simulink model "untitled"  (R2019a)
settings: Solver=VariableStepAuto  StartTime=0.0  StopTime=30.0  RelTol=1e-3
undefined symbols (not defined in the file or in its folder): qJoints_init, robot, sigbuilder_block
libraries: SPART_Lib x2, dspinverses x2, robotmaniplib x1
settings Model: Creator=tori  LastModifiedBy=tori
settings DataIOCC: ReturnWorkspaceOutputs=off
settings DebuggingCC: ArithmeticOperatorsInVariantConditions=warning
settings SFSimCC: SimUseLocalCustomCode=off
settings RTWCC: RTWUseLocalCustomCode=off

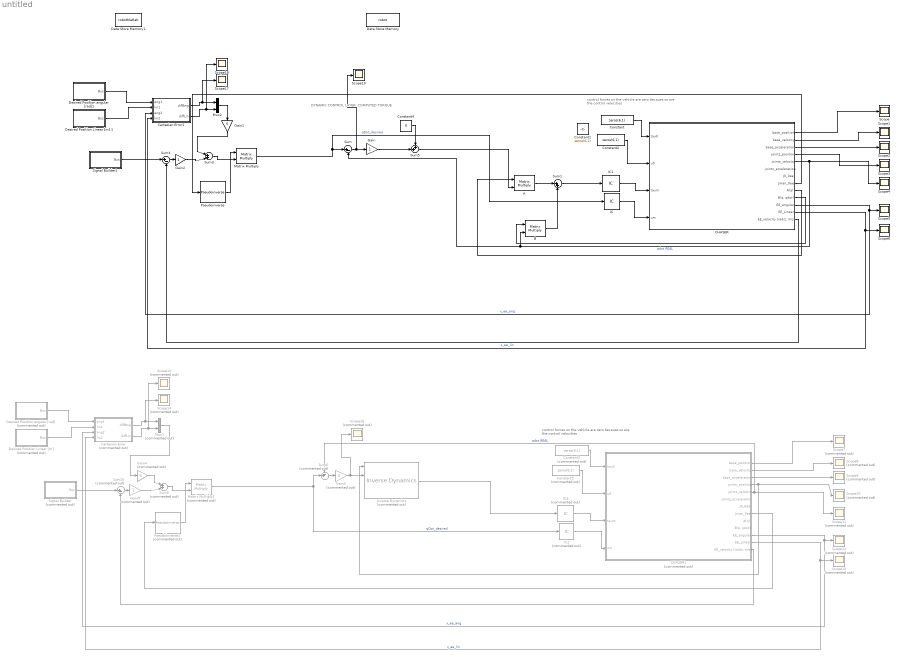
== system untitled ==
  note: DYNAMIC CONTROL LAYER: COMPUTED TORQUE
  note: control forces on the vehicle are zero
      | because so are the control velocities
  note: control forces on the vehicle are zero
      | because so are the control velocities
  A : Product  Multiplication=Matrix(*)
  B : Product  Multiplication=Matrix(*)
  CHASER : Subsystem
  CHASER1 : Subsystem  Commented=on
  Cartesian Error : MATLAB Function  Commented=on  TreatAsAtomicUnit=on
  Cartesian Error1 : MATLAB Function  TreatAsAtomicUnit=on
  Constant : Constant  Value=zeros(6,1)
  Constant1 : Constant  Value=zeros(6,1)
  Constant2 : Constant  Value=zeros(6,1)
  Constant3 : Constant  Commented=on  Value=zeros(6,1)
  Constant4 : Constant  Value=0
  Constant5 : Constant  Commented=on  Value=zeros(6,1)
  Data Store Memory : DataStoreMemory  DataStoreName=robot  ReadBeforeWriteMsg=warning  WriteAfterWriteMsg=warning  WriteAfterReadMsg=warning  ShowAdditionalParam=off
  Data Store Memory1 : DataStoreMemory  DataStoreName=robotMatlab  ReadBeforeWriteMsg=warning  WriteAfterWriteMsg=warning  WriteAfterReadMsg=warning  ShowAdditionalParam=off
  "Desired Position Linear [m] " : Subsystem  Tag=STV Subsys  Commented=on  LoadFcn=sigbuilder_block('load');  StartFcn=sigbuilder_block('start');  StopFcn=sigbuilder_block('stop');  ClipboardFcn=sigbuilder_block('clipboard');  mask(Sigbuilder block){tuvar=[0:10]}
      mask help: Simulink:masks:SigbuilderBlock_MD
      mask init:
      | if ~strcmp(get_param(bdroot(gcbh),'SimulationStatus'),'stopped') tuvar = sigbuilder_block('maskInit'); end
      settings: CopyFcn=sigbuilder_block('copy');  DeleteFcn=sigbuilder_block('delete');  ModelCloseFcn=sigbuilder_block('modelClose');  PreSaveFcn=sigbuilder_block('preSave');  PauseFcn=sigbuilder_block('pause');  ContinueFcn=sigbuilder_block('continue');  NameChangeFcn=sigbuilder_block('namechange');  OpenFcn=sigbuilder_block('open',[4.5 0 1432.5 645.75 ]);  CloseFcn=sigbuilder_block('close');
      mask Display: plot(0, 0, 100, 100,[2, 2, 32, 32, 2], [68, 8, 8, 68, 68],[32, 2], [38, 38], [32, 19, 2],[53, 60, 44], [32, 17, 17, 2],[16, 16, 31, 31]);txt = getActiveGroup(gcbh);text(2, 100, txt,'verticalAlignment', 'top');
  Desired Position Linear [m] 1 : Subsystem  Tag=STV Subsys  LoadFcn=sigbuilder_block('load');  StartFcn=sigbuilder_block('start');  StopFcn=sigbuilder_block('stop');  ClipboardFcn=sigbuilder_block('clipboard');  mask(Sigbuilder block){tuvar=[0:10]}
      mask help: Simulink:masks:SigbuilderBlock_MD
      mask init:
      | if ~strcmp(get_param(bdroot(gcbh),'SimulationStatus'),'stopped') tuvar = sigbuilder_block('maskInit'); end
      settings: CopyFcn=sigbuilder_block('copy');  DeleteFcn=sigbuilder_block('delete');  ModelCloseFcn=sigbuilder_block('modelClose');  PreSaveFcn=sigbuilder_block('preSave');  PauseFcn=sigbuilder_block('pause');  ContinueFcn=sigbuilder_block('continue');  NameChangeFcn=sigbuilder_block('namechange');  OpenFcn=sigbuilder_block('open',[4.5 0 1432.5 645.75 ]);  CloseFcn=sigbuilder_block('close');
      mask Display: plot(0, 0, 100, 100,[2, 2, 32, 32, 2], [68, 8, 8, 68, 68],[32, 2], [38, 38], [32, 19, 2],[53, 60, 44], [32, 17, 17, 2],[16, 16, 31, 31]);txt = getActiveGroup(gcbh);text(2, 100, txt,'verticalAlignment', 'top');
  Desired Position angular [rad] : Subsystem  Tag=STV Subsys  Commented=on  LoadFcn=sigbuilder_block('load');  StartFcn=sigbuilder_block('start');  StopFcn=sigbuilder_block('stop');  ClipboardFcn=sigbuilder_block('clipboard');  mask(Sigbuilder block){tuvar=[0:10]}
      mask help: Simulink:masks:SigbuilderBlock_MD
      mask init:
      | if ~strcmp(get_param(bdroot(gcbh),'SimulationStatus'),'stopped') tuvar = sigbuilder_block('maskInit'); end
      settings: CopyFcn=sigbuilder_block('copy');  DeleteFcn=sigbuilder_block('delete');  ModelCloseFcn=sigbuilder_block('modelClose');  PreSaveFcn=sigbuilder_block('preSave');  PauseFcn=sigbuilder_block('pause');  ContinueFcn=sigbuilder_block('continue');  NameChangeFcn=sigbuilder_block('namechange');  OpenFcn=sigbuilder_block('open',[0 0 1440 627 ]);  CloseFcn=sigbuilder_block('close');
      mask Display: plot(0, 0, 100, 100,[2, 2, 32, 32, 2], [68, 8, 8, 68, 68],[32, 2], [38, 38], [32, 19, 2],[53, 60, 44], [32, 17, 17, 2],[16, 16, 31, 31]);txt = getActiveGroup(gcbh);text(2, 100, txt,'verticalAlignment', 'top');
  Desired Position angular [rad]1 : Subsystem  Tag=STV Subsys  LoadFcn=sigbuilder_block('load');  StartFcn=sigbuilder_block('start');  StopFcn=sigbuilder_block('stop');  ClipboardFcn=sigbuilder_block('clipboard');  mask(Sigbuilder block){tuvar=[0:10]}
      mask help: Simulink:masks:SigbuilderBlock_MD
      mask init:
      | if ~strcmp(get_param(bdroot(gcbh),'SimulationStatus'),'stopped') tuvar = sigbuilder_block('maskInit'); end
      settings: CopyFcn=sigbuilder_block('copy');  DeleteFcn=sigbuilder_block('delete');  ModelCloseFcn=sigbuilder_block('modelClose');  PreSaveFcn=sigbuilder_block('preSave');  PauseFcn=sigbuilder_block('pause');  ContinueFcn=sigbuilder_block('continue');  NameChangeFcn=sigbuilder_block('namechange');  OpenFcn=sigbuilder_block('open',[0 0 1440 608.25 ]);  CloseFcn=sigbuilder_block('close');
      mask Display: plot(0, 0, 100, 100,[2, 2, 32, 32, 2], [68, 8, 8, 68, 68],[32, 2], [38, 38], [32, 19, 2],[53, 60, 44], [32, 17, 17, 2],[16, 16, 31, 31]);txt = getActiveGroup(gcbh);text(2, 100, txt,'verticalAlignment', 'top');
  Gain : Gain
  Gain1 : Gain  Gain=5
  Gain2 : Gain
  Gain3 : Gain  Commented=on  Gain=5
  Gain4 : Gain  Commented=on  Gain=3
  Gain5 : Gain  Commented=on
  IC : InitialCondition  Value=zeros(7,1)
  IC1 : InitialCondition  Value=zeros(7,1)
  IC2 : InitialCondition  Commented=on  Value=zeros(7,1)
  IC3 : InitialCondition  Commented=on  Value=zeros(7,1)
  Inverse Dynamics : robotmaniplib/Inverse Dynamics  Commented=on  RigidBodyTree=robotMatlab  SimulateUsing=Interpreted execution
      settings: SourceProductName=Robotics System Toolbox  SourceProductBaseCode=RO
  Matrix Multiply : Product  Multiplication=Matrix(*)
  Matrix Multiply1 : Product  Commented=on  Multiplication=Matrix(*)
  Mux1 : Mux  Commented=on  Inputs=2
  Mux2 : Mux  Inputs=2
  Pseudoinverse : dspinverses/Pseudoinverse  wanterr=off  SimulateUsing=Interpreted execution
      settings: SourceProductName=DSP System Toolbox  SourceProductBaseCode=DS
  Pseudoinverse1 : dspinverses/Pseudoinverse  Commented=on  wanterr=off  SimulateUsing=Interpreted execution
      settings: SourceProductName=DSP System Toolbox  SourceProductBaseCode=DS
  Scope{,1..6,17..19} (10 alike) : Scope
  Scope{7..16} (10 alike) : Scope  Commented=on
  Signal Builder : Subsystem  Tag=STV Subsys  Commented=on  LoadFcn=sigbuilder_block('load');  StartFcn=sigbuilder_block('start');  StopFcn=sigbuilder_block('stop');  ClipboardFcn=sigbuilder_block('clipboard');  mask(Sigbuilder block){tuvar=[0:10]}
      mask help: Simulink:masks:SigbuilderBlock_MD
      mask init:
      | if ~strcmp(get_param(bdroot(gcbh),'SimulationStatus'),'stopped') tuvar = sigbuilder_block('maskInit'); end
      settings: CopyFcn=sigbuilder_block('copy');  DeleteFcn=sigbuilder_block('delete');  ModelCloseFcn=sigbuilder_block('modelClose');  PreSaveFcn=sigbuilder_block('preSave');  PauseFcn=sigbuilder_block('pause');  ContinueFcn=sigbuilder_block('continue');  NameChangeFcn=sigbuilder_block('namechange');  OpenFcn=sigbuilder_block('open',[0.75 -1.5 735 724.5 ]);  CloseFcn=sigbuilder_block('close');
      mask Display: plot(0, 0, 100, 100,[2, 2, 32, 32, 2], [68, 8, 8, 68, 68],[32, 2], [38, 38], [32, 19, 2],[53, 60, 44], [32, 17, 17, 2],[16, 16, 31, 31]);txt = getActiveGroup(gcbh);text(2, 100, txt,'verticalAlignment', 'top');
  Signal Builder1 : Subsystem  Tag=STV Subsys  LoadFcn=sigbuilder_block('load');  StartFcn=sigbuilder_block('start');  StopFcn=sigbuilder_block('stop');  ClipboardFcn=sigbuilder_block('clipboard');  mask(Sigbuilder block){tuvar=[0:10]}
      mask help: Simulink:masks:SigbuilderBlock_MD
      mask init:
      | if ~strcmp(get_param(bdroot(gcbh),'SimulationStatus'),'stopped') tuvar = sigbuilder_block('maskInit'); end
      settings: CopyFcn=sigbuilder_block('copy');  DeleteFcn=sigbuilder_block('delete');  ModelCloseFcn=sigbuilder_block('modelClose');  PreSaveFcn=sigbuilder_block('preSave');  PauseFcn=sigbuilder_block('pause');  ContinueFcn=sigbuilder_block('continue');  NameChangeFcn=sigbuilder_block('namechange');  OpenFcn=sigbuilder_block('open',[8.25 0 720 724.5 ]);  CloseFcn=sigbuilder_block('close');
      mask Display: plot(0, 0, 100, 100,[2, 2, 32, 32, 2], [68, 8, 8, 68, 68],[32, 2], [38, 38], [32, 19, 2],[53, 60, 44], [32, 17, 17, 2],[16, 16, 31, 31]);txt = getActiveGroup(gcbh);text(2, 100, txt,'verticalAlignment', 'top');
  Sum : Sum  Inputs=|+-
  Sum1 : Sum  Inputs=|++
  Sum10 : Sum  Commented=on  Inputs=|+-
  Sum3 : Sum  Inputs=|++|
  Sum4 : Sum  Inputs=|+-
  Sum5 : Sum  Inputs=++|
  Sum6 : Sum  Commented=on  Inputs=-+|
  Sum9 : Sum  Commented=on  Inputs=|++|
  wires:
  Pseudoinverse/1 -> Matrix Multiply/1
  Gain/1 -> Sum5/2
  Matrix Multiply/1 -> IC/1, Sum/1  "qDot_desired"
  Sum/1 -> Scope19/1, Gain/1
  A/1 -> Sum1/1
  B/1 -> Sum1/2
  CHASER/5(joints_velocity) -> Scope4/1, Sum/2, B/2  "qdot REAL"
  CHASER/8(Jman_0ee) -> Pseudoinverse/1
  Sum1/1 -> IC1/1
  Constant/1 -> CHASER/1(tau0)
  Constant2/1 -> CHASER/2(u0)
  IC/1 -> CHASER/4(um)
  IC1/1 -> CHASER/3(taum)
  CHASER/10("B(q, qdot)") -> B/1
  CHASER/9(A(q)) -> A/1
  CHASER/1("base_position ") -> Scope/1
  CHASER/2("base_velocity ") -> Scope1/1
  CHASER/3(base_acceleration) -> Scope2/1
  CHASER/4(joints_position) -> Scope3/1
  CHASER/11("EE_angular ") -> Cartesian Error1/3(ang2), Scope5/1  "x_ee_ang"
  CHASER/12("EE_Linear ") -> Cartesian Error1/4(lin2), Scope6/1  "x_ee_lin"
  Sum3/1 -> Matrix Multiply/2
  Sum4/1 -> Gain2/1
  Gain2/1 -> Sum3/2
  Signal Builder1/1(Bus) -> Sum4/1
  CHASER/13(EE_velocity [rad/s; m/s]) -> Sum4/2
  Sum5/1 -> A/2
  Signal Builder/1(Bus) -> Sum10/1
  CHASER1/13(EE_velocity [rad/s; m/s]) -> Sum10/2
  CHASER1/12("EE_Linear ") -> Cartesian Error/4(lin2), Scope13/1  "x_ee_lin"
  Gain5/1 -> Sum9/2
  Matrix Multiply1/1 -> Sum6/2, IC2/1  "qDot_desired"
  CHASER1/3(base_acceleration) -> Scope9/1
  Gain4/1 -> Sum9/1
  CHASER1/4(joints_position) -> Inverse Dynamics/1, Scope10/1
  CHASER1/11("EE_angular ") -> Cartesian Error/3(ang2), Scope12/1  "x_ee_ang"
  Pseudoinverse1/1 -> Matrix Multiply1/1
  CHASER1/1("base_position ") -> Scope7/1
  Sum10/1 -> Gain5/1
  Sum9/1 -> Matrix Multiply1/2
  CHASER1/2("base_velocity ") -> Scope8/1
  Constant3/1 -> CHASER1/1(tau0)
  Constant5/1 -> CHASER1/2(u0)
  CHASER1/5(joints_velocity) -> Scope11/1, Sum6/1  "qdot REAL"
  CHASER1/8(Jman_0ee) -> Pseudoinverse1/1
  IC2/1 -> CHASER1/4(um)
  IC3/1 -> CHASER1/3(taum)
  Inverse Dynamics/1 -> IC3/1
  Desired Position angular [rad]/1(Bus) -> Cartesian Error/1(ang1)
  "Desired Position Linear [m] "/1(Bus) -> Cartesian Error/2(lin1)
  Cartesian Error/1(diffAng) -> Scope14/1, Mux1/1
  Cartesian Error/2(diffLin) -> Scope15/1, Mux1/2
  Mux1/1 -> Gain4/1
  Sum6/1 -> Gain3/1
  Gain3/1 -> Scope16/1, Inverse Dynamics/2
  Mux2/1 -> Gain1/1
  Cartesian Error1/2(diffLin) -> Scope18/1, Mux2/2
  Desired Position Linear [m] 1/1(Bus) -> Cartesian Error1/2(lin1)
  Cartesian Error1/1(diffAng) -> Scope17/1, Mux2/1
  Desired Position angular [rad]1/1(Bus) -> Cartesian Error1/1(ang1)
  Gain1/1 -> Sum3/1
  Constant4/1 -> Sum5/1

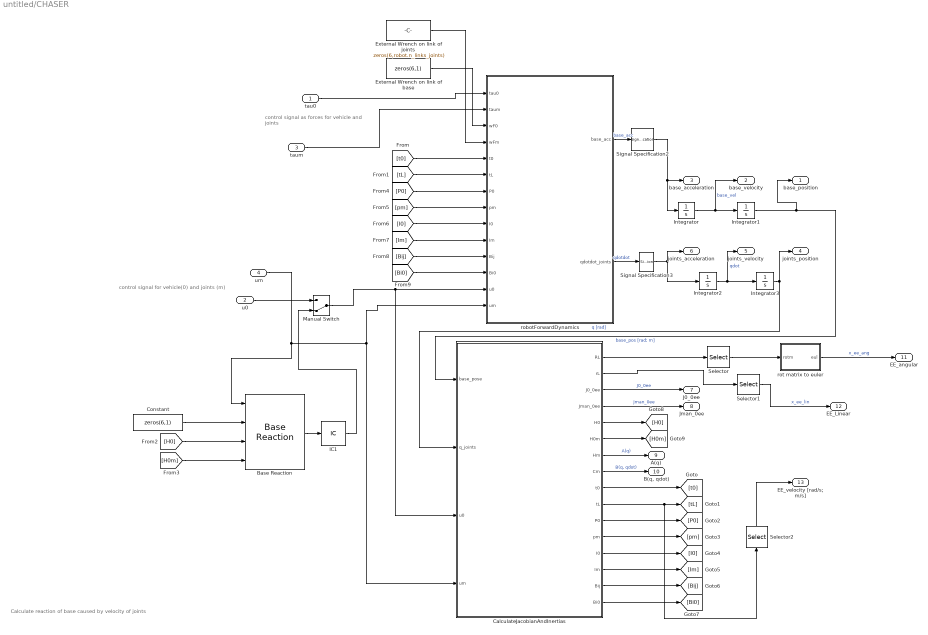
== system untitled/CHASER ==
  note: Calculate reaction of base caused by velocity of joints
  note: control signal as forces
      | for vehicle and joints
  note: control signal for vehicle(0)
      | and joints (m)
  tau0 : Inport
  u0 : Inport  Port=2
  taum : Inport  Port=3
  um : Inport  Port=4
  Base Reaction : SPART_Lib/Components/Base Reaction  SystemSampleTime=-1
  CalculateJacobianAndInertias : MATLAB Function  TreatAsAtomicUnit=on
  Constant : Constant  Value=zeros(6,1)
  "External Wrench on link of base " : Constant  Value=zeros(6,1)
  External Wrench on link of joints : Constant  Value=zeros(6,robot.n_links_joints)
  IC1 : InitialCondition  Value=zeros(6,1)
  Integrator : Integrator
  Integrator1 : Integrator
  Integrator2 : Integrator  InitialCondition=zeros(7,1)
  Integrator3 : Integrator  InitialCondition=qJoints_init  ContinuousStateAttributes='position'
  Manual Switch : ManualSwitch  CurrentSetting=0
  Selector : Selector  NumberOfDimensions=3  InputPortWidth=3  IndexOptions=Select all,Select all,Starting index (dialog)  Indices=[1 3],1,8  OutputSizes=1,1,1
  Selector1 : Selector  NumberOfDimensions=2  InputPortWidth=3  IndexOptions=Select all,Starting index (dialog)  Indices=[1 3],8  OutputSizes=1,1
  Selector2 : Selector  NumberOfDimensions=2  InputPortWidth=3  IndexOptions=Select all,Starting index (dialog)  Indices=[1 3],8  OutputSizes=1,1
  Signal Specification2 : SignalSpecification  Dimensions=[6 1]
  Signal Specification3 : SignalSpecification  Unit=rad  Dimensions=[7 1]
  "robotForwardDynamics " : MATLAB Function  TreatAsAtomicUnit=on
  "rot matrix to euler " : MATLAB Function  TreatAsAtomicUnit=on
  "base_position " : Outport
  "base_velocity " : Outport  Port=2
  base_acceleration : Outport  Port=3
  joints_position : Outport  Port=4
  joints_velocity : Outport  Port=5
  joints_acceleration : Outport  Port=6
  J0_0ee : Outport  Port=7
  Jman_0ee : Outport  Port=8
  A(q) : Outport  Port=9
  "B(q, qdot)" : Outport  Port=10
  "EE_angular " : Outport  Port=11
  "EE_Linear " : Outport  Port=12
  EE_velocity [rad/s; m/s] : Outport  Port=13
  wires:
  CalculateJacobianAndInertias/4(Jman_0ee) -> Jman_0ee/1  "Jman_0ee"
  CalculateJacobianAndInertias/7(Hm) -> A(q)/1  "A(q)"
  CalculateJacobianAndInertias/8(Cm) -> "B(q, qdot)"/1  "B(q, qdot)"
  "robotForwardDynamics "/1(base_acc) -> Signal Specification2/1  "base_acc"
  taum/1 -> "robotForwardDynamics "/2(taum)
  um/1 -> Base Reaction/1, "robotForwardDynamics "/14(um), CalculateJacobianAndInertias/4(um)
  tau0/1 -> "robotForwardDynamics "/1(tau0)
  CalculateJacobianAndInertias/3(J0_0ee) -> J0_0ee/1  "J0_0ee"
  Integrator/1 -> Integrator1/1, "base_velocity "/1  "base_vel"
  Integrator1/1 -> CalculateJacobianAndInertias/1(base_pose), "base_position "/1  "base_pos [rad; m]"
  Integrator2/1 -> joints_velocity/1, Integrator3/1  "qdot"
  Integrator3/1 -> CalculateJacobianAndInertias/2(q_joints), joints_position/1  "q [rad]"
  "robotForwardDynamics "/2(qdotdot_joints) -> Signal Specification3/1  "qdotdot"
  "External Wrench on link of base "/1 -> "robotForwardDynamics "/3(wF0)
  External Wrench on link of joints/1 -> "robotForwardDynamics "/4(wFm)
  [t0] -> "robotForwardDynamics "/5(t0)
  [tL] -> "robotForwardDynamics "/6(tL)
  [P0] -> "robotForwardDynamics "/7(P0)
  [pm] -> "robotForwardDynamics "/8(pm)
  [I0] -> "robotForwardDynamics "/9(I0)
  [Im] -> "robotForwardDynamics "/10(Im)
  [Bij] -> "robotForwardDynamics "/11(Bij)
  [Bi0] -> "robotForwardDynamics "/12(Bi0)
  CalculateJacobianAndInertias/9(t0) -> [t0]
  CalculateJacobianAndInertias/10(tL) -> Selector2/1, [tL]
  CalculateJacobianAndInertias/11(P0) -> [P0]
  CalculateJacobianAndInertias/12(pm) -> [pm]
  CalculateJacobianAndInertias/13(I0) -> [I0]
  CalculateJacobianAndInertias/14(Im) -> [Im]
  CalculateJacobianAndInertias/15(Bij) -> [Bij]
  CalculateJacobianAndInertias/16(Bi0) -> [Bi0]
  CalculateJacobianAndInertias/5(H0) -> [H0]
  CalculateJacobianAndInertias/6(H0m) -> [H0m]
  [H0] -> Base Reaction/3
  [H0m] -> Base Reaction/4
  CalculateJacobianAndInertias/1(RL) -> Selector/1
  CalculateJacobianAndInertias/2(rL) -> Selector1/1
  Selector/1 -> "rot matrix to euler "/1(rotm)
  "rot matrix to euler "/1(eul) -> "EE_angular "/1  "x_ee_ang"
  Selector1/1 -> "EE_Linear "/1  "x_ee_lin"
  Signal Specification3/1 -> Integrator2/1, joints_acceleration/1
  Signal Specification2/1 -> Integrator/1, base_acceleration/1
  Selector2/1 -> EE_velocity [rad/s; m/s]/1
  Constant/1 -> Base Reaction/2
  Base Reaction/1 -> IC1/1
  u0/1 -> Manual Switch/1
  Manual Switch/1 -> CalculateJacobianAndInertias/3(u0), "robotForwardDynamics "/13(u0)
  IC1/1 -> Manual Switch/2

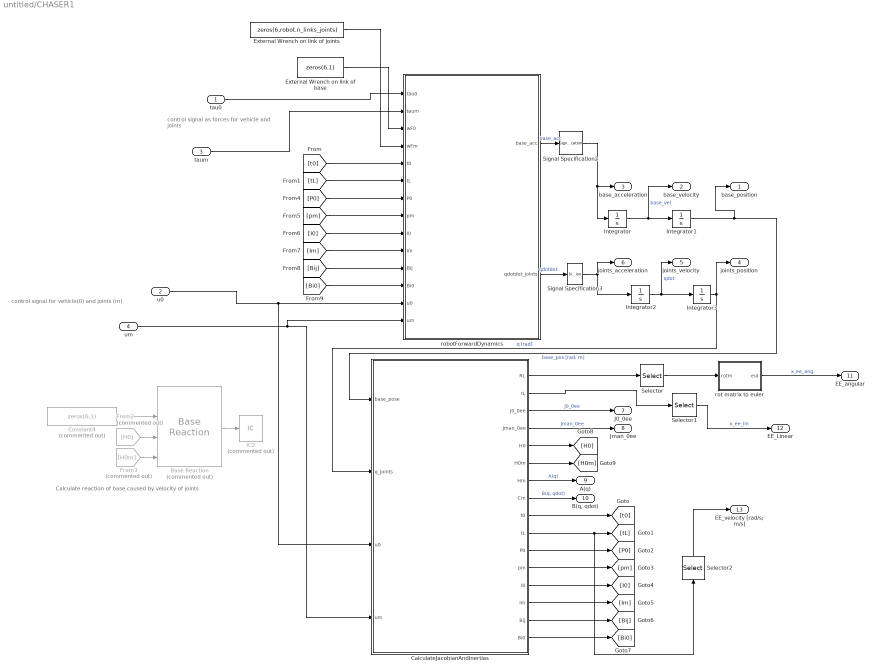
== system untitled/CHASER1 ==
  note: Calculate reaction of base caused by velocity of joints
  note: control signal as forces
      | for vehicle and joints
  note: control signal for vehicle(0)
      | and joints (m)
  tau0 : Inport
  u0 : Inport  Port=2
  taum : Inport  Port=3
  um : Inport  Port=4
  Base Reaction : SPART_Lib/Components/Base Reaction  Commented=on  SystemSampleTime=-1
  CalculateJacobianAndInertias : MATLAB Function  TreatAsAtomicUnit=on
  Constant4 : Constant  Commented=on  Value=zeros(6,1)
  "External Wrench on link of base " : Constant  Value=zeros(6,1)
  External Wrench on link of joints : Constant  Value=zeros(6,robot.n_links_joints)
  From2 : From  Commented=on  GotoTag=H0
  From3 : From  Commented=on  GotoTag=H0m
  IC2 : InitialCondition  Commented=on  Value=zeros(6,1)
  Integrator : Integrator
  Integrator1 : Integrator
  Integrator2 : Integrator  InitialCondition=zeros(7,1)
  Integrator3 : Integrator  InitialCondition=qJoints_init  ContinuousStateAttributes='position'
  Selector : Selector  NumberOfDimensions=3  InputPortWidth=3  IndexOptions=Select all,Select all,Starting index (dialog)  Indices=[1 3],1,8  OutputSizes=1,1,1
  Selector1 : Selector  NumberOfDimensions=2  InputPortWidth=3  IndexOptions=Select all,Starting index (dialog)  Indices=[1 3],8  OutputSizes=1,1
  Selector2 : Selector  NumberOfDimensions=2  InputPortWidth=3  IndexOptions=Select all,Starting index (dialog)  Indices=[1 3],8  OutputSizes=1,1
  Signal Specification2 : SignalSpecification  Dimensions=[6 1]
  Signal Specification3 : SignalSpecification  Unit=rad  Dimensions=[7 1]
  "robotForwardDynamics " : MATLAB Function  TreatAsAtomicUnit=on
  "rot matrix to euler " : MATLAB Function  TreatAsAtomicUnit=on
  "base_position " : Outport
  "base_velocity " : Outport  Port=2
  base_acceleration : Outport  Port=3
  joints_position : Outport  Port=4
  joints_velocity : Outport  Port=5
  joints_acceleration : Outport  Port=6
  J0_0ee : Outport  Port=7
  Jman_0ee : Outport  Port=8
  A(q) : Outport  Port=9
  "B(q, qdot)" : Outport  Port=10
  "EE_angular " : Outport  Port=11
  "EE_Linear " : Outport  Port=12
  EE_velocity [rad/s; m/s] : Outport  Port=13
  wires:
  CalculateJacobianAndInertias/4(Jman_0ee) -> Jman_0ee/1  "Jman_0ee"
  CalculateJacobianAndInertias/7(Hm) -> A(q)/1  "A(q)"
  CalculateJacobianAndInertias/8(Cm) -> "B(q, qdot)"/1  "B(q, qdot)"
  "robotForwardDynamics "/1(base_acc) -> Signal Specification2/1  "base_acc"
  taum/1 -> "robotForwardDynamics "/2(taum)
  um/1 -> CalculateJacobianAndInertias/4(um), "robotForwardDynamics "/14(um)
  tau0/1 -> "robotForwardDynamics "/1(tau0)
  CalculateJacobianAndInertias/3(J0_0ee) -> J0_0ee/1  "J0_0ee"
  Integrator/1 -> Integrator1/1, "base_velocity "/1  "base_vel"
  Integrator1/1 -> CalculateJacobianAndInertias/1(base_pose), "base_position "/1  "base_pos [rad; m]"
  Integrator2/1 -> joints_velocity/1, Integrator3/1  "qdot"
  Integrator3/1 -> CalculateJacobianAndInertias/2(q_joints), joints_position/1  "q [rad]"
  "robotForwardDynamics "/2(qdotdot_joints) -> Signal Specification3/1  "qdotdot"
  "External Wrench on link of base "/1 -> "robotForwardDynamics "/3(wF0)
  External Wrench on link of joints/1 -> "robotForwardDynamics "/4(wFm)
  [t0] -> "robotForwardDynamics "/5(t0)
  [tL] -> "robotForwardDynamics "/6(tL)
  [P0] -> "robotForwardDynamics "/7(P0)
  [pm] -> "robotForwardDynamics "/8(pm)
  [I0] -> "robotForwardDynamics "/9(I0)
  [Im] -> "robotForwardDynamics "/10(Im)
  [Bij] -> "robotForwardDynamics "/11(Bij)
  [Bi0] -> "robotForwardDynamics "/12(Bi0)
  CalculateJacobianAndInertias/9(t0) -> [t0]
  CalculateJacobianAndInertias/10(tL) -> Selector2/1, [tL]
  CalculateJacobianAndInertias/11(P0) -> [P0]
  CalculateJacobianAndInertias/12(pm) -> [pm]
  CalculateJacobianAndInertias/13(I0) -> [I0]
  CalculateJacobianAndInertias/14(Im) -> [Im]
  CalculateJacobianAndInertias/15(Bij) -> [Bij]
  CalculateJacobianAndInertias/16(Bi0) -> [Bi0]
  CalculateJacobianAndInertias/5(H0) -> [H0]
  CalculateJacobianAndInertias/6(H0m) -> [H0m]
  From2/1 -> Base Reaction/3
  From3/1 -> Base Reaction/4
  CalculateJacobianAndInertias/1(RL) -> Selector/1
  CalculateJacobianAndInertias/2(rL) -> Selector1/1
  Selector/1 -> "rot matrix to euler "/1(rotm)
  "rot matrix to euler "/1(eul) -> "EE_angular "/1  "x_ee_ang"
  Selector1/1 -> "EE_Linear "/1  "x_ee_lin"
  Signal Specification3/1 -> Integrator2/1, joints_acceleration/1
  Signal Specification2/1 -> Integrator/1, base_acceleration/1
  Selector2/1 -> EE_velocity [rad/s; m/s]/1
  Base Reaction/1 -> IC2/1
  Constant4/1 -> Base Reaction/2
  u0/1 -> CalculateJacobianAndInertias/3(u0), "robotForwardDynamics "/13(u0)

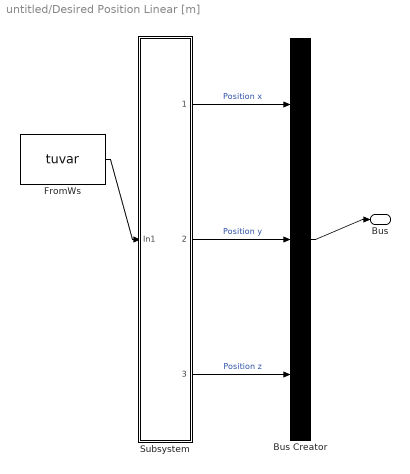
== system untitled/Desired Position Linear [m]  ==
  Bus Creator : BusCreator  Tag=Bus Creator  Inputs=3
  FromWs : FromWorkspace  Tag=STV FromWs  VariableName=tuvar  SampleTime=0
      SigBuilderData=|
      | common.afterFinalStr = 'Extrapolate'
      | common.sampleTime = 0
      | dataSet(1).timeRange = [0 30]
      | dataSet(1).name = 'Position'
      | dataSet(2).timeRange = [0 30]
      | dataSet(2).name = 'Position1'
      | sbobj.Groups(1).Name = 'Position'
      | sbobj.Groups(1).Signals(1).Name = 'Position x'
      | sbobj.Groups(1).Signals(1).XData = [0 0.15075 0.3015 0.45226 0.60301 0.75376 0.90451 1.0553 1.206 1.3568 1.5075 1.6583 1.809 1.9598 2.1105 2.2613 2.412 2.5628 2.7135 2.8643 3.015 3.1658 3.3165 3.4673 3.618 3.7688 3.9196 4.0703 4.2211 4.3718 4.5226 4.6733 4.8241 4.9748 5.1256 5.2763 5.4271 5.5778 5.7286 5.8793 6.0301 6.1808 6.3316 6.4823 6.6331 6.7838 6.9346 7.0853 7.2361 7.3869 7.5376 7.6884 7.8391 7.9899 8.1406 8.2914 8.4421 8.5929 8.7436 8.8944 9.0451 9.1959 9.3466 9.4974 9.6481 9.7989 9.9496 10.1 10.251 10.402 10.553 10.703 10.854 11.005 11.156 11.306 11.457 11.608 11.759 11.909 12.06 12.211 12.362 12.512 12.663 12.814 12.965 13.115 13.266 13.417 13.568 13.718 13.869 14.02 14.171 14.321 14.472 14.623 14.774 14.924 15.075 15.226 15.377 15.527 15.678 15.829 15.98 16.13 16.281 16.432 16.583 16.733 16.884 17.035 17.186 17.336 17.487 17.638 17.789 17.939 18.09 18.241 18.392 18.543 18.693 18.844 18.995 19.146 19.296 19.447 19.598 19.749 19.899 20.05 20.201 20.352 20.502 20.653 20.804 20.955 21.105 21.256 21.407 21.558 21.708 21.859 22.01 22.161 22.311 22.462 22.613 22.764 22.914 23.065 23.216 23.367 23.517 23.668 23.819 23.97 24.12 24.271 24.422 24.573 24.723 24.874 25.025 25.176 25.326 25.477 25.628 25.779 25.929 26.08 26.231 26.382 26.532 26.683 26.834 26.985 27.135 27.286 27.437 27.588 27.738 27.889 28.04 28.191 28.341 28.492 28.643 28.794 28.944 29.095 29.246 29.397 29.547 29.698 29.849 30]
      | sbobj.Groups(1).Signals(1).YData = [4.1497 4.1496 4.1494 4.149 4.1484 4.1474 4.1461 4.1445 4.1427 4.1405 4.1382 4.1356 4.1328 4.1298 4.1268 4.1236 4.1203 4.117 4.1136 4.1102 4.1067 4.1033 4.0999 4.0964 4.093 4.0896 4.0862 4.0828 4.0794 4.076 4.0726 4.0692 4.0657 4.0622 4.0586 4.055 4.0513 4.0476 4.0438 4.0399 4.0359 4.0318 4.0277 4.0235 4.0192 4.0148 4.0104 4.0058 4.0012 3.9966 3.9918 3.987 3.9822 3.9773 3.9723 3.9674 3.9623 3.9573 3.9522 3.9471 3.9419 3.9368 3.9316 3.9265 3.9213 3.9161 3.9109 3.9056 3.9004 3.8951 3.8899 3.8846 3.8793 3.8739 3.8686 3.8632 3.8578 3.8523 3.8468 3.8413 3.8357 3.83 3.8243 3.8186 3.8128 3.8069 3.801 3.795 3.7889 3.7828 3.7766 3.7704 3.7641 3.7578 3.7513 3.7449 3.7384 3.7318 3.7252 3.7186 3.7119 3.7052 3.6984 3.6917 3.6849 3.678 3.6712 3.6644 3.6575 3.6506 3.6438 3.6369 3.63 3.6231 3.6163 3.6094 3.6025 3.5956 3.5887 3.5818 3.5749 3.5679 3.561 3.554 3.547 3.54 3.533 3.5259 3.5188 3.5116 3.5044 3.4972 3.4899 3.4825 3.4751 3.4676 3.4601 3.4525 3.4449 3.4371 3.4294 3.4216 3.4137 3.4058 3.3978 3.3898 3.3818 3.3737 3.3656 3.3575 3.3494 3.3412 3.3331 3.325 3.3169 3.3088 3.3007 3.2927 3.2847 3.2767 3.2687 3.2608 3.253 3.2451 3.2373 3.2295 3.2217 3.2139 3.2061 3.1983 3.1905 3.1826 3.1747 3.1668 3.1587 3.1506 3.1424 3.1341 3.1258 3.1173 3.1087 3.1 3.0912 3.0824 3.0736 3.0647 3.0559 3.0471 3.0385 3.0301 3.022 3.0143 3.0071 3.0004 2.9944 2.9892 2.9849 2.9817 2.9797 2.979]
      | sbobj.Groups(1).Signals(2).Name = 'Position y'
      | sbobj.Groups(1).Signals(2).XData = [0 0.15075 0.3015 0.45226 0.60301 0.75376 0.90451 1.0553 1.206 1.3568 1.5075 1.6583 1.809 1.9598 2.1105 2.2613 2.412 2.5628 2.7135 2.8643 3.015 3.1658 3.3165 3.4673 3.618 3.7688 3.9196 4.0703 4.2211 4.3718 4.5226 4.6733 4.8241 4.9748 5.1256 5.2763 5.4271 5.5778 5.7286 5.8793 6.0301 6.1808 6.3316 6.4823 6.6331 6.7838 6.9346 7.0853 7.2361 7.3869 7.5376 7.6884 7.8391 7.9899 8.1406 8.2914 8.4421 8.5929 8.7436 8.8944 9.0451 9.1959 9.3466 9.4974 9.6481 9.7989 9.9496 10.1 10.251 10.402 10.553 10.703 10.854 11.005 11.156 11.306 11.457 11.608 11.759 11.909 12.06 12.211 12.362 12.512 12.663 12.814 12.965 13.115 13.266 13.417 13.568 13.718 13.869 14.02 14.171 14.321 14.472 14.623 14.774 14.924 15.075 15.226 15.377 15.527 15.678 15.829 15.98 16.13 16.281 16.432 16.583 16.733 16.884 17.035 17.186 17.336 17.487 17.638 17.789 17.939 18.09 18.241 18.392 18.543 18.693 18.844 18.995 19.146 19.296 19.447 19.598 19.749 19.899 20.05 20.201 20.352 20.502 20.653 20.804 20.955 21.105 21.256 21.407 21.558 21.708 21.859 22.01 22.161 22.311 22.462 22.613 22.764 22.914 23.065 23.216 23.367 23.517 23.668 23.819 23.97 24.12 24.271 24.422 24.573 24.723 24.874 25.025 25.176 25.326 25.477 25.628 25.779 25.929 26.08 26.231 26.382 26.532 26.683 26.834 26.985 27.135 27.286 27.437 27.588 27.738 27.889 28.04 28.191 28.341 28.492 28.643 28.794 28.944 29.095 29.246 29.397 29.547 29.698 29.849 30]
      | sbobj.Groups(1).Signals(2).YData = [0.16804 0.16819 0.16861 0.16923 0.17001 0.17093 0.17195 0.17305 0.1742 0.17541 0.17666 0.17793 0.17923 0.18054 0.18188 0.18322 0.18458 0.18595 0.18732 0.1887 0.19008 0.19147 0.19286 0.19425 0.19564 0.19703 0.19842 0.19981 0.2012 0.20259 0.20397 0.20535 0.20673 0.2081 0.20948 0.21085 0.21222 0.21359 0.21496 0.21632 0.21769 0.21906 0.22044 0.22181 0.22319 0.22458 0.22597 0.22738 0.22879 0.23021 0.23164 0.23309 0.23455 0.23602 0.23751 0.23902 0.24054 0.24207 0.24363 0.2452 0.24679 0.24839 0.25002 0.25166 0.25331 0.25498 0.25667 0.25837 0.26008 0.2618 0.26354 0.26528 0.26703 0.26879 0.27056 0.27233 0.27411 0.27589 0.27767 0.27945 0.28123 0.283 0.28478 0.28655 0.28832 0.29008 0.29184 0.2936 0.29535 0.2971 0.29884 0.30058 0.30231 0.30404 0.30577 0.30749 0.30922 0.31095 0.31268 0.31441 0.31614 0.31789 0.31963 0.32139 0.32316 0.32494 0.32673 0.32854 0.33036 0.3322 0.33405 0.33592 0.33782 0.33973 0.34166 0.34361 0.34558 0.34758 0.34959 0.35162 0.35367 0.35574 0.35782 0.35992 0.36204 0.36416 0.3663 0.36845 0.3706 0.37276 0.37493 0.37709 0.37926 0.38142 0.38358 0.38573 0.38788 0.39002 0.39214 0.39426 0.39636 0.39845 0.40052 0.40259 0.40464 0.40667 0.4087 0.41071 0.41272 0.41471 0.41671 0.4187 0.42069 0.42268 0.42468 0.42668 0.4287 0.43074 0.43279 0.43487 0.43697 0.43911 0.44128 0.44348 0.44572 0.44801 0.45033 0.4527 0.45511 0.45757 0.46008 0.46262 0.46521 0.46784 0.47051 0.47321 0.47593 0.47868 0.48145 0.48422 0.48701 0.48978 0.49255 0.49529 0.49801 0.50068 0.5033 0.50586 0.50835 0.51074 0.51304 0.51521 0.51725 0.51912 0.52082 0.5223 0.52353 0.52447 0.52508 0.52529]
      | sbobj.Groups(1).Signals(3).Name = 'Position z'
      | sbobj.Groups(1).Signals(3).XData = [0 0.15075 0.3015 0.45226 0.60301 0.75376 0.90451 1.0553 1.206 1.3568 1.5075 1.6583 1.809 1.9598 2.1105 2.2613 2.412 2.5628 2.7135 2.8643 3.015 3.1658 3.3165 3.4673 3.618 3.7688 3.9196 4.0703 4.2211 4.3718 4.5226 4.6733 4.8241 4.9748 5.1256 5.2763 5.4271 5.5778 5.7286 5.8793 6.0301 6.1808 6.3316 6.4823 6.6331 6.7838 6.9346 7.0853 7.2361 7.3869 7.5376 7.6884 7.8391 7.9899 8.1406 8.2914 8.4421 8.5929 8.7436 8.8944 9.0451 9.1959 9.3466 9.4974 9.6481 9.7989 9.9496 10.1 10.251 10.402 10.553 10.703 10.854 11.005 11.156 11.306 11.457 11.608 11.759 11.909 12.06 12.211 12.362 12.512 12.663 12.814 12.965 13.115 13.266 13.417 13.568 13.718 13.869 14.02 14.171 14.321 14.472 14.623 14.774 14.924 15.075 15.226 15.377 15.527 15.678 15.829 15.98 16.13 16.281 16.432 16.583 16.733 16.884 17.035 17.186 17.336 17.487 17.638 17.789 17.939 18.09 18.241 18.392 18.543 18.693 18.844 18.995 19.146 19.296 19.447 19.598 19.749 19.899 20.05 20.201 20.352 20.502 20.653 20.804 20.955 21.105 21.256 21.407 21.558 21.708 21.859 22.01 22.161 22.311 22.462 22.613 22.764 22.914 23.065 23.216 23.367 23.517 23.668 23.819 23.97 24.12 24.271 24.422 24.573 24.723 24.874 25.025 25.176 25.326 25.477 25.628 25.779 25.929 26.08 26.231 26.382 26.532 26.683 26.834 26.985 27.135 27.286 27.437 27.588 27.738 27.889 28.04 28.191 28.341 28.492 28.643 28.794 28.944 29.095 29.246 29.397 29.547 29.698 29.849 30]
      | sbobj.Groups(1).Signals(3).YData = [1.735 1.7355 1.737 1.7396 1.7435 1.7485 1.7547 1.7619 1.7701 1.7791 1.7889 1.7992 1.81 1.8211 1.8325 1.844 1.8557 1.8673 1.8789 1.8904 1.9017 1.9129 1.924 1.9348 1.9455 1.9559 1.9662 1.9764 1.9863 1.9962 2.0059 2.0155 2.0251 2.0346 2.044 2.0535 2.0629 2.0723 2.0817 2.0912 2.1007 2.1102 2.1198 2.1294 2.1391 2.1488 2.1585 2.1682 2.178 2.1878 2.1976 2.2074 2.2171 2.2269 2.2366 2.2463 2.2559 2.2655 2.275 2.2845 2.2939 2.3032 2.3124 2.3215 2.3306 2.3395 2.3484 2.3572 2.3659 2.3746 2.3831 2.3916 2.4 2.4083 2.4166 2.4248 2.4329 2.441 2.4491 2.4571 2.4651 2.4731 2.481 2.4889 2.4968 2.5047 2.5126 2.5204 2.5283 2.5361 2.5439 2.5518 2.5596 2.5674 2.5751 2.5829 2.5906 2.5983 2.606 2.6137 2.6213 2.6289 2.6364 2.6439 2.6513 2.6587 2.666 2.6733 2.6804 2.6876 2.6946 2.7016 2.7085 2.7153 2.722 2.7287 2.7353 2.7418 2.7483 2.7546 2.7609 2.7672 2.7733 2.7794 2.7855 2.7915 2.7974 2.8033 2.8091 2.815 2.8207 2.8265 2.8322 2.8379 2.8435 2.8492 2.8548 2.8604 2.866 2.8715 2.8771 2.8826 2.8881 2.8936 2.899 2.9045 2.9099 2.9152 2.9206 2.9258 2.9311 2.9362 2.9414 2.9464 2.9514 2.9563 2.9611 2.9659 2.9705 2.9751 2.9796 2.984 2.9883 2.9925 2.9966 3.0006 3.0045 3.0084 3.0122 3.0159 3.0195 3.0231 3.0266 3.0301 3.0336 3.037 3.0404 3.0438 3.0472 3.0506 3.054 3.0573 3.0607 3.0641 3.0674 3.0707 3.0739 3.0771 3.0802 3.0832 3.086 3.0887 3.0911 3.0934 3.0953 3.097 3.0983 3.0992 3.0998 3.1]
      | sbobj.Groups(1).TimeRange = [0 30]
      | sbobj.Groups(2).Name = 'Position1'
      | sbobj.Groups(2).Signals(1).Name = 'Position x'
      | sbobj.Groups(2).Signals(1).XData = [0 0.15075 0.3015 0.45226 0.60301 0.75376 0.90451 1.0553 1.206 1.3568 1.5075 1.6583 1.809 1.9598 2.1105 2.2613 2.412 2.5628 2.7135 2.8643 3.015 3.1658 3.3165 3.4673 3.618 3.7688 3.9196 4.0703 4.2211 4.3718 4.5226 4.6733 4.8241 4.9748 5.1256 5.2763 5.4271 5.5778 5.7286 5.8793 6.0301 6.1808 6.3316 6.4823 6.6331 6.7838 6.9346 7.0853 7.2361 7.3869 7.5376 7.6884 7.8391 7.9899 8.1406 8.2914 8.4421 8.5929 8.7436 8.8944 9.0451 9.1959 9.3466 9.4974 9.6481 9.7989 9.9496 10.1 10.251 10.402 10.553 10.703 10.854 11.005 11.156 11.306 11.457 11.608 11.759 11.909 12.06 12.211 12.362 12.512 12.663 12.814 12.965 13.115 13.266 13.417 13.568 13.718 13.869 14.02 14.171 14.321 14.472 14.623 14.774 14.924 15.075 15.226 15.377 15.527 15.678 15.829 15.98 16.13 16.281 16.432 16.583 16.733 16.884 17.035 17.186 17.336 17.487 17.638 17.789 17.939 18.09 18.241 18.392 18.543 18.693 18.844 18.995 19.146 19.296 19.447 19.598 19.749 19.899 20.05 20.201 20.352 20.502 20.653 20.804 20.955 21.105 21.256 21.407 21.558 21.708 21.859 22.01 22.161 22.311 22.462 22.613 22.764 22.914 23.065 23.216 23.367 23.517 23.668 23.819 23.97 24.12 24.271 24.422 24.573 24.723 24.874 25.025 25.176 25.326 25.477 25.628 25.779 25.929 26.08 26.231 26.382 26.532 26.683 26.834 26.985 27.135 27.286 27.437 27.588 27.738 27.889 28.04 28.191 28.341 28.492 28.643 28.794 28.944 29.095 29.246 29.397 29.547 29.698 29.849 30]
      | sbobj.Groups(2).Signals(1).YData = [4.1497 4.1496 4.1494 4.149 4.1484 4.1474 4.1461 4.1445 4.1427 4.1405 4.1382 4.1356 4.1328 4.1298 4.1268 4.1236 4.1203 4.117 4.1136 4.1102 4.1067 4.1033 4.0999 4.0964 4.093 4.0896 4.0862 4.0828 4.0794 4.076 4.0726 4.0692 4.0657 4.0622 4.0586 4.055 4.0513 4.0476 4.0438 4.0399 4.0359 4.0318 4.0277 4.0235 4.0192 4.0148 4.0104 4.0058 4.0012 3.9966 3.9918 3.987 3.9822 3.9773 3.9723 3.9674 3.9623 3.9573 3.9522 3.9471 3.9419 3.9368 3.9316 3.9265 3.9213 3.9161 3.9109 3.9056 3.9004 3.8951 3.8899 3.8846 3.8793 3.8739 3.8686 3.8632 3.8578 3.8523 3.8468 3.8413 3.8357 3.83 3.8243 3.8186 3.8128 3.8069 3.801 3.795 3.7889 3.7828 3.7766 3.7704 3.7641 3.7578 3.7513 3.7449 3.7384 3.7318 3.7252 3.7186 3.7119 3.7052 3.6984 3.6917 3.6849 3.678 3.6712 3.6644 3.6575 3.6506 3.6438 3.6369 3.63 3.6231 3.6163 3.6094 3.6025 3.5956 3.5887 3.5818 3.5749 3.5679 3.561 3.554 3.547 3.54 3.533 3.5259 3.5188 3.5116 3.5044 3.4972 3.4899 3.4825 3.4751 3.4676 3.4601 3.4525 3.4449 3.4371 3.4294 3.4216 3.4137 3.4058 3.3978 3.3898 3.3818 3.3737 3.3656 3.3575 3.3494 3.3412 3.3331 3.325 3.3169 3.3088 3.3007 3.2927 3.2847 3.2767 3.2687 3.2608 3.253 3.2451 3.2373 3.2295 3.2217 3.2139 3.2061 3.1983 3.1905 3.1826 3.1747 3.1668 3.1587 3.1506 3.1424 3.1341 3.1258 3.1173 3.1087 3.1 3.0912 3.0824 3.0736 3.0647 3.0559 3.0471 3.0385 3.0301 3.022 3.0143 3.0071 3.0004 2.9944 2.9892 2.9849 2.9817 2.9797 2.979]
      | sbobj.Groups(2).Signals(2).Name = 'Position y'
      | sbobj.Groups(2).Signals(2).XData = [0 0.15075 0.3015 0.45226 0.60301 0.75376 0.90451 1.0553 1.206 1.3568 1.5075 1.6583 1.809 1.9598 2.1105 2.2613 2.412 2.5628 2.7135 2.8643 3.015 3.1658 3.3165 3.4673 3.618 3.7688 3.9196 4.0703 4.2211 4.3718 4.5226 4.6733 4.8241 4.9748 5.1256 5.2763 5.4271 5.5778 5.7286 5.8793 6.0301 6.1808 6.3316 6.4823 6.6331 6.7838 6.9346 7.0853 7.2361 7.3869 7.5376 7.6884 7.8391 7.9899 8.1406 8.2914 8.4421 8.5929 8.7436 8.8944 9.0451 9.1959 9.3466 9.4974 9.6481 9.7989 9.9496 10.1 10.251 10.402 10.553 10.703 10.854 11.005 11.156 11.306 11.457 11.608 11.759 11.909 12.06 12.211 12.362 12.512 12.663 12.814 12.965 13.115 13.266 13.417 13.568 13.718 13.869 14.02 14.171 14.321 14.472 14.623 14.774 14.924 15.075 15.226 15.377 15.527 15.678 15.829 15.98 16.13 16.281 16.432 16.583 16.733 16.884 17.035 17.186 17.336 17.487 17.638 17.789 17.939 18.09 18.241 18.392 18.543 18.693 18.844 18.995 19.146 19.296 19.447 19.598 19.749 19.899 20.05 20.201 20.352 20.502 20.653 20.804 20.955 21.105 21.256 21.407 21.558 21.708 21.859 22.01 22.161 22.311 22.462 22.613 22.764 22.914 23.065 23.216 23.367 23.517 23.668 23.819 23.97 24.12 24.271 24.422 24.573 24.723 24.874 25.025 25.176 25.326 25.477 25.628 25.779 25.929 26.08 26.231 26.382 26.532 26.683 26.834 26.985 27.135 27.286 27.437 27.588 27.738 27.889 28.04 28.191 28.341 28.492 28.643 28.794 28.944 29.095 29.246 29.397 29.547 29.698 29.849 30]
      | sbobj.Groups(2).Signals(2).YData = [0.16804 0.16819 0.16861 0.16923 0.17001 0.17093 0.17195 0.17305 0.1742 0.17541 0.17666 0.17793 0.17923 0.18054 0.18188 0.18322 0.18458 0.18595 0.18732 0.1887 0.19008 0.19147 0.19286 0.19425 0.19564 0.19703 0.19842 0.19981 0.2012 0.20259 0.20397 0.20535 0.20673 0.2081 0.20948 0.21085 0.21222 0.21359 0.21496 0.21632 0.21769 0.21906 0.22044 0.22181 0.22319 0.22458 0.22597 0.22738 0.22879 0.23021 0.23164 0.23309 0.23455 0.23602 0.23751 0.23902 0.24054 0.24207 0.24363 0.2452 0.24679 0.24839 0.25002 0.25166 0.25331 0.25498 0.25667 0.25837 0.26008 0.2618 0.26354 0.26528 0.26703 0.26879 0.27056 0.27233 0.27411 0.27589 0.27767 0.27945 0.28123 0.283 0.28478 0.28655 0.28832 0.29008 0.29184 0.2936 0.29535 0.2971 0.29884 0.30058 0.30231 0.30404 0.30577 0.30749 0.30922 0.31095 0.31268 0.31441 0.31614 0.31789 0.31963 0.32139 0.32316 0.32494 0.32673 0.32854 0.33036 0.3322 0.33405 0.33592 0.33782 0.33973 0.34166 0.34361 0.34558 0.34758 0.34959 0.35162 0.35367 0.35574 0.35782 0.35992 0.36204 0.36416 0.3663 0.36845 0.3706 0.37276 0.37493 0.37709 0.37926 0.38142 0.38358 0.38573 0.38788 0.39002 0.39214 0.39426 0.39636 0.39845 0.40052 0.40259 0.40464 0.40667 0.4087 0.41071 0.41272 0.41471 0.41671 0.4187 0.42069 0.42268 0.42468 0.42668 0.4287 0.43074 0.43279 0.43487 0.43697 0.43911 0.44128 0.44348 0.44572 0.44801 0.45033 0.4527 0.45511 0.45757 0.46008 0.46262 0.46521 0.46784 0.47051 0.47321 0.47593 0.47868 0.48145 0.48422 0.48701 0.48978 0.49255 0.49529 0.49801 0.50068 0.5033 0.50586 0.50835 0.51074 0.51304 0.51521 0.51725 0.51912 0.52082 0.5223 0.52353 0.52447 0.52508 0.52529]
      | sbobj.Groups(2).Signals(3).Name = 'Position z'
      | sbobj.Groups(2).Signals(3).XData = [0 0.15075 0.3015 0.45226 0.60301 0.75376 0.90451 1.0553 1.206 1.3568 1.5075 1.6583 1.809 1.9598 2.1105 2.2613 2.412 2.5628 2.7135 2.8643 3.015 3.1658 3.3165 3.4673 3.618 3.7688 3.9196 4.0703 4.2211 4.3718 4.5226 4.6733 4.8241 4.9748 5.1256 5.2763 5.4271 5.5778 5.7286 5.8793 6.0301 6.1808 6.3316 6.4823 6.6331 6.7838 6.9346 7.0853 7.2361 7.3869 7.5376 7.6884 7.8391 7.9899 8.1406 8.2914 8.4421 8.5929 8.7436 8.8944 9.0451 9.1959 9.3466 9.4974 9.6481 9.7989 9.9496 10.1 10.251 10.402 10.553 10.703 10.854 11.005 11.156 11.306 11.457 11.608 11.759 11.909 12.06 12.211 12.362 12.512 12.663 12.814 12.965 13.115 13.266 13.417 13.568 13.718 13.869 14.02 14.171 14.321 14.472 14.623 14.774 14.924 15.075 15.226 15.377 15.527 15.678 15.829 15.98 16.13 16.281 16.432 16.583 16.733 16.884 17.035 17.186 17.336 17.487 17.638 17.789 17.939 18.09 18.241 18.392 18.543 18.693 18.844 18.995 19.146 19.296 19.447 19.598 19.749 19.899 20.05 20.201 20.352 20.502 20.653 20.804 20.955 21.105 21.256 21.407 21.558 21.708 21.859 22.01 22.161 22.311 22.462 22.613 22.764 22.914 23.065 23.216 23.367 23.517 23.668 23.819 23.97 24.12 24.271 24.422 24.573 24.723 24.874 25.025 25.176 25.326 25.477 25.628 25.779 25.929 26.08 26.231 26.382 26.532 26.683 26.834 26.985 27.135 27.286 27.437 27.588 27.738 27.889 28.04 28.191 28.341 28.492 28.643 28.794 28.944 29.095 29.246 29.397 29.547 29.698 29.849 30]
      | sbobj.Groups(2).Signals(3).YData = [1.735 1.7355 1.737 1.7396 1.7435 1.7485 1.7547 1.7619 1.7701 1.7791 1.7889 1.7992 1.81 1.8211 1.8325 1.844 1.8557 1.8673 1.8789 1.8904 1.9017 1.9129 1.924 1.9348 1.9455 1.9559 1.9662 1.9764 1.9863 1.9962 2.0059 2.0155 2.0251 2.0346 2.044 2.0535 2.0629 2.0723 2.0817 2.0912 2.1007 2.1102 2.1198 2.1294 2.1391 2.1488 2.1585 2.1682 2.178 2.1878 2.1976 2.2074 2.2171 2.2269 2.2366 2.2463 2.2559 2.2655 2.275 2.2845 2.2939 2.3032 2.3124 2.3215 2.3306 2.3395 2.3484 2.3572 2.3659 2.3746 2.3831 2.3916 2.4 2.4083 2.4166 2.4248 2.4329 2.441 2.4491 2.4571 2.4651 2.4731 2.481 2.4889 2.4968 2.5047 2.5126 2.5204 2.5283 2.5361 2.5439 2.5518 2.5596 2.5674 2.5751 2.5829 2.5906 2.5983 2.606 2.6137 2.6213 2.6289 2.6364 2.6439 2.6513 2.6587 2.666 2.6733 2.6804 2.6876 2.6946 2.7016 2.7085 2.7153 2.722 2.7287 2.7353 2.7418 2.7483 2.7546 2.7609 2.7672 2.7733 2.7794 2.7855 2.7915 2.7974 2.8033 2.8091 2.815 2.8207 2.8265 2.8322 2.8379 2.8435 2.8492 2.8548 2.8604 2.866 2.8715 2.8771 2.8826 2.8881 2.8936 2.899 2.9045 2.9099 2.9152 2.9206 2.9258 2.9311 2.9362 2.9414 2.9464 2.9514 2.9563 2.9611 2.9659 2.9705 2.9751 2.9796 2.984 2.9883 2.9925 2.9966 3.0006 3.0045 3.0084 3.0122 3.0159 3.0195 3.0231 3.0266 3.0301 3.0336 3.037 3.0404 3.0438 3.0472 3.0506 3.054 3.0573 3.0607 3.0641 3.0674 3.0707 3.0739 3.0771 3.0802 3.0832 3.086 3.0887 3.0911 3.0934 3.0953 3.097 3.0983 3.0992 3.0998 3.1]
      | sbobj.Groups(2).TimeRange = [0 30]
  Subsystem : Subsystem
  Bus : Outport
  wires:
  FromWs/1 -> Subsystem/1(In1)
  Bus Creator/1 -> Bus/1
  Subsystem/1(Position x) -> Bus Creator/1  "Position x"
  Subsystem/2(Position y) -> Bus Creator/2  "Position y"
  Subsystem/3(Position z) -> Bus Creator/3  "Position z"

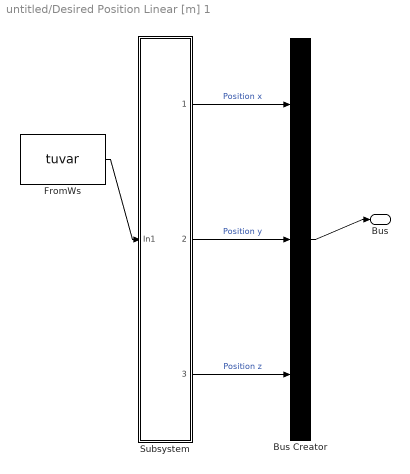
== system untitled/Desired Position Linear [m] 1 ==
  Bus Creator : BusCreator  Tag=Bus Creator  Inputs=3
  FromWs : FromWorkspace  Tag=STV FromWs  VariableName=tuvar  SampleTime=0
      SigBuilderData=|
      | common.afterFinalStr = 'Extrapolate'
      | common.sampleTime = 0
      | dataSet(1).timeRange = [0 30]
      | dataSet(1).name = 'Position'
      | dataSet(2).timeRange = [0 30]
      | dataSet(2).name = 'Position1'
      | sbobj.Groups(1).Name = 'Position'
      | sbobj.Groups(1).Signals(1).Name = 'Position x'
      | sbobj.Groups(1).Signals(1).XData = [0 0.15075 0.3015 0.45226 0.60301 0.75376 0.90451 1.0553 1.206 1.3568 1.5075 1.6583 1.809 1.9598 2.1105 2.2613 2.412 2.5628 2.7135 2.8643 3.015 3.1658 3.3165 3.4673 3.618 3.7688 3.9196 4.0703 4.2211 4.3718 4.5226 4.6733 4.8241 4.9748 5.1256 5.2763 5.4271 5.5778 5.7286 5.8793 6.0301 6.1808 6.3316 6.4823 6.6331 6.7838 6.9346 7.0853 7.2361 7.3869 7.5376 7.6884 7.8391 7.9899 8.1406 8.2914 8.4421 8.5929 8.7436 8.8944 9.0451 9.1959 9.3466 9.4974 9.6481 9.7989 9.9496 10.1 10.251 10.402 10.553 10.703 10.854 11.005 11.156 11.306 11.457 11.608 11.759 11.909 12.06 12.211 12.362 12.512 12.663 12.814 12.965 13.115 13.266 13.417 13.568 13.718 13.869 14.02 14.171 14.321 14.472 14.623 14.774 14.924 15.075 15.226 15.377 15.527 15.678 15.829 15.98 16.13 16.281 16.432 16.583 16.733 16.884 17.035 17.186 17.336 17.487 17.638 17.789 17.939 18.09 18.241 18.392 18.543 18.693 18.844 18.995 19.146 19.296 19.447 19.598 19.749 19.899 20.05 20.201 20.352 20.502 20.653 20.804 20.955 21.105 21.256 21.407 21.558 21.708 21.859 22.01 22.161 22.311 22.462 22.613 22.764 22.914 23.065 23.216 23.367 23.517 23.668 23.819 23.97 24.12 24.271 24.422 24.573 24.723 24.874 25.025 25.176 25.326 25.477 25.628 25.779 25.929 26.08 26.231 26.382 26.532 26.683 26.834 26.985 27.135 27.286 27.437 27.588 27.738 27.889 28.04 28.191 28.341 28.492 28.643 28.794 28.944 29.095 29.246 29.397 29.547 29.698 29.849 30]
      | sbobj.Groups(1).Signals(1).YData = [4.1497 4.1496 4.1494 4.149 4.1484 4.1474 4.1461 4.1445 4.1427 4.1405 4.1382 4.1356 4.1328 4.1298 4.1268 4.1236 4.1203 4.117 4.1136 4.1102 4.1067 4.1033 4.0999 4.0964 4.093 4.0896 4.0862 4.0828 4.0794 4.076 4.0726 4.0692 4.0657 4.0622 4.0586 4.055 4.0513 4.0476 4.0438 4.0399 4.0359 4.0318 4.0277 4.0235 4.0192 4.0148 4.0104 4.0058 4.0012 3.9966 3.9918 3.987 3.9822 3.9773 3.9723 3.9674 3.9623 3.9573 3.9522 3.9471 3.9419 3.9368 3.9316 3.9265 3.9213 3.9161 3.9109 3.9056 3.9004 3.8951 3.8899 3.8846 3.8793 3.8739 3.8686 3.8632 3.8578 3.8523 3.8468 3.8413 3.8357 3.83 3.8243 3.8186 3.8128 3.8069 3.801 3.795 3.7889 3.7828 3.7766 3.7704 3.7641 3.7578 3.7513 3.7449 3.7384 3.7318 3.7252 3.7186 3.7119 3.7052 3.6984 3.6917 3.6849 3.678 3.6712 3.6644 3.6575 3.6506 3.6438 3.6369 3.63 3.6231 3.6163 3.6094 3.6025 3.5956 3.5887 3.5818 3.5749 3.5679 3.561 3.554 3.547 3.54 3.533 3.5259 3.5188 3.5116 3.5044 3.4972 3.4899 3.4825 3.4751 3.4676 3.4601 3.4525 3.4449 3.4371 3.4294 3.4216 3.4137 3.4058 3.3978 3.3898 3.3818 3.3737 3.3656 3.3575 3.3494 3.3412 3.3331 3.325 3.3169 3.3088 3.3007 3.2927 3.2847 3.2767 3.2687 3.2608 3.253 3.2451 3.2373 3.2295 3.2217 3.2139 3.2061 3.1983 3.1905 3.1826 3.1747 3.1668 3.1587 3.1506 3.1424 3.1341 3.1258 3.1173 3.1087 3.1 3.0912 3.0824 3.0736 3.0647 3.0559 3.0471 3.0385 3.0301 3.022 3.0143 3.0071 3.0004 2.9944 2.9892 2.9849 2.9817 2.9797 2.979]
      | sbobj.Groups(1).Signals(2).Name = 'Position y'
      | sbobj.Groups(1).Signals(2).XData = [0 0.15075 0.3015 0.45226 0.60301 0.75376 0.90451 1.0553 1.206 1.3568 1.5075 1.6583 1.809 1.9598 2.1105 2.2613 2.412 2.5628 2.7135 2.8643 3.015 3.1658 3.3165 3.4673 3.618 3.7688 3.9196 4.0703 4.2211 4.3718 4.5226 4.6733 4.8241 4.9748 5.1256 5.2763 5.4271 5.5778 5.7286 5.8793 6.0301 6.1808 6.3316 6.4823 6.6331 6.7838 6.9346 7.0853 7.2361 7.3869 7.5376 7.6884 7.8391 7.9899 8.1406 8.2914 8.4421 8.5929 8.7436 8.8944 9.0451 9.1959 9.3466 9.4974 9.6481 9.7989 9.9496 10.1 10.251 10.402 10.553 10.703 10.854 11.005 11.156 11.306 11.457 11.608 11.759 11.909 12.06 12.211 12.362 12.512 12.663 12.814 12.965 13.115 13.266 13.417 13.568 13.718 13.869 14.02 14.171 14.321 14.472 14.623 14.774 14.924 15.075 15.226 15.377 15.527 15.678 15.829 15.98 16.13 16.281 16.432 16.583 16.733 16.884 17.035 17.186 17.336 17.487 17.638 17.789 17.939 18.09 18.241 18.392 18.543 18.693 18.844 18.995 19.146 19.296 19.447 19.598 19.749 19.899 20.05 20.201 20.352 20.502 20.653 20.804 20.955 21.105 21.256 21.407 21.558 21.708 21.859 22.01 22.161 22.311 22.462 22.613 22.764 22.914 23.065 23.216 23.367 23.517 23.668 23.819 23.97 24.12 24.271 24.422 24.573 24.723 24.874 25.025 25.176 25.326 25.477 25.628 25.779 25.929 26.08 26.231 26.382 26.532 26.683 26.834 26.985 27.135 27.286 27.437 27.588 27.738 27.889 28.04 28.191 28.341 28.492 28.643 28.794 28.944 29.095 29.246 29.397 29.547 29.698 29.849 30]
      | sbobj.Groups(1).Signals(2).YData = [0.16804 0.16819 0.16861 0.16923 0.17001 0.17093 0.17195 0.17305 0.1742 0.17541 0.17666 0.17793 0.17923 0.18054 0.18188 0.18322 0.18458 0.18595 0.18732 0.1887 0.19008 0.19147 0.19286 0.19425 0.19564 0.19703 0.19842 0.19981 0.2012 0.20259 0.20397 0.20535 0.20673 0.2081 0.20948 0.21085 0.21222 0.21359 0.21496 0.21632 0.21769 0.21906 0.22044 0.22181 0.22319 0.22458 0.22597 0.22738 0.22879 0.23021 0.23164 0.23309 0.23455 0.23602 0.23751 0.23902 0.24054 0.24207 0.24363 0.2452 0.24679 0.24839 0.25002 0.25166 0.25331 0.25498 0.25667 0.25837 0.26008 0.2618 0.26354 0.26528 0.26703 0.26879 0.27056 0.27233 0.27411 0.27589 0.27767 0.27945 0.28123 0.283 0.28478 0.28655 0.28832 0.29008 0.29184 0.2936 0.29535 0.2971 0.29884 0.30058 0.30231 0.30404 0.30577 0.30749 0.30922 0.31095 0.31268 0.31441 0.31614 0.31789 0.31963 0.32139 0.32316 0.32494 0.32673 0.32854 0.33036 0.3322 0.33405 0.33592 0.33782 0.33973 0.34166 0.34361 0.34558 0.34758 0.34959 0.35162 0.35367 0.35574 0.35782 0.35992 0.36204 0.36416 0.3663 0.36845 0.3706 0.37276 0.37493 0.37709 0.37926 0.38142 0.38358 0.38573 0.38788 0.39002 0.39214 0.39426 0.39636 0.39845 0.40052 0.40259 0.40464 0.40667 0.4087 0.41071 0.41272 0.41471 0.41671 0.4187 0.42069 0.42268 0.42468 0.42668 0.4287 0.43074 0.43279 0.43487 0.43697 0.43911 0.44128 0.44348 0.44572 0.44801 0.45033 0.4527 0.45511 0.45757 0.46008 0.46262 0.46521 0.46784 0.47051 0.47321 0.47593 0.47868 0.48145 0.48422 0.48701 0.48978 0.49255 0.49529 0.49801 0.50068 0.5033 0.50586 0.50835 0.51074 0.51304 0.51521 0.51725 0.51912 0.52082 0.5223 0.52353 0.52447 0.52508 0.52529]
      | sbobj.Groups(1).Signals(3).Name = 'Position z'
      | sbobj.Groups(1).Signals(3).XData = [0 0.15075 0.3015 0.45226 0.60301 0.75376 0.90451 1.0553 1.206 1.3568 1.5075 1.6583 1.809 1.9598 2.1105 2.2613 2.412 2.5628 2.7135 2.8643 3.015 3.1658 3.3165 3.4673 3.618 3.7688 3.9196 4.0703 4.2211 4.3718 4.5226 4.6733 4.8241 4.9748 5.1256 5.2763 5.4271 5.5778 5.7286 5.8793 6.0301 6.1808 6.3316 6.4823 6.6331 6.7838 6.9346 7.0853 7.2361 7.3869 7.5376 7.6884 7.8391 7.9899 8.1406 8.2914 8.4421 8.5929 8.7436 8.8944 9.0451 9.1959 9.3466 9.4974 9.6481 9.7989 9.9496 10.1 10.251 10.402 10.553 10.703 10.854 11.005 11.156 11.306 11.457 11.608 11.759 11.909 12.06 12.211 12.362 12.512 12.663 12.814 12.965 13.115 13.266 13.417 13.568 13.718 13.869 14.02 14.171 14.321 14.472 14.623 14.774 14.924 15.075 15.226 15.377 15.527 15.678 15.829 15.98 16.13 16.281 16.432 16.583 16.733 16.884 17.035 17.186 17.336 17.487 17.638 17.789 17.939 18.09 18.241 18.392 18.543 18.693 18.844 18.995 19.146 19.296 19.447 19.598 19.749 19.899 20.05 20.201 20.352 20.502 20.653 20.804 20.955 21.105 21.256 21.407 21.558 21.708 21.859 22.01 22.161 22.311 22.462 22.613 22.764 22.914 23.065 23.216 23.367 23.517 23.668 23.819 23.97 24.12 24.271 24.422 24.573 24.723 24.874 25.025 25.176 25.326 25.477 25.628 25.779 25.929 26.08 26.231 26.382 26.532 26.683 26.834 26.985 27.135 27.286 27.437 27.588 27.738 27.889 28.04 28.191 28.341 28.492 28.643 28.794 28.944 29.095 29.246 29.397 29.547 29.698 29.849 30]
      | sbobj.Groups(1).Signals(3).YData = [1.735 1.7355 1.737 1.7396 1.7435 1.7485 1.7547 1.7619 1.7701 1.7791 1.7889 1.7992 1.81 1.8211 1.8325 1.844 1.8557 1.8673 1.8789 1.8904 1.9017 1.9129 1.924 1.9348 1.9455 1.9559 1.9662 1.9764 1.9863 1.9962 2.0059 2.0155 2.0251 2.0346 2.044 2.0535 2.0629 2.0723 2.0817 2.0912 2.1007 2.1102 2.1198 2.1294 2.1391 2.1488 2.1585 2.1682 2.178 2.1878 2.1976 2.2074 2.2171 2.2269 2.2366 2.2463 2.2559 2.2655 2.275 2.2845 2.2939 2.3032 2.3124 2.3215 2.3306 2.3395 2.3484 2.3572 2.3659 2.3746 2.3831 2.3916 2.4 2.4083 2.4166 2.4248 2.4329 2.441 2.4491 2.4571 2.4651 2.4731 2.481 2.4889 2.4968 2.5047 2.5126 2.5204 2.5283 2.5361 2.5439 2.5518 2.5596 2.5674 2.5751 2.5829 2.5906 2.5983 2.606 2.6137 2.6213 2.6289 2.6364 2.6439 2.6513 2.6587 2.666 2.6733 2.6804 2.6876 2.6946 2.7016 2.7085 2.7153 2.722 2.7287 2.7353 2.7418 2.7483 2.7546 2.7609 2.7672 2.7733 2.7794 2.7855 2.7915 2.7974 2.8033 2.8091 2.815 2.8207 2.8265 2.8322 2.8379 2.8435 2.8492 2.8548 2.8604 2.866 2.8715 2.8771 2.8826 2.8881 2.8936 2.899 2.9045 2.9099 2.9152 2.9206 2.9258 2.9311 2.9362 2.9414 2.9464 2.9514 2.9563 2.9611 2.9659 2.9705 2.9751 2.9796 2.984 2.9883 2.9925 2.9966 3.0006 3.0045 3.0084 3.0122 3.0159 3.0195 3.0231 3.0266 3.0301 3.0336 3.037 3.0404 3.0438 3.0472 3.0506 3.054 3.0573 3.0607 3.0641 3.0674 3.0707 3.0739 3.0771 3.0802 3.0832 3.086 3.0887 3.0911 3.0934 3.0953 3.097 3.0983 3.0992 3.0998 3.1]
      | sbobj.Groups(1).TimeRange = [0 30]
      | sbobj.Groups(2).Name = 'Position1'
      | sbobj.Groups(2).Signals(1).Name = 'Position x'
      | sbobj.Groups(2).Signals(1).XData = [0 0.15075 0.3015 0.45226 0.60301 0.75376 0.90451 1.0553 1.206 1.3568 1.5075 1.6583 1.809 1.9598 2.1105 2.2613 2.412 2.5628 2.7135 2.8643 3.015 3.1658 3.3165 3.4673 3.618 3.7688 3.9196 4.0703 4.2211 4.3718 4.5226 4.6733 4.8241 4.9748 5.1256 5.2763 5.4271 5.5778 5.7286 5.8793 6.0301 6.1808 6.3316 6.4823 6.6331 6.7838 6.9346 7.0853 7.2361 7.3869 7.5376 7.6884 7.8391 7.9899 8.1406 8.2914 8.4421 8.5929 8.7436 8.8944 9.0451 9.1959 9.3466 9.4974 9.6481 9.7989 9.9496 10.1 10.251 10.402 10.553 10.703 10.854 11.005 11.156 11.306 11.457 11.608 11.759 11.909 12.06 12.211 12.362 12.512 12.663 12.814 12.965 13.115 13.266 13.417 13.568 13.718 13.869 14.02 14.171 14.321 14.472 14.623 14.774 14.924 15.075 15.226 15.377 15.527 15.678 15.829 15.98 16.13 16.281 16.432 16.583 16.733 16.884 17.035 17.186 17.336 17.487 17.638 17.789 17.939 18.09 18.241 18.392 18.543 18.693 18.844 18.995 19.146 19.296 19.447 19.598 19.749 19.899 20.05 20.201 20.352 20.502 20.653 20.804 20.955 21.105 21.256 21.407 21.558 21.708 21.859 22.01 22.161 22.311 22.462 22.613 22.764 22.914 23.065 23.216 23.367 23.517 23.668 23.819 23.97 24.12 24.271 24.422 24.573 24.723 24.874 25.025 25.176 25.326 25.477 25.628 25.779 25.929 26.08 26.231 26.382 26.532 26.683 26.834 26.985 27.135 27.286 27.437 27.588 27.738 27.889 28.04 28.191 28.341 28.492 28.643 28.794 28.944 29.095 29.246 29.397 29.547 29.698 29.849 30]
      | sbobj.Groups(2).Signals(1).YData = [4.1497 4.1496 4.1494 4.149 4.1484 4.1474 4.1461 4.1445 4.1427 4.1405 4.1382 4.1356 4.1328 4.1298 4.1268 4.1236 4.1203 4.117 4.1136 4.1102 4.1067 4.1033 4.0999 4.0964 4.093 4.0896 4.0862 4.0828 4.0794 4.076 4.0726 4.0692 4.0657 4.0622 4.0586 4.055 4.0513 4.0476 4.0438 4.0399 4.0359 4.0318 4.0277 4.0235 4.0192 4.0148 4.0104 4.0058 4.0012 3.9966 3.9918 3.987 3.9822 3.9773 3.9723 3.9674 3.9623 3.9573 3.9522 3.9471 3.9419 3.9368 3.9316 3.9265 3.9213 3.9161 3.9109 3.9056 3.9004 3.8951 3.8899 3.8846 3.8793 3.8739 3.8686 3.8632 3.8578 3.8523 3.8468 3.8413 3.8357 3.83 3.8243 3.8186 3.8128 3.8069 3.801 3.795 3.7889 3.7828 3.7766 3.7704 3.7641 3.7578 3.7513 3.7449 3.7384 3.7318 3.7252 3.7186 3.7119 3.7052 3.6984 3.6917 3.6849 3.678 3.6712 3.6644 3.6575 3.6506 3.6438 3.6369 3.63 3.6231 3.6163 3.6094 3.6025 3.5956 3.5887 3.5818 3.5749 3.5679 3.561 3.554 3.547 3.54 3.533 3.5259 3.5188 3.5116 3.5044 3.4972 3.4899 3.4825 3.4751 3.4676 3.4601 3.4525 3.4449 3.4371 3.4294 3.4216 3.4137 3.4058 3.3978 3.3898 3.3818 3.3737 3.3656 3.3575 3.3494 3.3412 3.3331 3.325 3.3169 3.3088 3.3007 3.2927 3.2847 3.2767 3.2687 3.2608 3.253 3.2451 3.2373 3.2295 3.2217 3.2139 3.2061 3.1983 3.1905 3.1826 3.1747 3.1668 3.1587 3.1506 3.1424 3.1341 3.1258 3.1173 3.1087 3.1 3.0912 3.0824 3.0736 3.0647 3.0559 3.0471 3.0385 3.0301 3.022 3.0143 3.0071 3.0004 2.9944 2.9892 2.9849 2.9817 2.9797 2.979]
      | sbobj.Groups(2).Signals(2).Name = 'Position y'
      | sbobj.Groups(2).Signals(2).XData = [0 0.15075 0.3015 0.45226 0.60301 0.75376 0.90451 1.0553 1.206 1.3568 1.5075 1.6583 1.809 1.9598 2.1105 2.2613 2.412 2.5628 2.7135 2.8643 3.015 3.1658 3.3165 3.4673 3.618 3.7688 3.9196 4.0703 4.2211 4.3718 4.5226 4.6733 4.8241 4.9748 5.1256 5.2763 5.4271 5.5778 5.7286 5.8793 6.0301 6.1808 6.3316 6.4823 6.6331 6.7838 6.9346 7.0853 7.2361 7.3869 7.5376 7.6884 7.8391 7.9899 8.1406 8.2914 8.4421 8.5929 8.7436 8.8944 9.0451 9.1959 9.3466 9.4974 9.6481 9.7989 9.9496 10.1 10.251 10.402 10.553 10.703 10.854 11.005 11.156 11.306 11.457 11.608 11.759 11.909 12.06 12.211 12.362 12.512 12.663 12.814 12.965 13.115 13.266 13.417 13.568 13.718 13.869 14.02 14.171 14.321 14.472 14.623 14.774 14.924 15.075 15.226 15.377 15.527 15.678 15.829 15.98 16.13 16.281 16.432 16.583 16.733 16.884 17.035 17.186 17.336 17.487 17.638 17.789 17.939 18.09 18.241 18.392 18.543 18.693 18.844 18.995 19.146 19.296 19.447 19.598 19.749 19.899 20.05 20.201 20.352 20.502 20.653 20.804 20.955 21.105 21.256 21.407 21.558 21.708 21.859 22.01 22.161 22.311 22.462 22.613 22.764 22.914 23.065 23.216 23.367 23.517 23.668 23.819 23.97 24.12 24.271 24.422 24.573 24.723 24.874 25.025 25.176 25.326 25.477 25.628 25.779 25.929 26.08 26.231 26.382 26.532 26.683 26.834 26.985 27.135 27.286 27.437 27.588 27.738 27.889 28.04 28.191 28.341 28.492 28.643 28.794 28.944 29.095 29.246 29.397 29.547 29.698 29.849 30]
      | sbobj.Groups(2).Signals(2).YData = [0.16804 0.16819 0.16861 0.16923 0.17001 0.17093 0.17195 0.17305 0.1742 0.17541 0.17666 0.17793 0.17923 0.18054 0.18188 0.18322 0.18458 0.18595 0.18732 0.1887 0.19008 0.19147 0.19286 0.19425 0.19564 0.19703 0.19842 0.19981 0.2012 0.20259 0.20397 0.20535 0.20673 0.2081 0.20948 0.21085 0.21222 0.21359 0.21496 0.21632 0.21769 0.21906 0.22044 0.22181 0.22319 0.22458 0.22597 0.22738 0.22879 0.23021 0.23164 0.23309 0.23455 0.23602 0.23751 0.23902 0.24054 0.24207 0.24363 0.2452 0.24679 0.24839 0.25002 0.25166 0.25331 0.25498 0.25667 0.25837 0.26008 0.2618 0.26354 0.26528 0.26703 0.26879 0.27056 0.27233 0.27411 0.27589 0.27767 0.27945 0.28123 0.283 0.28478 0.28655 0.28832 0.29008 0.29184 0.2936 0.29535 0.2971 0.29884 0.30058 0.30231 0.30404 0.30577 0.30749 0.30922 0.31095 0.31268 0.31441 0.31614 0.31789 0.31963 0.32139 0.32316 0.32494 0.32673 0.32854 0.33036 0.3322 0.33405 0.33592 0.33782 0.33973 0.34166 0.34361 0.34558 0.34758 0.34959 0.35162 0.35367 0.35574 0.35782 0.35992 0.36204 0.36416 0.3663 0.36845 0.3706 0.37276 0.37493 0.37709 0.37926 0.38142 0.38358 0.38573 0.38788 0.39002 0.39214 0.39426 0.39636 0.39845 0.40052 0.40259 0.40464 0.40667 0.4087 0.41071 0.41272 0.41471 0.41671 0.4187 0.42069 0.42268 0.42468 0.42668 0.4287 0.43074 0.43279 0.43487 0.43697 0.43911 0.44128 0.44348 0.44572 0.44801 0.45033 0.4527 0.45511 0.45757 0.46008 0.46262 0.46521 0.46784 0.47051 0.47321 0.47593 0.47868 0.48145 0.48422 0.48701 0.48978 0.49255 0.49529 0.49801 0.50068 0.5033 0.50586 0.50835 0.51074 0.51304 0.51521 0.51725 0.51912 0.52082 0.5223 0.52353 0.52447 0.52508 0.52529]
      | sbobj.Groups(2).Signals(3).Name = 'Position z'
      | sbobj.Groups(2).Signals(3).XData = [0 0.15075 0.3015 0.45226 0.60301 0.75376 0.90451 1.0553 1.206 1.3568 1.5075 1.6583 1.809 1.9598 2.1105 2.2613 2.412 2.5628 2.7135 2.8643 3.015 3.1658 3.3165 3.4673 3.618 3.7688 3.9196 4.0703 4.2211 4.3718 4.5226 4.6733 4.8241 4.9748 5.1256 5.2763 5.4271 5.5778 5.7286 5.8793 6.0301 6.1808 6.3316 6.4823 6.6331 6.7838 6.9346 7.0853 7.2361 7.3869 7.5376 7.6884 7.8391 7.9899 8.1406 8.2914 8.4421 8.5929 8.7436 8.8944 9.0451 9.1959 9.3466 9.4974 9.6481 9.7989 9.9496 10.1 10.251 10.402 10.553 10.703 10.854 11.005 11.156 11.306 11.457 11.608 11.759 11.909 12.06 12.211 12.362 12.512 12.663 12.814 12.965 13.115 13.266 13.417 13.568 13.718 13.869 14.02 14.171 14.321 14.472 14.623 14.774 14.924 15.075 15.226 15.377 15.527 15.678 15.829 15.98 16.13 16.281 16.432 16.583 16.733 16.884 17.035 17.186 17.336 17.487 17.638 17.789 17.939 18.09 18.241 18.392 18.543 18.693 18.844 18.995 19.146 19.296 19.447 19.598 19.749 19.899 20.05 20.201 20.352 20.502 20.653 20.804 20.955 21.105 21.256 21.407 21.558 21.708 21.859 22.01 22.161 22.311 22.462 22.613 22.764 22.914 23.065 23.216 23.367 23.517 23.668 23.819 23.97 24.12 24.271 24.422 24.573 24.723 24.874 25.025 25.176 25.326 25.477 25.628 25.779 25.929 26.08 26.231 26.382 26.532 26.683 26.834 26.985 27.135 27.286 27.437 27.588 27.738 27.889 28.04 28.191 28.341 28.492 28.643 28.794 28.944 29.095 29.246 29.397 29.547 29.698 29.849 30]
      | sbobj.Groups(2).Signals(3).YData = [1.735 1.7355 1.737 1.7396 1.7435 1.7485 1.7547 1.7619 1.7701 1.7791 1.7889 1.7992 1.81 1.8211 1.8325 1.844 1.8557 1.8673 1.8789 1.8904 1.9017 1.9129 1.924 1.9348 1.9455 1.9559 1.9662 1.9764 1.9863 1.9962 2.0059 2.0155 2.0251 2.0346 2.044 2.0535 2.0629 2.0723 2.0817 2.0912 2.1007 2.1102 2.1198 2.1294 2.1391 2.1488 2.1585 2.1682 2.178 2.1878 2.1976 2.2074 2.2171 2.2269 2.2366 2.2463 2.2559 2.2655 2.275 2.2845 2.2939 2.3032 2.3124 2.3215 2.3306 2.3395 2.3484 2.3572 2.3659 2.3746 2.3831 2.3916 2.4 2.4083 2.4166 2.4248 2.4329 2.441 2.4491 2.4571 2.4651 2.4731 2.481 2.4889 2.4968 2.5047 2.5126 2.5204 2.5283 2.5361 2.5439 2.5518 2.5596 2.5674 2.5751 2.5829 2.5906 2.5983 2.606 2.6137 2.6213 2.6289 2.6364 2.6439 2.6513 2.6587 2.666 2.6733 2.6804 2.6876 2.6946 2.7016 2.7085 2.7153 2.722 2.7287 2.7353 2.7418 2.7483 2.7546 2.7609 2.7672 2.7733 2.7794 2.7855 2.7915 2.7974 2.8033 2.8091 2.815 2.8207 2.8265 2.8322 2.8379 2.8435 2.8492 2.8548 2.8604 2.866 2.8715 2.8771 2.8826 2.8881 2.8936 2.899 2.9045 2.9099 2.9152 2.9206 2.9258 2.9311 2.9362 2.9414 2.9464 2.9514 2.9563 2.9611 2.9659 2.9705 2.9751 2.9796 2.984 2.9883 2.9925 2.9966 3.0006 3.0045 3.0084 3.0122 3.0159 3.0195 3.0231 3.0266 3.0301 3.0336 3.037 3.0404 3.0438 3.0472 3.0506 3.054 3.0573 3.0607 3.0641 3.0674 3.0707 3.0739 3.0771 3.0802 3.0832 3.086 3.0887 3.0911 3.0934 3.0953 3.097 3.0983 3.0992 3.0998 3.1]
      | sbobj.Groups(2).TimeRange = [0 30]
  Subsystem : Subsystem
  Bus : Outport
  wires:
  FromWs/1 -> Subsystem/1(In1)
  Bus Creator/1 -> Bus/1
  Subsystem/1(Position x) -> Bus Creator/1  "Position x"
  Subsystem/2(Position y) -> Bus Creator/2  "Position y"
  Subsystem/3(Position z) -> Bus Creator/3  "Position z"

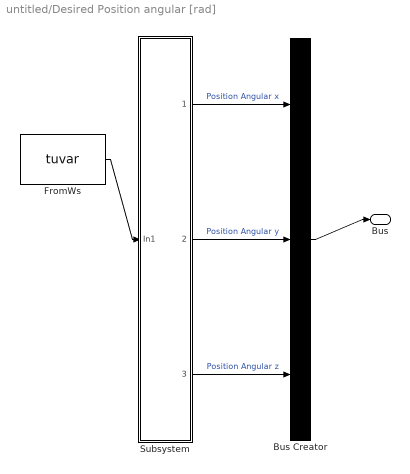
== system untitled/Desired Position angular [rad] ==
  Bus Creator : BusCreator  Tag=Bus Creator  Inputs=3
  FromWs : FromWorkspace  Tag=STV FromWs  VariableName=tuvar  SampleTime=0
      SigBuilderData=|
      | common.afterFinalStr = 'Extrapolate'
      | common.sampleTime = 0
      | dataSet(1).timeRange = [0 30]
      | dataSet(1).name = 'Position'
      | dataSet(2).timeRange = [0 30]
      | dataSet(2).name = 'Position1'
      | sbobj.Groups(1).Name = 'Position'
      | sbobj.Groups(1).Signals(1).Name = 'Position Angular x'
      | sbobj.Groups(1).Signals(1).XData = [0 0.15075 0.3015 0.45226 0.60301 0.75376 0.90451 1.0553 1.206 1.3568 1.5075 1.6583 1.809 1.9598 2.1105 2.2613 2.412 2.5628 2.7135 2.8643 3.015 3.1658 3.3165 3.4673 3.618 3.7688 3.9196 4.0703 4.2211 4.3718 4.5226 4.6733 4.8241 4.9748 5.1256 5.2763 5.4271 5.5778 5.7286 5.8793 6.0301 6.1808 6.3316 6.4823 6.6331 6.7838 6.9346 7.0853 7.2361 7.3869 7.5376 7.6884 7.8391 7.9899 8.1406 8.2914 8.4421 8.5929 8.7436 8.8944 9.0451 9.1959 9.3466 9.4974 9.6481 9.7989 9.9496 10.1 10.251 10.402 10.553 10.703 10.854 11.005 11.156 11.306 11.457 11.608 11.759 11.909 12.06 12.211 12.362 12.512 12.663 12.814 12.965 13.115 13.266 13.417 13.568 13.718 13.869 14.02 14.171 14.321 14.472 14.623 14.774 14.924 15.075 15.226 15.377 15.527 15.678 15.829 15.98 16.13 16.281 16.432 16.583 16.733 16.884 17.035 17.186 17.336 17.487 17.638 17.789 17.939 18.09 18.241 18.392 18.543 18.693 18.844 18.995 19.146 19.296 19.447 19.598 19.749 19.899 20.05 20.201 20.352 20.502 20.653 20.804 20.955 21.105 21.256 21.407 21.558 21.708 21.859 22.01 22.161 22.311 22.462 22.613 22.764 22.914 23.065 23.216 23.367 23.517 23.668 23.819 23.97 24.12 24.271 24.422 24.573 24.723 24.874 25.025 25.176 25.326 25.477 25.628 25.779 25.929 26.08 26.231 26.382 26.532 26.683 26.834 26.985 27.135 27.286 27.437 27.588 27.738 27.889 28.04 28.191 28.341 28.492 28.643 28.794 28.944 29.095 29.246 29.397 29.547 29.698 29.849 30]
      | sbobj.Groups(1).Signals(1).YData = [-1.2662 -2.371 -2.4879 -2.5537 -2.6023 -2.6406 -2.6717 -2.6974 -2.7189 -2.7372 -2.7527 -2.7661 -2.7777 -2.7877 -2.7963 -2.8039 -2.8104 -2.8161 -2.821 -2.8252 -2.8289 -2.832 -2.8346 -2.8369 -2.8388 -2.8404 -2.8417 -2.8429 -2.8438 -2.8446 -2.8453 -2.8459 -2.8464 -2.8469 -2.8474 -2.8479 -2.8484 -2.8489 -2.8495 -2.85 -2.8507 -2.8513 -2.852 -2.8528 -2.8536 -2.8544 -2.8552 -2.856 -2.8569 -2.8577 -2.8586 -2.8594 -2.8602 -2.861 -2.8617 -2.8624 -2.863 -2.8636 -2.8641 -2.8646 -2.865 -2.8654 -2.8656 -2.8659 -2.866 -2.8662 -2.8662 -2.8662 -2.8662 -2.8661 -2.866 -2.8659 -2.8657 -2.8655 -2.8653 -2.8651 -2.8649 -2.8647 -2.8645 -2.8643 -2.8641 -2.8639 -2.8638 -2.8637 -2.8636 -2.8635 -2.8635 -2.8635 -2.8635 -2.8636 -2.8637 -2.8638 -2.864 -2.8641 -2.8643 -2.8646 -2.8648 -2.865 -2.8653 -2.8655 -2.8658 -2.866 -2.8662 -2.8664 -2.8666 -2.8668 -2.8669 -2.867 -2.8671 -2.8672 -2.8672 -2.8672 -2.8671 -2.867 -2.8668 -2.8666 -2.8664 -2.8662 -2.8659 -2.8655 -2.8652 -2.8648 -2.8644 -2.864 -2.8635 -2.863 -2.8626 -2.8621 -2.8616 -2.8612 -2.8607 -2.8602 -2.8598 -2.8594 -2.859 -2.8586 -2.8582 -2.8579 -2.8576 -2.8573 -2.8571 -2.8568 -2.8566 -2.8565 -2.8563 -2.8562 -2.8561 -2.856 -2.8559 -2.8558 -2.8557 -2.8556 -2.8555 -2.8554 -2.8553 -2.8551 -2.8549 -2.8547 -2.8544 -2.8541 -2.8538 -2.8534 -2.853 -2.8525 -2.852 -2.8514 -2.8508 -2.8502 -2.8495 -2.8487 -2.8479 -2.8471 -2.8463 -2.8454 -2.8445 -2.8436 -2.8428 -2.8419 -2.841 -2.8401 -2.8393 -2.8384 -2.8376 -2.8368 -2.8361 -2.8354 -2.8347 -2.834 -2.8334 -2.8328 -2.8322 -2.8317 -2.8312 -2.8307 -2.8303 -2.8299 -2.8295 -2.8292 -2.8291 -2.8291]
      | sbobj.Groups(1).Signals(2).Name = 'Position Angular y'
      | sbobj.Groups(1).Signals(2).XData = [0 0.15075 0.3015 0.45226 0.60301 0.75376 0.90451 1.0553 1.206 1.3568 1.5075 1.6583 1.809 1.9598 2.1105 2.2613 2.412 2.5628 2.7135 2.8643 3.015 3.1658 3.3165 3.4673 3.618 3.7688 3.9196 4.0703 4.2211 4.3718 4.5226 4.6733 4.8241 4.9748 5.1256 5.2763 5.4271 5.5778 5.7286 5.8793 6.0301 6.1808 6.3316 6.4823 6.6331 6.7838 6.9346 7.0853 7.2361 7.3869 7.5376 7.6884 7.8391 7.9899 8.1406 8.2914 8.4421 8.5929 8.7436 8.8944 9.0451 9.1959 9.3466 9.4974 9.6481 9.7989 9.9496 10.1 10.251 10.402 10.553 10.703 10.854 11.005 11.156 11.306 11.457 11.608 11.759 11.909 12.06 12.211 12.362 12.512 12.663 12.814 12.965 13.115 13.266 13.417 13.568 13.718 13.869 14.02 14.171 14.321 14.472 14.623 14.774 14.924 15.075 15.226 15.377 15.527 15.678 15.829 15.98 16.13 16.281 16.432 16.583 16.733 16.884 17.035 17.186 17.336 17.487 17.638 17.789 17.939 18.09 18.241 18.392 18.543 18.693 18.844 18.995 19.146 19.296 19.447 19.598 19.749 19.899 20.05 20.201 20.352 20.502 20.653 20.804 20.955 21.105 21.256 21.407 21.558 21.708 21.859 22.01 22.161 22.311 22.462 22.613 22.764 22.914 23.065 23.216 23.367 23.517 23.668 23.819 23.97 24.12 24.271 24.422 24.573 24.723 24.874 25.025 25.176 25.326 25.477 25.628 25.779 25.929 26.08 26.231 26.382 26.532 26.683 26.834 26.985 27.135 27.286 27.437 27.588 27.738 27.889 28.04 28.191 28.341 28.492 28.643 28.794 28.944 29.095 29.246 29.397 29.547 29.698 29.849 30]
      | sbobj.Groups(1).Signals(2).YData = [-1.5708 -1.5706 -1.5699 -1.5687 -1.5669 -1.5646 -1.5618 -1.5584 -1.5546 -1.5504 -1.5458 -1.5409 -1.5358 -1.5305 -1.525 -1.5195 -1.5138 -1.5082 -1.5025 -1.4969 -1.4914 -1.4859 -1.4804 -1.4751 -1.4698 -1.4647 -1.4596 -1.4546 -1.4496 -1.4447 -1.4399 -1.4351 -1.4303 -1.4255 -1.4208 -1.416 -1.4113 -1.4065 -1.4017 -1.3969 -1.392 -1.3871 -1.3822 -1.3772 -1.3722 -1.3672 -1.3621 -1.3569 -1.3518 -1.3466 -1.3414 -1.3361 -1.3309 -1.3256 -1.3204 -1.3151 -1.3098 -1.3046 -1.2993 -1.2941 -1.2889 -1.2837 -1.2785 -1.2734 -1.2683 -1.2632 -1.2582 -1.2532 -1.2482 -1.2432 -1.2383 -1.2334 -1.2285 -1.2236 -1.2187 -1.2139 -1.2091 -1.2042 -1.1994 -1.1946 -1.1898 -1.185 -1.1801 -1.1753 -1.1704 -1.1655 -1.1606 -1.1557 -1.1508 -1.1459 -1.1409 -1.1359 -1.1309 -1.1259 -1.1209 -1.1158 -1.1108 -1.1057 -1.1006 -1.0955 -1.0904 -1.0853 -1.0802 -1.0751 -1.07 -1.065 -1.0599 -1.0549 -1.0498 -1.0448 -1.0398 -1.0348 -1.0299 -1.0249 -1.02 -1.0151 -1.0103 -1.0054 -1.0006 -0.9958 -0.99101 -0.98623 -0.98146 -0.97671 -0.97195 -0.96721 -0.96246 -0.95771 -0.95296 -0.9482 -0.94342 -0.93864 -0.93384 -0.92902 -0.92418 -0.91932 -0.91444 -0.90954 -0.90462 -0.89967 -0.8947 -0.88972 -0.88471 -0.87969 -0.87466 -0.86962 -0.86457 -0.85952 -0.85448 -0.84944 -0.8444 -0.83939 -0.83439 -0.82941 -0.82446 -0.81954 -0.81465 -0.8098 -0.80498 -0.8002 -0.79546 -0.79075 -0.78608 -0.78143 -0.77682 -0.77223 -0.76765 -0.76309 -0.75853 -0.75396 -0.74939 -0.74479 -0.74016 -0.7355 -0.73079 -0.72604 -0.72122 -0.71635 -0.71142 -0.70643 -0.70139 -0.6963 -0.69118 -0.68603 -0.68089 -0.67576 -0.6707 -0.66571 -0.66086 -0.65617 -0.65169 -0.64747 -0.64355 -0.64 -0.63685 -0.63414 -0.63191 -0.63017 -0.62894 -0.62818]
      | sbobj.Groups(1).Signals(3).Name = 'Position Angular z'
      | sbobj.Groups(1).Signals(3).XData = [0 0.15075 0.3015 0.45226 0.60301 0.75376 0.90451 1.0553 1.206 1.3568 1.5075 1.6583 1.809 1.9598 2.1105 2.2613 2.412 2.5628 2.7135 2.8643 3.015 3.1658 3.3165 3.4673 3.618 3.7688 3.9196 4.0703 4.2211 4.3718 4.5226 4.6733 4.8241 4.9748 5.1256 5.2763 5.4271 5.5778 5.7286 5.8793 6.0301 6.1808 6.3316 6.4823 6.6331 6.7838 6.9346 7.0853 7.2361 7.3869 7.5376 7.6884 7.8391 7.9899 8.1406 8.2914 8.4421 8.5929 8.7436 8.8944 9.0451 9.1959 9.3466 9.4974 9.6481 9.7989 9.9496 10.1 10.251 10.402 10.553 10.703 10.854 11.005 11.156 11.306 11.457 11.608 11.759 11.909 12.06 12.211 12.362 12.512 12.663 12.814 12.965 13.115 13.266 13.417 13.568 13.718 13.869 14.02 14.171 14.321 14.472 14.623 14.774 14.924 15.075 15.226 15.377 15.527 15.678 15.829 15.98 16.13 16.281 16.432 16.583 16.733 16.884 17.035 17.186 17.336 17.487 17.638 17.789 17.939 18.09 18.241 18.392 18.543 18.693 18.844 18.995 19.146 19.296 19.447 19.598 19.749 19.899 20.05 20.201 20.352 20.502 20.653 20.804 20.955 21.105 21.256 21.407 21.558 21.708 21.859 22.01 22.161 22.311 22.462 22.613 22.764 22.914 23.065 23.216 23.367 23.517 23.668 23.819 23.97 24.12 24.271 24.422 24.573 24.723 24.874 25.025 25.176 25.326 25.477 25.628 25.779 25.929 26.08 26.231 26.382 26.532 26.683 26.834 26.985 27.135 27.286 27.437 27.588 27.738 27.889 28.04 28.191 28.341 28.492 28.643 28.794 28.944 29.095 29.246 29.397 29.547 29.698 29.849 30]
      | sbobj.Groups(1).Signals(3).YData = [1.2662 2.3711 2.4881 2.554 2.6028 2.6413 2.6726 2.6985 2.7203 2.7387 2.7545 2.7681 2.7799 2.7901 2.799 2.8067 2.8135 2.8194 2.8246 2.8291 2.833 2.8364 2.8393 2.8419 2.8441 2.846 2.8476 2.849 2.8502 2.8513 2.8523 2.8532 2.854 2.8547 2.8554 2.8562 2.8569 2.8577 2.8584 2.8593 2.8601 2.861 2.8619 2.8629 2.8639 2.8649 2.866 2.8671 2.8681 2.8692 2.8703 2.8714 2.8725 2.8735 2.8745 2.8755 2.8764 2.8773 2.8781 2.8789 2.8796 2.8803 2.8809 2.8815 2.882 2.8825 2.8829 2.8832 2.8835 2.8838 2.8841 2.8843 2.8844 2.8846 2.8847 2.8849 2.885 2.8851 2.8852 2.8854 2.8855 2.8857 2.8859 2.8861 2.8863 2.8866 2.8869 2.8872 2.8876 2.888 2.8884 2.8889 2.8894 2.8899 2.8905 2.891 2.8916 2.8922 2.8928 2.8934 2.8941 2.8947 2.8953 2.8959 2.8965 2.8971 2.8977 2.8982 2.8987 2.8992 2.8997 2.9001 2.9005 2.9008 2.9011 2.9014 2.9016 2.9018 2.902 2.9021 2.9022 2.9023 2.9024 2.9024 2.9024 2.9024 2.9024 2.9024 2.9024 2.9024 2.9024 2.9024 2.9025 2.9025 2.9026 2.9027 2.9029 2.903 2.9032 2.9035 2.9038 2.9041 2.9044 2.9048 2.9052 2.9056 2.906 2.9065 2.907 2.9075 2.908 2.9085 2.9089 2.9094 2.9099 2.9103 2.9107 2.9111 2.9114 2.9117 2.912 2.9122 2.9123 2.9125 2.9125 2.9126 2.9125 2.9125 2.9124 2.9123 2.9121 2.912 2.9118 2.9117 2.9115 2.9114 2.9112 2.9111 2.9111 2.9111 2.9111 2.9112 2.9113 2.9114 2.9116 2.9118 2.912 2.9122 2.9124 2.9126 2.9128 2.9128 2.9129 2.9128 2.9128 2.9127 2.9126 2.9125 2.9127 2.9131]
      | sbobj.Groups(1).TimeRange = [0 30]
      | sbobj.Groups(2).Name = 'Position1'
      | sbobj.Groups(2).Signals(1).Name = 'Position Angular x'
      | sbobj.Groups(2).Signals(1).XData = [0 0.15075 0.3015 0.45226 0.60301 0.75376 0.90451 1.0553 1.206 1.3568 1.5075 1.6583 1.809 1.9598 2.1105 2.2613 2.412 2.5628 2.7135 2.8643 3.015 3.1658 3.3165 3.4673 3.618 3.7688 3.9196 4.0703 4.2211 4.3718 4.5226 4.6733 4.8241 4.9748 5.1256 5.2763 5.4271 5.5778 5.7286 5.8793 6.0301 6.1808 6.3316 6.4823 6.6331 6.7838 6.9346 7.0853 7.2361 7.3869 7.5376 7.6884 7.8391 7.9899 8.1406 8.2914 8.4421 8.5929 8.7436 8.8944 9.0451 9.1959 9.3466 9.4974 9.6481 9.7989 9.9496 10.1 10.251 10.402 10.553 10.703 10.854 11.005 11.156 11.306 11.457 11.608 11.759 11.909 12.06 12.211 12.362 12.512 12.663 12.814 12.965 13.115 13.266 13.417 13.568 13.718 13.869 14.02 14.171 14.321 14.472 14.623 14.774 14.924 15.075 15.226 15.377 15.527 15.678 15.829 15.98 16.13 16.281 16.432 16.583 16.733 16.884 17.035 17.186 17.336 17.487 17.638 17.789 17.939 18.09 18.241 18.392 18.543 18.693 18.844 18.995 19.146 19.296 19.447 19.598 19.749 19.899 20.05 20.201 20.352 20.502 20.653 20.804 20.955 21.105 21.256 21.407 21.558 21.708 21.859 22.01 22.161 22.311 22.462 22.613 22.764 22.914 23.065 23.216 23.367 23.517 23.668 23.819 23.97 24.12 24.271 24.422 24.573 24.723 24.874 25.025 25.176 25.326 25.477 25.628 25.779 25.929 26.08 26.231 26.382 26.532 26.683 26.834 26.985 27.135 27.286 27.437 27.588 27.738 27.889 28.04 28.191 28.341 28.492 28.643 28.794 28.944 29.095 29.246 29.397 29.547 29.698 29.849 30]
      | sbobj.Groups(2).Signals(1).YData = [-1.2662 -2.371 -2.4879 -2.5537 -2.6023 -2.6406 -2.6717 -2.6974 -2.7189 -2.7372 -2.7527 -2.7661 -2.7777 -2.7877 -2.7963 -2.8039 -2.8104 -2.8161 -2.821 -2.8252 -2.8289 -2.832 -2.8346 -2.8369 -2.8388 -2.8404 -2.8417 -2.8429 -2.8438 -2.8446 -2.8453 -2.8459 -2.8464 -2.8469 -2.8474 -2.8479 -2.8484 -2.8489 -2.8495 -2.85 -2.8507 -2.8513 -2.852 -2.8528 -2.8536 -2.8544 -2.8552 -2.856 -2.8569 -2.8577 -2.8586 -2.8594 -2.8602 -2.861 -2.8617 -2.8624 -2.863 -2.8636 -2.8641 -2.8646 -2.865 -2.8654 -2.8656 -2.8659 -2.866 -2.8662 -2.8662 -2.8662 -2.8662 -2.8661 -2.866 -2.8659 -2.8657 -2.8655 -2.8653 -2.8651 -2.8649 -2.8647 -2.8645 -2.8643 -2.8641 -2.8639 -2.8638 -2.8637 -2.8636 -2.8635 -2.8635 -2.8635 -2.8635 -2.8636 -2.8637 -2.8638 -2.864 -2.8641 -2.8643 -2.8646 -2.8648 -2.865 -2.8653 -2.8655 -2.8658 -2.866 -2.8662 -2.8664 -2.8666 -2.8668 -2.8669 -2.867 -2.8671 -2.8672 -2.8672 -2.8672 -2.8671 -2.867 -2.8668 -2.8666 -2.8664 -2.8662 -2.8659 -2.8655 -2.8652 -2.8648 -2.8644 -2.864 -2.8635 -2.863 -2.8626 -2.8621 -2.8616 -2.8612 -2.8607 -2.8602 -2.8598 -2.8594 -2.859 -2.8586 -2.8582 -2.8579 -2.8576 -2.8573 -2.8571 -2.8568 -2.8566 -2.8565 -2.8563 -2.8562 -2.8561 -2.856 -2.8559 -2.8558 -2.8557 -2.8556 -2.8555 -2.8554 -2.8553 -2.8551 -2.8549 -2.8547 -2.8544 -2.8541 -2.8538 -2.8534 -2.853 -2.8525 -2.852 -2.8514 -2.8508 -2.8502 -2.8495 -2.8487 -2.8479 -2.8471 -2.8463 -2.8454 -2.8445 -2.8436 -2.8428 -2.8419 -2.841 -2.8401 -2.8393 -2.8384 -2.8376 -2.8368 -2.8361 -2.8354 -2.8347 -2.834 -2.8334 -2.8328 -2.8322 -2.8317 -2.8312 -2.8307 -2.8303 -2.8299 -2.8295 -2.8292 -2.8291 -2.8291]
      | sbobj.Groups(2).Signals(2).Name = 'Position Angular y'
      | sbobj.Groups(2).Signals(2).XData = [0 0.15075 0.3015 0.45226 0.60301 0.75376 0.90451 1.0553 1.206 1.3568 1.5075 1.6583 1.809 1.9598 2.1105 2.2613 2.412 2.5628 2.7135 2.8643 3.015 3.1658 3.3165 3.4673 3.618 3.7688 3.9196 4.0703 4.2211 4.3718 4.5226 4.6733 4.8241 4.9748 5.1256 5.2763 5.4271 5.5778 5.7286 5.8793 6.0301 6.1808 6.3316 6.4823 6.6331 6.7838 6.9346 7.0853 7.2361 7.3869 7.5376 7.6884 7.8391 7.9899 8.1406 8.2914 8.4421 8.5929 8.7436 8.8944 9.0451 9.1959 9.3466 9.4974 9.6481 9.7989 9.9496 10.1 10.251 10.402 10.553 10.703 10.854 11.005 11.156 11.306 11.457 11.608 11.759 11.909 12.06 12.211 12.362 12.512 12.663 12.814 12.965 13.115 13.266 13.417 13.568 13.718 13.869 14.02 14.171 14.321 14.472 14.623 14.774 14.924 15.075 15.226 15.377 15.527 15.678 15.829 15.98 16.13 16.281 16.432 16.583 16.733 16.884 17.035 17.186 17.336 17.487 17.638 17.789 17.939 18.09 18.241 18.392 18.543 18.693 18.844 18.995 19.146 19.296 19.447 19.598 19.749 19.899 20.05 20.201 20.352 20.502 20.653 20.804 20.955 21.105 21.256 21.407 21.558 21.708 21.859 22.01 22.161 22.311 22.462 22.613 22.764 22.914 23.065 23.216 23.367 23.517 23.668 23.819 23.97 24.12 24.271 24.422 24.573 24.723 24.874 25.025 25.176 25.326 25.477 25.628 25.779 25.929 26.08 26.231 26.382 26.532 26.683 26.834 26.985 27.135 27.286 27.437 27.588 27.738 27.889 28.04 28.191 28.341 28.492 28.643 28.794 28.944 29.095 29.246 29.397 29.547 29.698 29.849 30]
      | sbobj.Groups(2).Signals(2).YData = [-1.5708 -1.5706 -1.5699 -1.5687 -1.5669 -1.5646 -1.5618 -1.5584 -1.5546 -1.5504 -1.5458 -1.5409 -1.5358 -1.5305 -1.525 -1.5195 -1.5138 -1.5082 -1.5025 -1.4969 -1.4914 -1.4859 -1.4804 -1.4751 -1.4698 -1.4647 -1.4596 -1.4546 -1.4496 -1.4447 -1.4399 -1.4351 -1.4303 -1.4255 -1.4208 -1.416 -1.4113 -1.4065 -1.4017 -1.3969 -1.392 -1.3871 -1.3822 -1.3772 -1.3722 -1.3672 -1.3621 -1.3569 -1.3518 -1.3466 -1.3414 -1.3361 -1.3309 -1.3256 -1.3204 -1.3151 -1.3098 -1.3046 -1.2993 -1.2941 -1.2889 -1.2837 -1.2785 -1.2734 -1.2683 -1.2632 -1.2582 -1.2532 -1.2482 -1.2432 -1.2383 -1.2334 -1.2285 -1.2236 -1.2187 -1.2139 -1.2091 -1.2042 -1.1994 -1.1946 -1.1898 -1.185 -1.1801 -1.1753 -1.1704 -1.1655 -1.1606 -1.1557 -1.1508 -1.1459 -1.1409 -1.1359 -1.1309 -1.1259 -1.1209 -1.1158 -1.1108 -1.1057 -1.1006 -1.0955 -1.0904 -1.0853 -1.0802 -1.0751 -1.07 -1.065 -1.0599 -1.0549 -1.0498 -1.0448 -1.0398 -1.0348 -1.0299 -1.0249 -1.02 -1.0151 -1.0103 -1.0054 -1.0006 -0.9958 -0.99101 -0.98623 -0.98146 -0.97671 -0.97195 -0.96721 -0.96246 -0.95771 -0.95296 -0.9482 -0.94342 -0.93864 -0.93384 -0.92902 -0.92418 -0.91932 -0.91444 -0.90954 -0.90462 -0.89967 -0.8947 -0.88972 -0.88471 -0.87969 -0.87466 -0.86962 -0.86457 -0.85952 -0.85448 -0.84944 -0.8444 -0.83939 -0.83439 -0.82941 -0.82446 -0.81954 -0.81465 -0.8098 -0.80498 -0.8002 -0.79546 -0.79075 -0.78608 -0.78143 -0.77682 -0.77223 -0.76765 -0.76309 -0.75853 -0.75396 -0.74939 -0.74479 -0.74016 -0.7355 -0.73079 -0.72604 -0.72122 -0.71635 -0.71142 -0.70643 -0.70139 -0.6963 -0.69118 -0.68603 -0.68089 -0.67576 -0.6707 -0.66571 -0.66086 -0.65617 -0.65169 -0.64747 -0.64355 -0.64 -0.63685 -0.63414 -0.63191 -0.63017 -0.62894 -0.62818]
      | sbobj.Groups(2).Signals(3).Name = 'Position Angular z'
      | sbobj.Groups(2).Signals(3).XData = [0 0.15075 0.3015 0.45226 0.60301 0.75376 0.90451 1.0553 1.206 1.3568 1.5075 1.6583 1.809 1.9598 2.1105 2.2613 2.412 2.5628 2.7135 2.8643 3.015 3.1658 3.3165 3.4673 3.618 3.7688 3.9196 4.0703 4.2211 4.3718 4.5226 4.6733 4.8241 4.9748 5.1256 5.2763 5.4271 5.5778 5.7286 5.8793 6.0301 6.1808 6.3316 6.4823 6.6331 6.7838 6.9346 7.0853 7.2361 7.3869 7.5376 7.6884 7.8391 7.9899 8.1406 8.2914 8.4421 8.5929 8.7436 8.8944 9.0451 9.1959 9.3466 9.4974 9.6481 9.7989 9.9496 10.1 10.251 10.402 10.553 10.703 10.854 11.005 11.156 11.306 11.457 11.608 11.759 11.909 12.06 12.211 12.362 12.512 12.663 12.814 12.965 13.115 13.266 13.417 13.568 13.718 13.869 14.02 14.171 14.321 14.472 14.623 14.774 14.924 15.075 15.226 15.377 15.527 15.678 15.829 15.98 16.13 16.281 16.432 16.583 16.733 16.884 17.035 17.186 17.336 17.487 17.638 17.789 17.939 18.09 18.241 18.392 18.543 18.693 18.844 18.995 19.146 19.296 19.447 19.598 19.749 19.899 20.05 20.201 20.352 20.502 20.653 20.804 20.955 21.105 21.256 21.407 21.558 21.708 21.859 22.01 22.161 22.311 22.462 22.613 22.764 22.914 23.065 23.216 23.367 23.517 23.668 23.819 23.97 24.12 24.271 24.422 24.573 24.723 24.874 25.025 25.176 25.326 25.477 25.628 25.779 25.929 26.08 26.231 26.382 26.532 26.683 26.834 26.985 27.135 27.286 27.437 27.588 27.738 27.889 28.04 28.191 28.341 28.492 28.643 28.794 28.944 29.095 29.246 29.397 29.547 29.698 29.849 30]
      | sbobj.Groups(2).Signals(3).YData = [1.2662 2.3711 2.4881 2.554 2.6028 2.6413 2.6726 2.6985 2.7203 2.7387 2.7545 2.7681 2.7799 2.7901 2.799 2.8067 2.8135 2.8194 2.8246 2.8291 2.833 2.8364 2.8393 2.8419 2.8441 2.846 2.8476 2.849 2.8502 2.8513 2.8523 2.8532 2.854 2.8547 2.8554 2.8562 2.8569 2.8577 2.8584 2.8593 2.8601 2.861 2.8619 2.8629 2.8639 2.8649 2.866 2.8671 2.8681 2.8692 2.8703 2.8714 2.8725 2.8735 2.8745 2.8755 2.8764 2.8773 2.8781 2.8789 2.8796 2.8803 2.8809 2.8815 2.882 2.8825 2.8829 2.8832 2.8835 2.8838 2.8841 2.8843 2.8844 2.8846 2.8847 2.8849 2.885 2.8851 2.8852 2.8854 2.8855 2.8857 2.8859 2.8861 2.8863 2.8866 2.8869 2.8872 2.8876 2.888 2.8884 2.8889 2.8894 2.8899 2.8905 2.891 2.8916 2.8922 2.8928 2.8934 2.8941 2.8947 2.8953 2.8959 2.8965 2.8971 2.8977 2.8982 2.8987 2.8992 2.8997 2.9001 2.9005 2.9008 2.9011 2.9014 2.9016 2.9018 2.902 2.9021 2.9022 2.9023 2.9024 2.9024 2.9024 2.9024 2.9024 2.9024 2.9024 2.9024 2.9024 2.9024 2.9025 2.9025 2.9026 2.9027 2.9029 2.903 2.9032 2.9035 2.9038 2.9041 2.9044 2.9048 2.9052 2.9056 2.906 2.9065 2.907 2.9075 2.908 2.9085 2.9089 2.9094 2.9099 2.9103 2.9107 2.9111 2.9114 2.9117 2.912 2.9122 2.9123 2.9125 2.9125 2.9126 2.9125 2.9125 2.9124 2.9123 2.9121 2.912 2.9118 2.9117 2.9115 2.9114 2.9112 2.9111 2.9111 2.9111 2.9111 2.9112 2.9113 2.9114 2.9116 2.9118 2.912 2.9122 2.9124 2.9126 2.9128 2.9128 2.9129 2.9128 2.9128 2.9127 2.9126 2.9125 2.9127 2.9131]
      | sbobj.Groups(2).TimeRange = [0 30]
  Subsystem : Subsystem
  Bus : Outport
  wires:
  Bus Creator/1 -> Bus/1
  Subsystem/3(Position Angular z) -> Bus Creator/3  "Position Angular z"
  Subsystem/2(Position Angular y) -> Bus Creator/2  "Position Angular y"
  Subsystem/1(Position Angular x) -> Bus Creator/1  "Position Angular x"
  FromWs/1 -> Subsystem/1(In1)

== system untitled/Desired Position angular [rad]1 ==
  Bus Creator : BusCreator  Tag=Bus Creator  Inputs=3
  FromWs : FromWorkspace  Tag=STV FromWs  VariableName=tuvar  SampleTime=0
      SigBuilderData=|
      | common.afterFinalStr = 'Extrapolate'
      | common.sampleTime = 0
      | dataSet(1).timeRange = [0 30]
      | dataSet(1).name = 'Position'
      | dataSet(2).timeRange = [0 30]
      | dataSet(2).name = 'Position1'
      | sbobj.Groups(1).Name = 'Position'
      | sbobj.Groups(1).Signals(1).Name = 'Position Angular x'
      | sbobj.Groups(1).Signals(1).XData = [0 0.15075 0.3015 0.45226 0.60301 0.75376 0.90451 1.0553 1.206 1.3568 1.5075 1.6583 1.809 1.9598 2.1105 2.2613 2.412 2.5628 2.7135 2.8643 3.015 3.1658 3.3165 3.4673 3.618 3.7688 3.9196 4.0703 4.2211 4.3718 4.5226 4.6733 4.8241 4.9748 5.1256 5.2763 5.4271 5.5778 5.7286 5.8793 6.0301 6.1808 6.3316 6.4823 6.6331 6.7838 6.9346 7.0853 7.2361 7.3869 7.5376 7.6884 7.8391 7.9899 8.1406 8.2914 8.4421 8.5929 8.7436 8.8944 9.0451 9.1959 9.3466 9.4974 9.6481 9.7989 9.9496 10.1 10.251 10.402 10.553 10.703 10.854 11.005 11.156 11.306 11.457 11.608 11.759 11.909 12.06 12.211 12.362 12.512 12.663 12.814 12.965 13.115 13.266 13.417 13.568 13.718 13.869 14.02 14.171 14.321 14.472 14.623 14.774 14.924 15.075 15.226 15.377 15.527 15.678 15.829 15.98 16.13 16.281 16.432 16.583 16.733 16.884 17.035 17.186 17.336 17.487 17.638 17.789 17.939 18.09 18.241 18.392 18.543 18.693 18.844 18.995 19.146 19.296 19.447 19.598 19.749 19.899 20.05 20.201 20.352 20.502 20.653 20.804 20.955 21.105 21.256 21.407 21.558 21.708 21.859 22.01 22.161 22.311 22.462 22.613 22.764 22.914 23.065 23.216 23.367 23.517 23.668 23.819 23.97 24.12 24.271 24.422 24.573 24.723 24.874 25.025 25.176 25.326 25.477 25.628 25.779 25.929 26.08 26.231 26.382 26.532 26.683 26.834 26.985 27.135 27.286 27.437 27.588 27.738 27.889 28.04 28.191 28.341 28.492 28.643 28.794 28.944 29.095 29.246 29.397 29.547 29.698 29.849 30]
      | sbobj.Groups(1).Signals(1).YData = [-1.2662 -2.371 -2.4879 -2.5537 -2.6023 -2.6406 -2.6717 -2.6974 -2.7189 -2.7372 -2.7527 -2.7661 -2.7777 -2.7877 -2.7963 -2.8039 -2.8104 -2.8161 -2.821 -2.8252 -2.8289 -2.832 -2.8346 -2.8369 -2.8388 -2.8404 -2.8417 -2.8429 -2.8438 -2.8446 -2.8453 -2.8459 -2.8464 -2.8469 -2.8474 -2.8479 -2.8484 -2.8489 -2.8495 -2.85 -2.8507 -2.8513 -2.852 -2.8528 -2.8536 -2.8544 -2.8552 -2.856 -2.8569 -2.8577 -2.8586 -2.8594 -2.8602 -2.861 -2.8617 -2.8624 -2.863 -2.8636 -2.8641 -2.8646 -2.865 -2.8654 -2.8656 -2.8659 -2.866 -2.8662 -2.8662 -2.8662 -2.8662 -2.8661 -2.866 -2.8659 -2.8657 -2.8655 -2.8653 -2.8651 -2.8649 -2.8647 -2.8645 -2.8643 -2.8641 -2.8639 -2.8638 -2.8637 -2.8636 -2.8635 -2.8635 -2.8635 -2.8635 -2.8636 -2.8637 -2.8638 -2.864 -2.8641 -2.8643 -2.8646 -2.8648 -2.865 -2.8653 -2.8655 -2.8658 -2.866 -2.8662 -2.8664 -2.8666 -2.8668 -2.8669 -2.867 -2.8671 -2.8672 -2.8672 -2.8672 -2.8671 -2.867 -2.8668 -2.8666 -2.8664 -2.8662 -2.8659 -2.8655 -2.8652 -2.8648 -2.8644 -2.864 -2.8635 -2.863 -2.8626 -2.8621 -2.8616 -2.8612 -2.8607 -2.8602 -2.8598 -2.8594 -2.859 -2.8586 -2.8582 -2.8579 -2.8576 -2.8573 -2.8571 -2.8568 -2.8566 -2.8565 -2.8563 -2.8562 -2.8561 -2.856 -2.8559 -2.8558 -2.8557 -2.8556 -2.8555 -2.8554 -2.8553 -2.8551 -2.8549 -2.8547 -2.8544 -2.8541 -2.8538 -2.8534 -2.853 -2.8525 -2.852 -2.8514 -2.8508 -2.8502 -2.8495 -2.8487 -2.8479 -2.8471 -2.8463 -2.8454 -2.8445 -2.8436 -2.8428 -2.8419 -2.841 -2.8401 -2.8393 -2.8384 -2.8376 -2.8368 -2.8361 -2.8354 -2.8347 -2.834 -2.8334 -2.8328 -2.8322 -2.8317 -2.8312 -2.8307 -2.8303 -2.8299 -2.8295 -2.8292 -2.8291 -2.8291]
      | sbobj.Groups(1).Signals(2).Name = 'Position Angular y'
      | sbobj.Groups(1).Signals(2).XData = [0 0.15075 0.3015 0.45226 0.60301 0.75376 0.90451 1.0553 1.206 1.3568 1.5075 1.6583 1.809 1.9598 2.1105 2.2613 2.412 2.5628 2.7135 2.8643 3.015 3.1658 3.3165 3.4673 3.618 3.7688 3.9196 4.0703 4.2211 4.3718 4.5226 4.6733 4.8241 4.9748 5.1256 5.2763 5.4271 5.5778 5.7286 5.8793 6.0301 6.1808 6.3316 6.4823 6.6331 6.7838 6.9346 7.0853 7.2361 7.3869 7.5376 7.6884 7.8391 7.9899 8.1406 8.2914 8.4421 8.5929 8.7436 8.8944 9.0451 9.1959 9.3466 9.4974 9.6481 9.7989 9.9496 10.1 10.251 10.402 10.553 10.703 10.854 11.005 11.156 11.306 11.457 11.608 11.759 11.909 12.06 12.211 12.362 12.512 12.663 12.814 12.965 13.115 13.266 13.417 13.568 13.718 13.869 14.02 14.171 14.321 14.472 14.623 14.774 14.924 15.075 15.226 15.377 15.527 15.678 15.829 15.98 16.13 16.281 16.432 16.583 16.733 16.884 17.035 17.186 17.336 17.487 17.638 17.789 17.939 18.09 18.241 18.392 18.543 18.693 18.844 18.995 19.146 19.296 19.447 19.598 19.749 19.899 20.05 20.201 20.352 20.502 20.653 20.804 20.955 21.105 21.256 21.407 21.558 21.708 21.859 22.01 22.161 22.311 22.462 22.613 22.764 22.914 23.065 23.216 23.367 23.517 23.668 23.819 23.97 24.12 24.271 24.422 24.573 24.723 24.874 25.025 25.176 25.326 25.477 25.628 25.779 25.929 26.08 26.231 26.382 26.532 26.683 26.834 26.985 27.135 27.286 27.437 27.588 27.738 27.889 28.04 28.191 28.341 28.492 28.643 28.794 28.944 29.095 29.246 29.397 29.547 29.698 29.849 30]
      | sbobj.Groups(1).Signals(2).YData = [-1.5708 -1.5706 -1.5699 -1.5687 -1.5669 -1.5646 -1.5618 -1.5584 -1.5546 -1.5504 -1.5458 -1.5409 -1.5358 -1.5305 -1.525 -1.5195 -1.5138 -1.5082 -1.5025 -1.4969 -1.4914 -1.4859 -1.4804 -1.4751 -1.4698 -1.4647 -1.4596 -1.4546 -1.4496 -1.4447 -1.4399 -1.4351 -1.4303 -1.4255 -1.4208 -1.416 -1.4113 -1.4065 -1.4017 -1.3969 -1.392 -1.3871 -1.3822 -1.3772 -1.3722 -1.3672 -1.3621 -1.3569 -1.3518 -1.3466 -1.3414 -1.3361 -1.3309 -1.3256 -1.3204 -1.3151 -1.3098 -1.3046 -1.2993 -1.2941 -1.2889 -1.2837 -1.2785 -1.2734 -1.2683 -1.2632 -1.2582 -1.2532 -1.2482 -1.2432 -1.2383 -1.2334 -1.2285 -1.2236 -1.2187 -1.2139 -1.2091 -1.2042 -1.1994 -1.1946 -1.1898 -1.185 -1.1801 -1.1753 -1.1704 -1.1655 -1.1606 -1.1557 -1.1508 -1.1459 -1.1409 -1.1359 -1.1309 -1.1259 -1.1209 -1.1158 -1.1108 -1.1057 -1.1006 -1.0955 -1.0904 -1.0853 -1.0802 -1.0751 -1.07 -1.065 -1.0599 -1.0549 -1.0498 -1.0448 -1.0398 -1.0348 -1.0299 -1.0249 -1.02 -1.0151 -1.0103 -1.0054 -1.0006 -0.9958 -0.99101 -0.98623 -0.98146 -0.97671 -0.97195 -0.96721 -0.96246 -0.95771 -0.95296 -0.9482 -0.94342 -0.93864 -0.93384 -0.92902 -0.92418 -0.91932 -0.91444 -0.90954 -0.90462 -0.89967 -0.8947 -0.88972 -0.88471 -0.87969 -0.87466 -0.86962 -0.86457 -0.85952 -0.85448 -0.84944 -0.8444 -0.83939 -0.83439 -0.82941 -0.82446 -0.81954 -0.81465 -0.8098 -0.80498 -0.8002 -0.79546 -0.79075 -0.78608 -0.78143 -0.77682 -0.77223 -0.76765 -0.76309 -0.75853 -0.75396 -0.74939 -0.74479 -0.74016 -0.7355 -0.73079 -0.72604 -0.72122 -0.71635 -0.71142 -0.70643 -0.70139 -0.6963 -0.69118 -0.68603 -0.68089 -0.67576 -0.6707 -0.66571 -0.66086 -0.65617 -0.65169 -0.64747 -0.64355 -0.64 -0.63685 -0.63414 -0.63191 -0.63017 -0.62894 -0.62818]
      | sbobj.Groups(1).Signals(3).Name = 'Position Angular z'
      | sbobj.Groups(1).Signals(3).XData = [0 0.15075 0.3015 0.45226 0.60301 0.75376 0.90451 1.0553 1.206 1.3568 1.5075 1.6583 1.809 1.9598 2.1105 2.2613 2.412 2.5628 2.7135 2.8643 3.015 3.1658 3.3165 3.4673 3.618 3.7688 3.9196 4.0703 4.2211 4.3718 4.5226 4.6733 4.8241 4.9748 5.1256 5.2763 5.4271 5.5778 5.7286 5.8793 6.0301 6.1808 6.3316 6.4823 6.6331 6.7838 6.9346 7.0853 7.2361 7.3869 7.5376 7.6884 7.8391 7.9899 8.1406 8.2914 8.4421 8.5929 8.7436 8.8944 9.0451 9.1959 9.3466 9.4974 9.6481 9.7989 9.9496 10.1 10.251 10.402 10.553 10.703 10.854 11.005 11.156 11.306 11.457 11.608 11.759 11.909 12.06 12.211 12.362 12.512 12.663 12.814 12.965 13.115 13.266 13.417 13.568 13.718 13.869 14.02 14.171 14.321 14.472 14.623 14.774 14.924 15.075 15.226 15.377 15.527 15.678 15.829 15.98 16.13 16.281 16.432 16.583 16.733 16.884 17.035 17.186 17.336 17.487 17.638 17.789 17.939 18.09 18.241 18.392 18.543 18.693 18.844 18.995 19.146 19.296 19.447 19.598 19.749 19.899 20.05 20.201 20.352 20.502 20.653 20.804 20.955 21.105 21.256 21.407 21.558 21.708 21.859 22.01 22.161 22.311 22.462 22.613 22.764 22.914 23.065 23.216 23.367 23.517 23.668 23.819 23.97 24.12 24.271 24.422 24.573 24.723 24.874 25.025 25.176 25.326 25.477 25.628 25.779 25.929 26.08 26.231 26.382 26.532 26.683 26.834 26.985 27.135 27.286 27.437 27.588 27.738 27.889 28.04 28.191 28.341 28.492 28.643 28.794 28.944 29.095 29.246 29.397 29.547 29.698 29.849 30]
      | sbobj.Groups(1).Signals(3).YData = [1.2662 2.3711 2.4881 2.554 2.6028 2.6413 2.6726 2.6985 2.7203 2.7387 2.7545 2.7681 2.7799 2.7901 2.799 2.8067 2.8135 2.8194 2.8246 2.8291 2.833 2.8364 2.8393 2.8419 2.8441 2.846 2.8476 2.849 2.8502 2.8513 2.8523 2.8532 2.854 2.8547 2.8554 2.8562 2.8569 2.8577 2.8584 2.8593 2.8601 2.861 2.8619 2.8629 2.8639 2.8649 2.866 2.8671 2.8681 2.8692 2.8703 2.8714 2.8725 2.8735 2.8745 2.8755 2.8764 2.8773 2.8781 2.8789 2.8796 2.8803 2.8809 2.8815 2.882 2.8825 2.8829 2.8832 2.8835 2.8838 2.8841 2.8843 2.8844 2.8846 2.8847 2.8849 2.885 2.8851 2.8852 2.8854 2.8855 2.8857 2.8859 2.8861 2.8863 2.8866 2.8869 2.8872 2.8876 2.888 2.8884 2.8889 2.8894 2.8899 2.8905 2.891 2.8916 2.8922 2.8928 2.8934 2.8941 2.8947 2.8953 2.8959 2.8965 2.8971 2.8977 2.8982 2.8987 2.8992 2.8997 2.9001 2.9005 2.9008 2.9011 2.9014 2.9016 2.9018 2.902 2.9021 2.9022 2.9023 2.9024 2.9024 2.9024 2.9024 2.9024 2.9024 2.9024 2.9024 2.9024 2.9024 2.9025 2.9025 2.9026 2.9027 2.9029 2.903 2.9032 2.9035 2.9038 2.9041 2.9044 2.9048 2.9052 2.9056 2.906 2.9065 2.907 2.9075 2.908 2.9085 2.9089 2.9094 2.9099 2.9103 2.9107 2.9111 2.9114 2.9117 2.912 2.9122 2.9123 2.9125 2.9125 2.9126 2.9125 2.9125 2.9124 2.9123 2.9121 2.912 2.9118 2.9117 2.9115 2.9114 2.9112 2.9111 2.9111 2.9111 2.9111 2.9112 2.9113 2.9114 2.9116 2.9118 2.912 2.9122 2.9124 2.9126 2.9128 2.9128 2.9129 2.9128 2.9128 2.9127 2.9126 2.9125 2.9127 2.9131]
      | sbobj.Groups(1).TimeRange = [0 30]
      | sbobj.Groups(2).Name = 'Position1'
      | sbobj.Groups(2).Signals(1).Name = 'Position Angular x'
      | sbobj.Groups(2).Signals(1).XData = [0 0.15075 0.3015 0.45226 0.60301 0.75376 0.90451 1.0553 1.206 1.3568 1.5075 1.6583 1.809 1.9598 2.1105 2.2613 2.412 2.5628 2.7135 2.8643 3.015 3.1658 3.3165 3.4673 3.618 3.7688 3.9196 4.0703 4.2211 4.3718 4.5226 4.6733 4.8241 4.9748 5.1256 5.2763 5.4271 5.5778 5.7286 5.8793 6.0301 6.1808 6.3316 6.4823 6.6331 6.7838 6.9346 7.0853 7.2361 7.3869 7.5376 7.6884 7.8391 7.9899 8.1406 8.2914 8.4421 8.5929 8.7436 8.8944 9.0451 9.1959 9.3466 9.4974 9.6481 9.7989 9.9496 10.1 10.251 10.402 10.553 10.703 10.854 11.005 11.156 11.306 11.457 11.608 11.759 11.909 12.06 12.211 12.362 12.512 12.663 12.814 12.965 13.115 13.266 13.417 13.568 13.718 13.869 14.02 14.171 14.321 14.472 14.623 14.774 14.924 15.075 15.226 15.377 15.527 15.678 15.829 15.98 16.13 16.281 16.432 16.583 16.733 16.884 17.035 17.186 17.336 17.487 17.638 17.789 17.939 18.09 18.241 18.392 18.543 18.693 18.844 18.995 19.146 19.296 19.447 19.598 19.749 19.899 20.05 20.201 20.352 20.502 20.653 20.804 20.955 21.105 21.256 21.407 21.558 21.708 21.859 22.01 22.161 22.311 22.462 22.613 22.764 22.914 23.065 23.216 23.367 23.517 23.668 23.819 23.97 24.12 24.271 24.422 24.573 24.723 24.874 25.025 25.176 25.326 25.477 25.628 25.779 25.929 26.08 26.231 26.382 26.532 26.683 26.834 26.985 27.135 27.286 27.437 27.588 27.738 27.889 28.04 28.191 28.341 28.492 28.643 28.794 28.944 29.095 29.246 29.397 29.547 29.698 29.849 30]
      | sbobj.Groups(2).Signals(1).YData = [-1.2662 -2.371 -2.4879 -2.5537 -2.6023 -2.6406 -2.6717 -2.6974 -2.7189 -2.7372 -2.7527 -2.7661 -2.7777 -2.7877 -2.7963 -2.8039 -2.8104 -2.8161 -2.821 -2.8252 -2.8289 -2.832 -2.8346 -2.8369 -2.8388 -2.8404 -2.8417 -2.8429 -2.8438 -2.8446 -2.8453 -2.8459 -2.8464 -2.8469 -2.8474 -2.8479 -2.8484 -2.8489 -2.8495 -2.85 -2.8507 -2.8513 -2.852 -2.8528 -2.8536 -2.8544 -2.8552 -2.856 -2.8569 -2.8577 -2.8586 -2.8594 -2.8602 -2.861 -2.8617 -2.8624 -2.863 -2.8636 -2.8641 -2.8646 -2.865 -2.8654 -2.8656 -2.8659 -2.866 -2.8662 -2.8662 -2.8662 -2.8662 -2.8661 -2.866 -2.8659 -2.8657 -2.8655 -2.8653 -2.8651 -2.8649 -2.8647 -2.8645 -2.8643 -2.8641 -2.8639 -2.8638 -2.8637 -2.8636 -2.8635 -2.8635 -2.8635 -2.8635 -2.8636 -2.8637 -2.8638 -2.864 -2.8641 -2.8643 -2.8646 -2.8648 -2.865 -2.8653 -2.8655 -2.8658 -2.866 -2.8662 -2.8664 -2.8666 -2.8668 -2.8669 -2.867 -2.8671 -2.8672 -2.8672 -2.8672 -2.8671 -2.867 -2.8668 -2.8666 -2.8664 -2.8662 -2.8659 -2.8655 -2.8652 -2.8648 -2.8644 -2.864 -2.8635 -2.863 -2.8626 -2.8621 -2.8616 -2.8612 -2.8607 -2.8602 -2.8598 -2.8594 -2.859 -2.8586 -2.8582 -2.8579 -2.8576 -2.8573 -2.8571 -2.8568 -2.8566 -2.8565 -2.8563 -2.8562 -2.8561 -2.856 -2.8559 -2.8558 -2.8557 -2.8556 -2.8555 -2.8554 -2.8553 -2.8551 -2.8549 -2.8547 -2.8544 -2.8541 -2.8538 -2.8534 -2.853 -2.8525 -2.852 -2.8514 -2.8508 -2.8502 -2.8495 -2.8487 -2.8479 -2.8471 -2.8463 -2.8454 -2.8445 -2.8436 -2.8428 -2.8419 -2.841 -2.8401 -2.8393 -2.8384 -2.8376 -2.8368 -2.8361 -2.8354 -2.8347 -2.834 -2.8334 -2.8328 -2.8322 -2.8317 -2.8312 -2.8307 -2.8303 -2.8299 -2.8295 -2.8292 -2.8291 -2.8291]
      | sbobj.Groups(2).Signals(2).Name = 'Position Angular y'
      | sbobj.Groups(2).Signals(2).XData = [0 0.15075 0.3015 0.45226 0.60301 0.75376 0.90451 1.0553 1.206 1.3568 1.5075 1.6583 1.809 1.9598 2.1105 2.2613 2.412 2.5628 2.7135 2.8643 3.015 3.1658 3.3165 3.4673 3.618 3.7688 3.9196 4.0703 4.2211 4.3718 4.5226 4.6733 4.8241 4.9748 5.1256 5.2763 5.4271 5.5778 5.7286 5.8793 6.0301 6.1808 6.3316 6.4823 6.6331 6.7838 6.9346 7.0853 7.2361 7.3869 7.5376 7.6884 7.8391 7.9899 8.1406 8.2914 8.4421 8.5929 8.7436 8.8944 9.0451 9.1959 9.3466 9.4974 9.6481 9.7989 9.9496 10.1 10.251 10.402 10.553 10.703 10.854 11.005 11.156 11.306 11.457 11.608 11.759 11.909 12.06 12.211 12.362 12.512 12.663 12.814 12.965 13.115 13.266 13.417 13.568 13.718 13.869 14.02 14.171 14.321 14.472 14.623 14.774 14.924 15.075 15.226 15.377 15.527 15.678 15.829 15.98 16.13 16.281 16.432 16.583 16.733 16.884 17.035 17.186 17.336 17.487 17.638 17.789 17.939 18.09 18.241 18.392 18.543 18.693 18.844 18.995 19.146 19.296 19.447 19.598 19.749 19.899 20.05 20.201 20.352 20.502 20.653 20.804 20.955 21.105 21.256 21.407 21.558 21.708 21.859 22.01 22.161 22.311 22.462 22.613 22.764 22.914 23.065 23.216 23.367 23.517 23.668 23.819 23.97 24.12 24.271 24.422 24.573 24.723 24.874 25.025 25.176 25.326 25.477 25.628 25.779 25.929 26.08 26.231 26.382 26.532 26.683 26.834 26.985 27.135 27.286 27.437 27.588 27.738 27.889 28.04 28.191 28.341 28.492 28.643 28.794 28.944 29.095 29.246 29.397 29.547 29.698 29.849 30]
      | sbobj.Groups(2).Signals(2).YData = [-1.5708 -1.5706 -1.5699 -1.5687 -1.5669 -1.5646 -1.5618 -1.5584 -1.5546 -1.5504 -1.5458 -1.5409 -1.5358 -1.5305 -1.525 -1.5195 -1.5138 -1.5082 -1.5025 -1.4969 -1.4914 -1.4859 -1.4804 -1.4751 -1.4698 -1.4647 -1.4596 -1.4546 -1.4496 -1.4447 -1.4399 -1.4351 -1.4303 -1.4255 -1.4208 -1.416 -1.4113 -1.4065 -1.4017 -1.3969 -1.392 -1.3871 -1.3822 -1.3772 -1.3722 -1.3672 -1.3621 -1.3569 -1.3518 -1.3466 -1.3414 -1.3361 -1.3309 -1.3256 -1.3204 -1.3151 -1.3098 -1.3046 -1.2993 -1.2941 -1.2889 -1.2837 -1.2785 -1.2734 -1.2683 -1.2632 -1.2582 -1.2532 -1.2482 -1.2432 -1.2383 -1.2334 -1.2285 -1.2236 -1.2187 -1.2139 -1.2091 -1.2042 -1.1994 -1.1946 -1.1898 -1.185 -1.1801 -1.1753 -1.1704 -1.1655 -1.1606 -1.1557 -1.1508 -1.1459 -1.1409 -1.1359 -1.1309 -1.1259 -1.1209 -1.1158 -1.1108 -1.1057 -1.1006 -1.0955 -1.0904 -1.0853 -1.0802 -1.0751 -1.07 -1.065 -1.0599 -1.0549 -1.0498 -1.0448 -1.0398 -1.0348 -1.0299 -1.0249 -1.02 -1.0151 -1.0103 -1.0054 -1.0006 -0.9958 -0.99101 -0.98623 -0.98146 -0.97671 -0.97195 -0.96721 -0.96246 -0.95771 -0.95296 -0.9482 -0.94342 -0.93864 -0.93384 -0.92902 -0.92418 -0.91932 -0.91444 -0.90954 -0.90462 -0.89967 -0.8947 -0.88972 -0.88471 -0.87969 -0.87466 -0.86962 -0.86457 -0.85952 -0.85448 -0.84944 -0.8444 -0.83939 -0.83439 -0.82941 -0.82446 -0.81954 -0.81465 -0.8098 -0.80498 -0.8002 -0.79546 -0.79075 -0.78608 -0.78143 -0.77682 -0.77223 -0.76765 -0.76309 -0.75853 -0.75396 -0.74939 -0.74479 -0.74016 -0.7355 -0.73079 -0.72604 -0.72122 -0.71635 -0.71142 -0.70643 -0.70139 -0.6963 -0.69118 -0.68603 -0.68089 -0.67576 -0.6707 -0.66571 -0.66086 -0.65617 -0.65169 -0.64747 -0.64355 -0.64 -0.63685 -0.63414 -0.63191 -0.63017 -0.62894 -0.62818]
      | sbobj.Groups(2).Signals(3).Name = 'Position Angular z'
      | sbobj.Groups(2).Signals(3).XData = [0 0.15075 0.3015 0.45226 0.60301 0.75376 0.90451 1.0553 1.206 1.3568 1.5075 1.6583 1.809 1.9598 2.1105 2.2613 2.412 2.5628 2.7135 2.8643 3.015 3.1658 3.3165 3.4673 3.618 3.7688 3.9196 4.0703 4.2211 4.3718 4.5226 4.6733 4.8241 4.9748 5.1256 5.2763 5.4271 5.5778 5.7286 5.8793 6.0301 6.1808 6.3316 6.4823 6.6331 6.7838 6.9346 7.0853 7.2361 7.3869 7.5376 7.6884 7.8391 7.9899 8.1406 8.2914 8.4421 8.5929 8.7436 8.8944 9.0451 9.1959 9.3466 9.4974 9.6481 9.7989 9.9496 10.1 10.251 10.402 10.553 10.703 10.854 11.005 11.156 11.306 11.457 11.608 11.759 11.909 12.06 12.211 12.362 12.512 12.663 12.814 12.965 13.115 13.266 13.417 13.568 13.718 13.869 14.02 14.171 14.321 14.472 14.623 14.774 14.924 15.075 15.226 15.377 15.527 15.678 15.829 15.98 16.13 16.281 16.432 16.583 16.733 16.884 17.035 17.186 17.336 17.487 17.638 17.789 17.939 18.09 18.241 18.392 18.543 18.693 18.844 18.995 19.146 19.296 19.447 19.598 19.749 19.899 20.05 20.201 20.352 20.502 20.653 20.804 20.955 21.105 21.256 21.407 21.558 21.708 21.859 22.01 22.161 22.311 22.462 22.613 22.764 22.914 23.065 23.216 23.367 23.517 23.668 23.819 23.97 24.12 24.271 24.422 24.573 24.723 24.874 25.025 25.176 25.326 25.477 25.628 25.779 25.929 26.08 26.231 26.382 26.532 26.683 26.834 26.985 27.135 27.286 27.437 27.588 27.738 27.889 28.04 28.191 28.341 28.492 28.643 28.794 28.944 29.095 29.246 29.397 29.547 29.698 29.849 30]
      | sbobj.Groups(2).Signals(3).YData = [1.2662 2.3711 2.4881 2.554 2.6028 2.6413 2.6726 2.6985 2.7203 2.7387 2.7545 2.7681 2.7799 2.7901 2.799 2.8067 2.8135 2.8194 2.8246 2.8291 2.833 2.8364 2.8393 2.8419 2.8441 2.846 2.8476 2.849 2.8502 2.8513 2.8523 2.8532 2.854 2.8547 2.8554 2.8562 2.8569 2.8577 2.8584 2.8593 2.8601 2.861 2.8619 2.8629 2.8639 2.8649 2.866 2.8671 2.8681 2.8692 2.8703 2.8714 2.8725 2.8735 2.8745 2.8755 2.8764 2.8773 2.8781 2.8789 2.8796 2.8803 2.8809 2.8815 2.882 2.8825 2.8829 2.8832 2.8835 2.8838 2.8841 2.8843 2.8844 2.8846 2.8847 2.8849 2.885 2.8851 2.8852 2.8854 2.8855 2.8857 2.8859 2.8861 2.8863 2.8866 2.8869 2.8872 2.8876 2.888 2.8884 2.8889 2.8894 2.8899 2.8905 2.891 2.8916 2.8922 2.8928 2.8934 2.8941 2.8947 2.8953 2.8959 2.8965 2.8971 2.8977 2.8982 2.8987 2.8992 2.8997 2.9001 2.9005 2.9008 2.9011 2.9014 2.9016 2.9018 2.902 2.9021 2.9022 2.9023 2.9024 2.9024 2.9024 2.9024 2.9024 2.9024 2.9024 2.9024 2.9024 2.9024 2.9025 2.9025 2.9026 2.9027 2.9029 2.903 2.9032 2.9035 2.9038 2.9041 2.9044 2.9048 2.9052 2.9056 2.906 2.9065 2.907 2.9075 2.908 2.9085 2.9089 2.9094 2.9099 2.9103 2.9107 2.9111 2.9114 2.9117 2.912 2.9122 2.9123 2.9125 2.9125 2.9126 2.9125 2.9125 2.9124 2.9123 2.9121 2.912 2.9118 2.9117 2.9115 2.9114 2.9112 2.9111 2.9111 2.9111 2.9111 2.9112 2.9113 2.9114 2.9116 2.9118 2.912 2.9122 2.9124 2.9126 2.9128 2.9128 2.9129 2.9128 2.9128 2.9127 2.9126 2.9125 2.9127 2.9131]
      | sbobj.Groups(2).TimeRange = [0 30]
  Subsystem : Subsystem
  Bus : Outport
  wires:
  Bus Creator/1 -> Bus/1
  Subsystem/3(Position Angular z) -> Bus Creator/3  "Position Angular z"
  Subsystem/2(Position Angular y) -> Bus Creator/2  "Position Angular y"
  Subsystem/1(Position Angular x) -> Bus Creator/1  "Position Angular x"
  FromWs/1 -> Subsystem/1(In1)

== system untitled/Signal Builder ==
  Bus Creator : BusCreator  Tag=Bus Creator  Inputs=6
  FromWs : FromWorkspace  Tag=STV FromWs  VariableName=tuvar  SampleTime=0
      SigBuilderData=|
      | common.afterFinalStr = 'Extrapolate'
      | common.sampleTime = 0
      | dataSet.timeRange = [0 30]
      | dataSet.name = 'Desired Velocities'
      | sbobj.Groups.Name = 'Desired Velocities'
      | sbobj.Groups.Signals(1).Name = 'Velocity Angular x'
      | sbobj.Groups.Signals(1).XData = [0 0.15075 0.3015 0.45226 0.60301 0.75376 0.90451 1.0553 1.206 1.3568 1.5075 1.6583 1.809 1.9598 2.1105 2.2613 2.412 2.5628 2.7135 2.8643 3.015 3.1658 3.3165 3.4673 3.618 3.7688 3.9196 4.0703 4.2211 4.3718 4.5226 4.6733 4.8241 4.9748 5.1256 5.2763 5.4271 5.5778 5.7286 5.8793 6.0301 6.1808 6.3316 6.4823 6.6331 6.7838 6.9346 7.0853 7.2361 7.3869 7.5376 7.6884 7.8391 7.9899 8.1406 8.2914 8.4421 8.5929 8.7436 8.8944 9.0451 9.1959 9.3466 9.4974 9.6481 9.7989 9.9496 10.1 10.251 10.402 10.553 10.703 10.854 11.005 11.156 11.306 11.457 11.608 11.759 11.909 12.06 12.211 12.362 12.512 12.663 12.814 12.965 13.115 13.266 13.417 13.568 13.718 13.869 14.02 14.171 14.321 14.472 14.623 14.774 14.924 15.075 15.226 15.377 15.527 15.678 15.829 15.98 16.13 16.281 16.432 16.583 16.733 16.884 17.035 17.186 17.336 17.487 17.638 17.789 17.939 18.09 18.241 18.392 18.543 18.693 18.844 18.995 19.146 19.296 19.447 19.598 19.749 19.899 20.05 20.201 20.352 20.502 20.653 20.804 20.955 21.105 21.256 21.407 21.558 21.708 21.859 22.01 22.161 22.311 22.462 22.613 22.764 22.914 23.065 23.216 23.367 23.517 23.668 23.819 23.97 24.12 24.271 24.422 24.573 24.723 24.874 25.025 25.176 25.326 25.477 25.628 25.779 25.929 26.08 26.231 26.382 26.532 26.683 26.834 26.985 27.135 27.286 27.437 27.588 27.738 27.889 28.04 28.191 28.341 28.492 28.643 28.794 28.944 29.095 29.246 29.397 29.547 29.698 29.849 30]
      | sbobj.Groups.Signals(1).YData = [0 -0.0018068 -0.0034031 -0.0047915 -0.0059792 -0.0069775 -0.0078002 -0.0084629 -0.0089823 -0.0093754 -0.0096591 -0.0098495 ... (200 elements, 1x200)]
      | sbobj.Groups.Signals(2).Name = 'Velocity Angular y'
      | sbobj.Groups.Signals(2).XData = [0 0.15075 0.3015 0.45226 0.60301 0.75376 0.90451 1.0553 1.206 1.3568 1.5075 1.6583 1.809 1.9598 2.1105 2.2613 2.412 2.5628 2.7135 2.8643 3.015 3.1658 3.3165 3.4673 3.618 3.7688 3.9196 4.0703 4.2211 4.3718 4.5226 4.6733 4.8241 4.9748 5.1256 5.2763 5.4271 5.5778 5.7286 5.8793 6.0301 6.1808 6.3316 6.4823 6.6331 6.7838 6.9346 7.0853 7.2361 7.3869 7.5376 7.6884 7.8391 7.9899 8.1406 8.2914 8.4421 8.5929 8.7436 8.8944 9.0451 9.1959 9.3466 9.4974 9.6481 9.7989 9.9496 10.1 10.251 10.402 10.553 10.703 10.854 11.005 11.156 11.306 11.457 11.608 11.759 11.909 12.06 12.211 12.362 12.512 12.663 12.814 12.965 13.115 13.266 13.417 13.568 13.718 13.869 14.02 14.171 14.321 14.472 14.623 14.774 14.924 15.075 15.226 15.377 15.527 15.678 15.829 15.98 16.13 16.281 16.432 16.583 16.733 16.884 17.035 17.186 17.336 17.487 17.638 17.789 17.939 18.09 18.241 18.392 18.543 18.693 18.844 18.995 19.146 19.296 19.447 19.598 19.749 19.899 20.05 20.201 20.352 20.502 20.653 20.804 20.955 21.105 21.256 21.407 21.558 21.708 21.859 22.01 22.161 22.311 22.462 22.613 22.764 22.914 23.065 23.216 23.367 23.517 23.668 23.819 23.97 24.12 24.271 24.422 24.573 24.723 24.874 25.025 25.176 25.326 25.477 25.628 25.779 25.929 26.08 26.231 26.382 26.532 26.683 26.834 26.985 27.135 27.286 27.437 27.588 27.738 27.889 28.04 28.191 28.341 28.492 28.643 28.794 28.944 29.095 29.246 29.397 29.547 29.698 29.849 30]
      | sbobj.Groups.Signals(2).YData = [0 -0.0022666 -0.0052246 -0.00859 -0.012137 -0.01569 -0.019115 -0.022315 -0.025222 -0.027794 -0.030007 -0.031856 -0.033348 -0.0345 -0.035335 -0.035883 -0.036178 -0.036253 -0.036144 -0.035884 -0.035509 -0.035047 -0.03453 -0.033981 -0.033425 -0.032881 -0.032366 -0.031893 -0.031474 -0.031115 -0.030823 -0.0306 -0.030446 -0.03036 -0.030339 -0.03038 -0.030476 -0.030621 -0.030809 -0.031031 -0.03128 -0.031549 -0.031829 -0.032114 -0.032396 -0.03267 -0.032929 -0.033168 -0.033383 -0.033571 -0.033727 -0.033851 -0.03394 -0.033995 -0.034015 -0.034001 -0.033954 -0.033876 -0.03377 -0.033638 -0.033484 -0.033311 -0.033123 -0.032923 -0.032715 -0.032504 -0.032292 -0.032084 -0.031883 -0.031691 -0.031513 -0.031351 -0.031207 -0.031082 -0.030979 -0.030899 -0.030841 -0.030808 -0.030797 -0.03081 -0.030845 -0.0309 -0.030975 -0.031068 -0.031176 -0.031297 -0.031429 -0.031568 -0.031714 -0.031861 -0.032009 -0.032154 -0.032293 -0.032425 -0.032546 -0.032654 -0.032747 -0.032824 -0.032884 -0.032924 -0.032945 -0.032945 -0.032924 -0.032883 -0.032822 -0.032742 -0.032644 -0.032528 -0.032398 -0.032254 -0.0321 -0.031936 -0.031767 -0.031593 -0.031419 -0.031246 -0.031078 -0.030917 -0.030765 -0.030626 -0.030501 -0.030393 -0.030302 -0.030232 -0.030182 -0.030155 -0.03015 -0.030167 -0.030207 -0.030268 -0.030351 -0.030452 -0.030571 -0.030705 -0.030852 -0.031009 -0.031172 -0.03134 -0.031507 -0.031672 -0.031829 -0.031975 -0.032108 -0.032222 -0.032316 -0.032386 -0.03243 -0.032445 -0.03243 -0.032383 -0.032304 -0.032194 -0.032052 -0.03188 -0.03168 -0.031456 -0.03121 -0.030948 -0.030673 -0.030391 -0.030109 -0.029833 -0.029569 -0.029325 -0.029107 -0.028922 -0.028776 -0.028675 -0.028625 -0.028629 -0.028689 -0.028808 -0.028985 -0.029218 -0.029501 -0.029828 -0.030189 -0.030572 -0.030961 -0.03134 -0.031686 -0.031977 -0.032187 -0.032287 -0.032248 -0.032039 -0.03163 -0.03099 -0.03009 -0.028908 -0.027423 -0.025625 -0.023511 -0.021094 -0.018401 -0.015482 -0.012411 -0.0092907 -0.0062639 -0.0035154]
      | sbobj.Groups.Signals(3).Name = 'Velocity Angular z'
      | sbobj.Groups.Signals(3).XData = [0 0.15075 0.3015 0.45226 0.60301 0.75376 0.90451 1.0553 1.206 1.3568 1.5075 1.6583 1.809 1.9598 2.1105 2.2613 2.412 2.5628 2.7135 2.8643 3.015 3.1658 3.3165 3.4673 3.618 3.7688 3.9196 4.0703 4.2211 4.3718 4.5226 4.6733 4.8241 4.9748 5.1256 5.2763 5.4271 5.5778 5.7286 5.8793 6.0301 6.1808 6.3316 6.4823 6.6331 6.7838 6.9346 7.0853 7.2361 7.3869 7.5376 7.6884 7.8391 7.9899 8.1406 8.2914 8.4421 8.5929 8.7436 8.8944 9.0451 9.1959 9.3466 9.4974 9.6481 9.7989 9.9496 10.1 10.251 10.402 10.553 10.703 10.854 11.005 11.156 11.306 11.457 11.608 11.759 11.909 12.06 12.211 12.362 12.512 12.663 12.814 12.965 13.115 13.266 13.417 13.568 13.718 13.869 14.02 14.171 14.321 14.472 14.623 14.774 14.924 15.075 15.226 15.377 15.527 15.678 15.829 15.98 16.13 16.281 16.432 16.583 16.733 16.884 17.035 17.186 17.336 17.487 17.638 17.789 17.939 18.09 18.241 18.392 18.543 18.693 18.844 18.995 19.146 19.296 19.447 19.598 19.749 19.899 20.05 20.201 20.352 20.502 20.653 20.804 20.955 21.105 21.256 21.407 21.558 21.708 21.859 22.01 22.161 22.311 22.462 22.613 22.764 22.914 23.065 23.216 23.367 23.517 23.668 23.819 23.97 24.12 24.271 24.422 24.573 24.723 24.874 25.025 25.176 25.326 25.477 25.628 25.779 25.929 26.08 26.231 26.382 26.532 26.683 26.834 26.985 27.135 27.286 27.437 27.588 27.738 27.889 28.04 28.191 28.341 28.492 28.643 28.794 28.944 29.095 29.246 29.397 29.547 29.698 29.849 30]
      | sbobj.Groups.Signals(3).YData = [0 0.00054192 0.00090485 0.0011364 0.0012753 0.0013522 0.0013906 0.0014082 0.0014177 0.0014277 0.0014432 0.0014672 0.0015001 0.0015414 0.0015895 0.001642 0.0016966 0.0017508 0.0018022 0.0018487 0.0018887 0.0019208 0.0019441 0.0019583 0.0019633 0.0019593 0.001947 0.0019273 0.0019012 0.0018699 0.0018349 0.0017974 0.0017589 0.0017206 0.0016839 0.00165 0.0016199 0.0015945 0.0015747 0.0015609 0.0015536 0.0015531 0.0015594 0.0015725 0.0015921 0.0016179 0.0016494 0.0016859 0.0017267 0.0017711 0.0018181 0.001867 0.0019168 0.0019667 0.0020158 0.0020633 0.0021083 0.0021503 0.0021887 0.0022228 0.0022524 0.002277 0.0022966 0.0023111 0.0023205 0.0023249 0.0023247 0.00232 0.0023115 0.0022996 0.0022848 0.0022678 0.0022493 0.0022298 0.0022102 0.0021911 0.0021732 0.0021571 0.0021435 0.0021328 0.0021257 0.0021224 0.0021234 0.002129 0.0021392 0.0021543 0.0021741 0.0021987 0.0022277 0.002261 0.0022981 0.0023387 0.0023823 0.0024282 0.0024759 0.0025248 0.0025741 0.0026231 0.0026711 0.0027175 0.0027615 0.0028026 0.0028401 0.0028734 0.0029022 0.002926 0.0029445 0.0029574 0.0029648 0.0029665 0.0029626 0.0029534 0.0029392 0.0029204 0.0028976 0.0028712 0.0028421 0.0028109 0.0027786 0.0027459 0.0027139 0.0026834 0.0026554 0.0026307 0.0026103 0.0025949 0.0025854 0.0025824 0.0025864 0.0025979 0.0026171 0.0026444 0.0026796 0.0027226 0.0027731 0.0028305 0.0028943 0.0029636 0.0030374 0.0031146 0.0031939 0.003274 0.0033534 0.0034307 0.0035042 0.0035724 0.0036338 0.003687 0.0037306 0.0037634 0.0037843 0.0037926 0.0037877 0.0037693 0.0037375 0.0036926 0.0036354 0.0035669 0.0034886 0.0034024 0.0033103 0.003215 0.0031191 0.0030257 0.002938 0.0028593 0.0027928 0.0027418 0.0027093 0.002698 0.0027102 0.0027474 0.0028108 0.0029002 0.0030149 0.0031528 0.0033106 0.0034836 0.0036659 0.0038501 0.0040275 0.004188 0.0043207 0.0044139 0.0044556 0.0044343 0.0043395 0.004163 0.0038999 0.0035504 0.0031216 0.0026293 0.0021014 0.0015799 0.0011252 0.00081917 0.00077016 0.0011172 0.0020355 0.0037422]
      | sbobj.Groups.Signals(4).Name = 'Velocity Linear x'
      | sbobj.Groups.Signals(4).XData = [0 0.15075 0.3015 0.45226 0.60301 0.75376 0.90451 1.0553 1.206 1.3568 1.5075 1.6583 1.809 1.9598 2.1105 2.2613 2.412 2.5628 2.7135 2.8643 3.015 3.1658 3.3165 3.4673 3.618 3.7688 3.9196 4.0703 4.2211 4.3718 4.5226 4.6733 4.8241 4.9748 5.1256 5.2763 5.4271 5.5778 5.7286 5.8793 6.0301 6.1808 6.3316 6.4823 6.6331 6.7838 6.9346 7.0853 7.2361 7.3869 7.5376 7.6884 7.8391 7.9899 8.1406 8.2914 8.4421 8.5929 8.7436 8.8944 9.0451 9.1959 9.3466 9.4974 9.6481 9.7989 9.9496 10.1 10.251 10.402 10.553 10.703 10.854 11.005 11.156 11.306 11.457 11.608 11.759 11.909 12.06 12.211 12.362 12.512 12.663 12.814 12.965 13.115 13.266 13.417 13.568 13.718 13.869 14.02 14.171 14.321 14.472 14.623 14.774 14.924 15.075 15.226 15.377 15.527 15.678 15.829 15.98 16.13 16.281 16.432 16.583 16.733 16.884 17.035 17.186 17.336 17.487 17.638 17.789 17.939 18.09 18.241 18.392 18.543 18.693 18.844 18.995 19.146 19.296 19.447 19.598 19.749 19.899 20.05 20.201 20.352 20.502 20.653 20.804 20.955 21.105 21.256 21.407 21.558 21.708 21.859 22.01 22.161 22.311 22.462 22.613 22.764 22.914 23.065 23.216 23.367 23.517 23.668 23.819 23.97 24.12 24.271 24.422 24.573 24.723 24.874 25.025 25.176 25.326 25.477 25.628 25.779 25.929 26.08 26.231 26.382 26.532 26.683 26.834 26.985 27.135 27.286 27.437 27.588 27.738 27.889 28.04 28.191 28.341 28.492 28.643 28.794 28.944 29.095 29.246 29.397 29.547 29.698 29.849 30]
      | sbobj.Groups.Signals(4).YData = [0 -0.0006469 -0.0019071 -0.0035651 -0.0054557 -0.0074534 -0.0094641 -0.011418 -0.013264 -0.014968 -0.016506 -0.017863 -0.019035 -0.020023 -0.020833 -0.021476 -0.021966 -0.02232 -0.022557 -0.022697 -0.022759 -0.022763 -0.022728 -0.022671 -0.022609 -0.022555 -0.022522 -0.022521 -0.022558 -0.02264 -0.022772 -0.022955 -0.023189 -0.023475 -0.023809 -0.024188 -0.024608 -0.025064 -0.02555 -0.026061 -0.026589 -0.02713 -0.027676 -0.028222 -0.028762 -0.029291 -0.029804 -0.030297 -0.030766 -0.031209 -0.031623 -0.032005 -0.032356 -0.032674 -0.03296 -0.033215 -0.03344 -0.033636 -0.033807 -0.033954 -0.034082 -0.034192 -0.034289 -0.034376 -0.034457 -0.034536 -0.034615 -0.034699 -0.034791 -0.034894 -0.03501 -0.035143 -0.035293 -0.035464 -0.035655 -0.035868 -0.036104 -0.036362 -0.036642 -0.036943 -0.037265 -0.037606 -0.037963 -0.038336 -0.038721 -0.039117 -0.03952 -0.039927 -0.040337 -0.040745 -0.04115 -0.041547 -0.041935 -0.042311 -0.042672 -0.043016 -0.043342 -0.043646 -0.043929 -0.044189 -0.044425 -0.044637 -0.044825 -0.044989 -0.04513 -0.045249 -0.045347 -0.045426 -0.045488 -0.045535 -0.045571 -0.045597 -0.045616 -0.045632 -0.045648 -0.045666 -0.04569 -0.045723 -0.045767 -0.045826 -0.045901 -0.045996 -0.046112 -0.04625 -0.046413 -0.0466 -0.046812 -0.04705 -0.047312 -0.047598 -0.047906 -0.048235 -0.048583 -0.048946 -0.049321 -0.049706 -0.050096 -0.050487 -0.050876 -0.051258 -0.051628 -0.051983 -0.052317 -0.052628 -0.05291 -0.053161 -0.053377 -0.053556 -0.053695 -0.053793 -0.053849 -0.053863 -0.053836 -0.053769 -0.053666 -0.053528 -0.053361 -0.05317 -0.052961 -0.05274 -0.052515 -0.052294 -0.052085 -0.051898 -0.05174 -0.051621 -0.051549 -0.051533 -0.051579 -0.051693 -0.051881 -0.052144 -0.052484 -0.0529 -0.053387 -0.053937 -0.054541 -0.055183 -0.055845 -0.056505 -0.057135 -0.057702 -0.058171 -0.0585 -0.058641 -0.058545 -0.058156 -0.057415 -0.05626 -0.054628 -0.052453 -0.049672 -0.046224 -0.042053 -0.037109 -0.031354 -0.024763 -0.017327 -0.0090607 9.2466e-16]
      | sbobj.Groups.Signals(5).Name = 'Velocity Linear y'
      | sbobj.Groups.Signals(5).XData = [0 0.15075 0.3015 0.45226 0.60301 0.75376 0.90451 1.0553 1.206 1.3568 1.5075 1.6583 1.809 1.9598 2.1105 2.2613 2.412 2.5628 2.7135 2.8643 3.015 3.1658 3.3165 3.4673 3.618 3.7688 3.9196 4.0703 4.2211 4.3718 4.5226 4.6733 4.8241 4.9748 5.1256 5.2763 5.4271 5.5778 5.7286 5.8793 6.0301 6.1808 6.3316 6.4823 6.6331 6.7838 6.9346 7.0853 7.2361 7.3869 7.5376 7.6884 7.8391 7.9899 8.1406 8.2914 8.4421 8.5929 8.7436 8.8944 9.0451 9.1959 9.3466 9.4974 9.6481 9.7989 9.9496 10.1 10.251 10.402 10.553 10.703 10.854 11.005 11.156 11.306 11.457 11.608 11.759 11.909 12.06 12.211 12.362 12.512 12.663 12.814 12.965 13.115 13.266 13.417 13.568 13.718 13.869 14.02 14.171 14.321 14.472 14.623 14.774 14.924 15.075 15.226 15.377 15.527 15.678 15.829 15.98 16.13 16.281 16.432 16.583 16.733 16.884 17.035 17.186 17.336 17.487 17.638 17.789 17.939 18.09 18.241 18.392 18.543 18.693 18.844 18.995 19.146 19.296 19.447 19.598 19.749 19.899 20.05 20.201 20.352 20.502 20.653 20.804 20.955 21.105 21.256 21.407 21.558 21.708 21.859 22.01 22.161 22.311 22.462 22.613 22.764 22.914 23.065 23.216 23.367 23.517 23.668 23.819 23.97 24.12 24.271 24.422 24.573 24.723 24.874 25.025 25.176 25.326 25.477 25.628 25.779 25.929 26.08 26.231 26.382 26.532 26.683 26.834 26.985 27.135 27.286 27.437 27.588 27.738 27.889 28.04 28.191 28.341 28.492 28.643 28.794 28.944 29.095 29.246 29.397 29.547 29.698 29.849 30]
      | sbobj.Groups.Signals(5).YData = [0 0.0019316 0.0034825 0.0047149 0.0056861 0.0064464 0.0070393 0.007501 0.0078612 0.0081436 0.0083667 0.0085448 0.0086886 0.008806 0.0089029 0.0089833 0.0090503 0.009106 0.0091518 0.009189 0.0092184 0.0092408 0.0092568 0.0092671 0.0092721 0.0092726 0.0092691 0.0092623 0.0092527 0.009241 0.009228 0.0092142 0.0092004 0.0091874 0.0091758 0.0091665 0.0091601 0.0091573 0.009159 0.0091657 0.0091781 0.0091968 0.0092222 0.0092549 0.009295 0.0093429 0.0093987 0.0094623 0.0095338 0.0096129 0.0096992 0.0097925 0.0098921 0.0099974 0.010108 0.010223 0.010341 0.010462 0.010585 0.010708 0.010832 0.010954 0.011075 0.011193 0.011307 0.011417 0.011522 0.011621 0.011714 0.011799 0.011878 0.011949 0.012012 0.012067 0.012114 0.012153 0.012184 0.012207 0.012223 0.012232 0.012235 0.012233 0.012225 0.012213 0.012197 0.012179 0.012159 0.012138 0.012117 0.012098 0.012081 0.012066 0.012056 0.012051 0.012051 0.012058 0.012073 0.012095 0.012125 0.012165 0.012214 0.012273 0.012341 0.012419 0.012506 0.012603 0.012709 0.012823 0.012946 0.013075 0.013211 0.013353 0.013499 0.013649 0.013802 0.013955 0.014109 0.014261 0.01441 0.014556 0.014697 0.014832 0.014959 0.015077 0.015186 0.015285 0.015372 0.015448 0.015511 0.015561 0.015598 0.015622 0.015633 0.015632 0.015619 0.015594 0.015559 0.015514 0.015461 0.015402 0.015337 0.015269 0.015199 0.015129 0.015062 0.014999 0.014943 0.014895 0.014858 0.014834 0.014825 0.014833 0.01486 0.014906 0.014974 0.015065 0.015179 0.015317 0.01548 0.015667 0.015877 0.01611 0.016365 0.01664 0.016933 0.017241 0.017561 0.017891 0.018227 0.018564 0.018899 0.019228 0.019544 0.019845 0.020125 0.020378 0.0206 0.020786 0.02093 0.021027 0.021072 0.021059 0.020983 0.020838 0.020618 0.020316 0.019926 0.019438 0.018845 0.018135 0.017296 0.016314 0.01517 0.013843 0.012306 0.010527 0.0084644 0.0060676 0.0032728 -5.8634e-16]
      | sbobj.Groups.Signals(6).Name = 'Velocity Linear z'
      | sbobj.Groups.Signals(6).XData = [0 0.15075 0.3015 0.45226 0.60301 0.75376 0.90451 1.0553 1.206 1.3568 1.5075 1.6583 1.809 1.9598 2.1105 2.2613 2.412 2.5628 2.7135 2.8643 3.015 3.1658 3.3165 3.4673 3.618 3.7688 3.9196 4.0703 4.2211 4.3718 4.5226 4.6733 4.8241 4.9748 5.1256 5.2763 5.4271 5.5778 5.7286 5.8793 6.0301 6.1808 6.3316 6.4823 6.6331 6.7838 6.9346 7.0853 7.2361 7.3869 7.5376 7.6884 7.8391 7.9899 8.1406 8.2914 8.4421 8.5929 8.7436 8.8944 9.0451 9.1959 9.3466 9.4974 9.6481 9.7989 9.9496 10.1 10.251 10.402 10.553 10.703 10.854 11.005 11.156 11.306 11.457 11.608 11.759 11.909 12.06 12.211 12.362 12.512 12.663 12.814 12.965 13.115 13.266 13.417 13.568 13.718 13.869 14.02 14.171 14.321 14.472 14.623 14.774 14.924 15.075 15.226 15.377 15.527 15.678 15.829 15.98 16.13 16.281 16.432 16.583 16.733 16.884 17.035 17.186 17.336 17.487 17.638 17.789 17.939 18.09 18.241 18.392 18.543 18.693 18.844 18.995 19.146 19.296 19.447 19.598 19.749 19.899 20.05 20.201 20.352 20.502 20.653 20.804 20.955 21.105 21.256 21.407 21.558 21.708 21.859 22.01 22.161 22.311 22.462 22.613 22.764 22.914 23.065 23.216 23.367 23.517 23.668 23.819 23.97 24.12 24.271 24.422 24.573 24.723 24.874 25.025 25.176 25.326 25.477 25.628 25.779 25.929 26.08 26.231 26.382 26.532 26.683 26.834 26.985 27.135 27.286 27.437 27.588 27.738 27.889 28.04 28.191 28.341 28.492 28.643 28.794 28.944 29.095 29.246 29.397 29.547 29.698 29.849 30]
      | sbobj.Groups.Signals(6).YData = [0 0.0063472 0.013725 0.021607 0.029579 0.037322 0.044602 0.051251 0.057163 0.06228 0.066581 0.070078 0.072807 0.074819 0.076181 0.076964 0.077246 0.077103 0.076612 0.075845 0.074871 0.073751 0.072542 0.071292 0.070045 0.068835 0.067693 0.06664 0.065694 0.064866 0.064164 0.06359 0.063142 0.062816 0.062605 0.062498 0.062484 0.062552 0.062686 0.062875 0.063102 0.063355 0.06362 0.063885 0.064138 0.064368 0.064567 0.064726 0.064839 0.064901 0.064907 0.064856 0.064745 0.064576 0.064349 0.064066 0.063731 0.063347 0.062919 0.062452 0.061951 0.061423 0.060873 0.060307 0.059732 0.059153 0.058576 0.058006 0.057449 0.056909 0.05639 0.055895 0.055429 0.054992 0.054587 0.054215 0.053876 0.053572 0.0533 0.05306 0.05285 0.052669 0.052514 0.052382 0.052269 0.052173 0.05209 0.052015 0.051947 0.051879 0.05181 0.051734 0.051649 0.051551 0.051438 0.051306 0.051153 0.050977 0.050776 0.05055 0.050296 0.050015 0.049706 0.04937 0.049008 0.048621 0.04821 0.047777 0.047325 0.046855 0.04637 0.045874 0.045369 0.044858 0.044344 0.043831 0.043322 0.04282 0.042328 0.041849 0.041385 0.040939 0.040513 0.040109 0.039728 0.039371 0.03904 0.038734 0.038453 0.038197 0.037965 0.037755 0.037566 0.037396 0.037241 0.0371 0.036969 0.036845 0.036723 0.036602 0.036476 0.036341 0.036195 0.036034 0.035853 0.03565 0.035422 0.035166 0.034881 0.034563 0.034212 0.033828 0.03341 0.032959 0.032476 0.031962 0.031422 0.030856 0.03027 0.029668 0.029053 0.028432 0.027811 0.027194 0.026589 0.026001 0.025437 0.024902 0.024402 0.023943 0.023527 0.023159 0.022841 0.022573 0.022354 0.022184 0.022056 0.021965 0.021903 0.021858 0.021819 0.02177 0.021694 0.021574 0.021389 0.021119 0.02074 0.020232 0.019573 0.018744 0.017726 0.016506 0.015074 0.013425 0.011564 0.0095037 0.007268 0.0048968 0.0024476 -3.505e-15]
      | sbobj.Groups.TimeRange = [0 30]
  Subsystem : Subsystem
  Bus : Outport
  wires:
  FromWs/1 -> Subsystem/1(In1)
  Subsystem/1(Velocity Angular x) -> Bus Creator/1  "Velocity Angular x"
  Subsystem/2(Velocity Angular y) -> Bus Creator/2  "Velocity Angular y"
  Subsystem/3(Velocity Angular z) -> Bus Creator/3  "Velocity Angular z"
  Subsystem/4(Velocity Linear x) -> Bus Creator/4  "Velocity Linear x"
  Subsystem/5(Velocity Linear y) -> Bus Creator/5  "Velocity Linear y"
  Subsystem/6(Velocity Linear z) -> Bus Creator/6  "Velocity Linear z"
  Bus Creator/1 -> Bus/1

== system untitled/Signal Builder1 ==
  Bus Creator : BusCreator  Tag=Bus Creator  Inputs=6
  FromWs : FromWorkspace  Tag=STV FromWs  VariableName=tuvar  SampleTime=0
      SigBuilderData=|
      | common.afterFinalStr = 'Extrapolate'
      | common.sampleTime = 0
      | dataSet.timeRange = [0 30]
      | dataSet.name = 'Desired Velocities'
      | sbobj.Groups.Name = 'Desired Velocities'
      | sbobj.Groups.Signals(1).Name = 'Velocity Angular x'
      | sbobj.Groups.Signals(1).XData = [0 0.15075 0.3015 0.45226 0.60301 0.75376 0.90451 1.0553 1.206 1.3568 1.5075 1.6583 1.809 1.9598 2.1105 2.2613 2.412 2.5628 2.7135 2.8643 3.015 3.1658 3.3165 3.4673 3.618 3.7688 3.9196 4.0703 4.2211 4.3718 4.5226 4.6733 4.8241 4.9748 5.1256 5.2763 5.4271 5.5778 5.7286 5.8793 6.0301 6.1808 6.3316 6.4823 6.6331 6.7838 6.9346 7.0853 7.2361 7.3869 7.5376 7.6884 7.8391 7.9899 8.1406 8.2914 8.4421 8.5929 8.7436 8.8944 9.0451 9.1959 9.3466 9.4974 9.6481 9.7989 9.9496 10.1 10.251 10.402 10.553 10.703 10.854 11.005 11.156 11.306 11.457 11.608 11.759 11.909 12.06 12.211 12.362 12.512 12.663 12.814 12.965 13.115 13.266 13.417 13.568 13.718 13.869 14.02 14.171 14.321 14.472 14.623 14.774 14.924 15.075 15.226 15.377 15.527 15.678 15.829 15.98 16.13 16.281 16.432 16.583 16.733 16.884 17.035 17.186 17.336 17.487 17.638 17.789 17.939 18.09 18.241 18.392 18.543 18.693 18.844 18.995 19.146 19.296 19.447 19.598 19.749 19.899 20.05 20.201 20.352 20.502 20.653 20.804 20.955 21.105 21.256 21.407 21.558 21.708 21.859 22.01 22.161 22.311 22.462 22.613 22.764 22.914 23.065 23.216 23.367 23.517 23.668 23.819 23.97 24.12 24.271 24.422 24.573 24.723 24.874 25.025 25.176 25.326 25.477 25.628 25.779 25.929 26.08 26.231 26.382 26.532 26.683 26.834 26.985 27.135 27.286 27.437 27.588 27.738 27.889 28.04 28.191 28.341 28.492 28.643 28.794 28.944 29.095 29.246 29.397 29.547 29.698 29.849 30]
      | sbobj.Groups.Signals(1).YData = [0 -0.0018068 -0.0034031 -0.0047915 -0.0059792 -0.0069775 -0.0078002 -0.0084629 -0.0089823 -0.0093754 -0.0096591 -0.0098495 ... (200 elements, 1x200)]
      | sbobj.Groups.Signals(2).Name = 'Velocity Angular y'
      | sbobj.Groups.Signals(2).XData = [0 0.15075 0.3015 0.45226 0.60301 0.75376 0.90451 1.0553 1.206 1.3568 1.5075 1.6583 1.809 1.9598 2.1105 2.2613 2.412 2.5628 2.7135 2.8643 3.015 3.1658 3.3165 3.4673 3.618 3.7688 3.9196 4.0703 4.2211 4.3718 4.5226 4.6733 4.8241 4.9748 5.1256 5.2763 5.4271 5.5778 5.7286 5.8793 6.0301 6.1808 6.3316 6.4823 6.6331 6.7838 6.9346 7.0853 7.2361 7.3869 7.5376 7.6884 7.8391 7.9899 8.1406 8.2914 8.4421 8.5929 8.7436 8.8944 9.0451 9.1959 9.3466 9.4974 9.6481 9.7989 9.9496 10.1 10.251 10.402 10.553 10.703 10.854 11.005 11.156 11.306 11.457 11.608 11.759 11.909 12.06 12.211 12.362 12.512 12.663 12.814 12.965 13.115 13.266 13.417 13.568 13.718 13.869 14.02 14.171 14.321 14.472 14.623 14.774 14.924 15.075 15.226 15.377 15.527 15.678 15.829 15.98 16.13 16.281 16.432 16.583 16.733 16.884 17.035 17.186 17.336 17.487 17.638 17.789 17.939 18.09 18.241 18.392 18.543 18.693 18.844 18.995 19.146 19.296 19.447 19.598 19.749 19.899 20.05 20.201 20.352 20.502 20.653 20.804 20.955 21.105 21.256 21.407 21.558 21.708 21.859 22.01 22.161 22.311 22.462 22.613 22.764 22.914 23.065 23.216 23.367 23.517 23.668 23.819 23.97 24.12 24.271 24.422 24.573 24.723 24.874 25.025 25.176 25.326 25.477 25.628 25.779 25.929 26.08 26.231 26.382 26.532 26.683 26.834 26.985 27.135 27.286 27.437 27.588 27.738 27.889 28.04 28.191 28.341 28.492 28.643 28.794 28.944 29.095 29.246 29.397 29.547 29.698 29.849 30]
      | sbobj.Groups.Signals(2).YData = [0 -0.0022666 -0.0052246 -0.00859 -0.012137 -0.01569 -0.019115 -0.022315 -0.025222 -0.027794 -0.030007 -0.031856 -0.033348 -0.0345 -0.035335 -0.035883 -0.036178 -0.036253 -0.036144 -0.035884 -0.035509 -0.035047 -0.03453 -0.033981 -0.033425 -0.032881 -0.032366 -0.031893 -0.031474 -0.031115 -0.030823 -0.0306 -0.030446 -0.03036 -0.030339 -0.03038 -0.030476 -0.030621 -0.030809 -0.031031 -0.03128 -0.031549 -0.031829 -0.032114 -0.032396 -0.03267 -0.032929 -0.033168 -0.033383 -0.033571 -0.033727 -0.033851 -0.03394 -0.033995 -0.034015 -0.034001 -0.033954 -0.033876 -0.03377 -0.033638 -0.033484 -0.033311 -0.033123 -0.032923 -0.032715 -0.032504 -0.032292 -0.032084 -0.031883 -0.031691 -0.031513 -0.031351 -0.031207 -0.031082 -0.030979 -0.030899 -0.030841 -0.030808 -0.030797 -0.03081 -0.030845 -0.0309 -0.030975 -0.031068 -0.031176 -0.031297 -0.031429 -0.031568 -0.031714 -0.031861 -0.032009 -0.032154 -0.032293 -0.032425 -0.032546 -0.032654 -0.032747 -0.032824 -0.032884 -0.032924 -0.032945 -0.032945 -0.032924 -0.032883 -0.032822 -0.032742 -0.032644 -0.032528 -0.032398 -0.032254 -0.0321 -0.031936 -0.031767 -0.031593 -0.031419 -0.031246 -0.031078 -0.030917 -0.030765 -0.030626 -0.030501 -0.030393 -0.030302 -0.030232 -0.030182 -0.030155 -0.03015 -0.030167 -0.030207 -0.030268 -0.030351 -0.030452 -0.030571 -0.030705 -0.030852 -0.031009 -0.031172 -0.03134 -0.031507 -0.031672 -0.031829 -0.031975 -0.032108 -0.032222 -0.032316 -0.032386 -0.03243 -0.032445 -0.03243 -0.032383 -0.032304 -0.032194 -0.032052 -0.03188 -0.03168 -0.031456 -0.03121 -0.030948 -0.030673 -0.030391 -0.030109 -0.029833 -0.029569 -0.029325 -0.029107 -0.028922 -0.028776 -0.028675 -0.028625 -0.028629 -0.028689 -0.028808 -0.028985 -0.029218 -0.029501 -0.029828 -0.030189 -0.030572 -0.030961 -0.03134 -0.031686 -0.031977 -0.032187 -0.032287 -0.032248 -0.032039 -0.03163 -0.03099 -0.03009 -0.028908 -0.027423 -0.025625 -0.023511 -0.021094 -0.018401 -0.015482 -0.012411 -0.0092907 -0.0062639 -0.0035154]
      | sbobj.Groups.Signals(3).Name = 'Velocity Angular z'
      | sbobj.Groups.Signals(3).XData = [0 0.15075 0.3015 0.45226 0.60301 0.75376 0.90451 1.0553 1.206 1.3568 1.5075 1.6583 1.809 1.9598 2.1105 2.2613 2.412 2.5628 2.7135 2.8643 3.015 3.1658 3.3165 3.4673 3.618 3.7688 3.9196 4.0703 4.2211 4.3718 4.5226 4.6733 4.8241 4.9748 5.1256 5.2763 5.4271 5.5778 5.7286 5.8793 6.0301 6.1808 6.3316 6.4823 6.6331 6.7838 6.9346 7.0853 7.2361 7.3869 7.5376 7.6884 7.8391 7.9899 8.1406 8.2914 8.4421 8.5929 8.7436 8.8944 9.0451 9.1959 9.3466 9.4974 9.6481 9.7989 9.9496 10.1 10.251 10.402 10.553 10.703 10.854 11.005 11.156 11.306 11.457 11.608 11.759 11.909 12.06 12.211 12.362 12.512 12.663 12.814 12.965 13.115 13.266 13.417 13.568 13.718 13.869 14.02 14.171 14.321 14.472 14.623 14.774 14.924 15.075 15.226 15.377 15.527 15.678 15.829 15.98 16.13 16.281 16.432 16.583 16.733 16.884 17.035 17.186 17.336 17.487 17.638 17.789 17.939 18.09 18.241 18.392 18.543 18.693 18.844 18.995 19.146 19.296 19.447 19.598 19.749 19.899 20.05 20.201 20.352 20.502 20.653 20.804 20.955 21.105 21.256 21.407 21.558 21.708 21.859 22.01 22.161 22.311 22.462 22.613 22.764 22.914 23.065 23.216 23.367 23.517 23.668 23.819 23.97 24.12 24.271 24.422 24.573 24.723 24.874 25.025 25.176 25.326 25.477 25.628 25.779 25.929 26.08 26.231 26.382 26.532 26.683 26.834 26.985 27.135 27.286 27.437 27.588 27.738 27.889 28.04 28.191 28.341 28.492 28.643 28.794 28.944 29.095 29.246 29.397 29.547 29.698 29.849 30]
      | sbobj.Groups.Signals(3).YData = [0 0.00054192 0.00090485 0.0011364 0.0012753 0.0013522 0.0013906 0.0014082 0.0014177 0.0014277 0.0014432 0.0014672 0.0015001 0.0015414 0.0015895 0.001642 0.0016966 0.0017508 0.0018022 0.0018487 0.0018887 0.0019208 0.0019441 0.0019583 0.0019633 0.0019593 0.001947 0.0019273 0.0019012 0.0018699 0.0018349 0.0017974 0.0017589 0.0017206 0.0016839 0.00165 0.0016199 0.0015945 0.0015747 0.0015609 0.0015536 0.0015531 0.0015594 0.0015725 0.0015921 0.0016179 0.0016494 0.0016859 0.0017267 0.0017711 0.0018181 0.001867 0.0019168 0.0019667 0.0020158 0.0020633 0.0021083 0.0021503 0.0021887 0.0022228 0.0022524 0.002277 0.0022966 0.0023111 0.0023205 0.0023249 0.0023247 0.00232 0.0023115 0.0022996 0.0022848 0.0022678 0.0022493 0.0022298 0.0022102 0.0021911 0.0021732 0.0021571 0.0021435 0.0021328 0.0021257 0.0021224 0.0021234 0.002129 0.0021392 0.0021543 0.0021741 0.0021987 0.0022277 0.002261 0.0022981 0.0023387 0.0023823 0.0024282 0.0024759 0.0025248 0.0025741 0.0026231 0.0026711 0.0027175 0.0027615 0.0028026 0.0028401 0.0028734 0.0029022 0.002926 0.0029445 0.0029574 0.0029648 0.0029665 0.0029626 0.0029534 0.0029392 0.0029204 0.0028976 0.0028712 0.0028421 0.0028109 0.0027786 0.0027459 0.0027139 0.0026834 0.0026554 0.0026307 0.0026103 0.0025949 0.0025854 0.0025824 0.0025864 0.0025979 0.0026171 0.0026444 0.0026796 0.0027226 0.0027731 0.0028305 0.0028943 0.0029636 0.0030374 0.0031146 0.0031939 0.003274 0.0033534 0.0034307 0.0035042 0.0035724 0.0036338 0.003687 0.0037306 0.0037634 0.0037843 0.0037926 0.0037877 0.0037693 0.0037375 0.0036926 0.0036354 0.0035669 0.0034886 0.0034024 0.0033103 0.003215 0.0031191 0.0030257 0.002938 0.0028593 0.0027928 0.0027418 0.0027093 0.002698 0.0027102 0.0027474 0.0028108 0.0029002 0.0030149 0.0031528 0.0033106 0.0034836 0.0036659 0.0038501 0.0040275 0.004188 0.0043207 0.0044139 0.0044556 0.0044343 0.0043395 0.004163 0.0038999 0.0035504 0.0031216 0.0026293 0.0021014 0.0015799 0.0011252 0.00081917 0.00077016 0.0011172 0.0020355 0.0037422]
      | sbobj.Groups.Signals(4).Name = 'Velocity Linear x'
      | sbobj.Groups.Signals(4).XData = [0 0.15075 0.3015 0.45226 0.60301 0.75376 0.90451 1.0553 1.206 1.3568 1.5075 1.6583 1.809 1.9598 2.1105 2.2613 2.412 2.5628 2.7135 2.8643 3.015 3.1658 3.3165 3.4673 3.618 3.7688 3.9196 4.0703 4.2211 4.3718 4.5226 4.6733 4.8241 4.9748 5.1256 5.2763 5.4271 5.5778 5.7286 5.8793 6.0301 6.1808 6.3316 6.4823 6.6331 6.7838 6.9346 7.0853 7.2361 7.3869 7.5376 7.6884 7.8391 7.9899 8.1406 8.2914 8.4421 8.5929 8.7436 8.8944 9.0451 9.1959 9.3466 9.4974 9.6481 9.7989 9.9496 10.1 10.251 10.402 10.553 10.703 10.854 11.005 11.156 11.306 11.457 11.608 11.759 11.909 12.06 12.211 12.362 12.512 12.663 12.814 12.965 13.115 13.266 13.417 13.568 13.718 13.869 14.02 14.171 14.321 14.472 14.623 14.774 14.924 15.075 15.226 15.377 15.527 15.678 15.829 15.98 16.13 16.281 16.432 16.583 16.733 16.884 17.035 17.186 17.336 17.487 17.638 17.789 17.939 18.09 18.241 18.392 18.543 18.693 18.844 18.995 19.146 19.296 19.447 19.598 19.749 19.899 20.05 20.201 20.352 20.502 20.653 20.804 20.955 21.105 21.256 21.407 21.558 21.708 21.859 22.01 22.161 22.311 22.462 22.613 22.764 22.914 23.065 23.216 23.367 23.517 23.668 23.819 23.97 24.12 24.271 24.422 24.573 24.723 24.874 25.025 25.176 25.326 25.477 25.628 25.779 25.929 26.08 26.231 26.382 26.532 26.683 26.834 26.985 27.135 27.286 27.437 27.588 27.738 27.889 28.04 28.191 28.341 28.492 28.643 28.794 28.944 29.095 29.246 29.397 29.547 29.698 29.849 30]
      | sbobj.Groups.Signals(4).YData = [0 -0.0006469 -0.0019071 -0.0035651 -0.0054557 -0.0074534 -0.0094641 -0.011418 -0.013264 -0.014968 -0.016506 -0.017863 -0.019035 -0.020023 -0.020833 -0.021476 -0.021966 -0.02232 -0.022557 -0.022697 -0.022759 -0.022763 -0.022728 -0.022671 -0.022609 -0.022555 -0.022522 -0.022521 -0.022558 -0.02264 -0.022772 -0.022955 -0.023189 -0.023475 -0.023809 -0.024188 -0.024608 -0.025064 -0.02555 -0.026061 -0.026589 -0.02713 -0.027676 -0.028222 -0.028762 -0.029291 -0.029804 -0.030297 -0.030766 -0.031209 -0.031623 -0.032005 -0.032356 -0.032674 -0.03296 -0.033215 -0.03344 -0.033636 -0.033807 -0.033954 -0.034082 -0.034192 -0.034289 -0.034376 -0.034457 -0.034536 -0.034615 -0.034699 -0.034791 -0.034894 -0.03501 -0.035143 -0.035293 -0.035464 -0.035655 -0.035868 -0.036104 -0.036362 -0.036642 -0.036943 -0.037265 -0.037606 -0.037963 -0.038336 -0.038721 -0.039117 -0.03952 -0.039927 -0.040337 -0.040745 -0.04115 -0.041547 -0.041935 -0.042311 -0.042672 -0.043016 -0.043342 -0.043646 -0.043929 -0.044189 -0.044425 -0.044637 -0.044825 -0.044989 -0.04513 -0.045249 -0.045347 -0.045426 -0.045488 -0.045535 -0.045571 -0.045597 -0.045616 -0.045632 -0.045648 -0.045666 -0.04569 -0.045723 -0.045767 -0.045826 -0.045901 -0.045996 -0.046112 -0.04625 -0.046413 -0.0466 -0.046812 -0.04705 -0.047312 -0.047598 -0.047906 -0.048235 -0.048583 -0.048946 -0.049321 -0.049706 -0.050096 -0.050487 -0.050876 -0.051258 -0.051628 -0.051983 -0.052317 -0.052628 -0.05291 -0.053161 -0.053377 -0.053556 -0.053695 -0.053793 -0.053849 -0.053863 -0.053836 -0.053769 -0.053666 -0.053528 -0.053361 -0.05317 -0.052961 -0.05274 -0.052515 -0.052294 -0.052085 -0.051898 -0.05174 -0.051621 -0.051549 -0.051533 -0.051579 -0.051693 -0.051881 -0.052144 -0.052484 -0.0529 -0.053387 -0.053937 -0.054541 -0.055183 -0.055845 -0.056505 -0.057135 -0.057702 -0.058171 -0.0585 -0.058641 -0.058545 -0.058156 -0.057415 -0.05626 -0.054628 -0.052453 -0.049672 -0.046224 -0.042053 -0.037109 -0.031354 -0.024763 -0.017327 -0.0090607 9.2466e-16]
      | sbobj.Groups.Signals(5).Name = 'Velocity Linear y'
      | sbobj.Groups.Signals(5).XData = [0 0.15075 0.3015 0.45226 0.60301 0.75376 0.90451 1.0553 1.206 1.3568 1.5075 1.6583 1.809 1.9598 2.1105 2.2613 2.412 2.5628 2.7135 2.8643 3.015 3.1658 3.3165 3.4673 3.618 3.7688 3.9196 4.0703 4.2211 4.3718 4.5226 4.6733 4.8241 4.9748 5.1256 5.2763 5.4271 5.5778 5.7286 5.8793 6.0301 6.1808 6.3316 6.4823 6.6331 6.7838 6.9346 7.0853 7.2361 7.3869 7.5376 7.6884 7.8391 7.9899 8.1406 8.2914 8.4421 8.5929 8.7436 8.8944 9.0451 9.1959 9.3466 9.4974 9.6481 9.7989 9.9496 10.1 10.251 10.402 10.553 10.703 10.854 11.005 11.156 11.306 11.457 11.608 11.759 11.909 12.06 12.211 12.362 12.512 12.663 12.814 12.965 13.115 13.266 13.417 13.568 13.718 13.869 14.02 14.171 14.321 14.472 14.623 14.774 14.924 15.075 15.226 15.377 15.527 15.678 15.829 15.98 16.13 16.281 16.432 16.583 16.733 16.884 17.035 17.186 17.336 17.487 17.638 17.789 17.939 18.09 18.241 18.392 18.543 18.693 18.844 18.995 19.146 19.296 19.447 19.598 19.749 19.899 20.05 20.201 20.352 20.502 20.653 20.804 20.955 21.105 21.256 21.407 21.558 21.708 21.859 22.01 22.161 22.311 22.462 22.613 22.764 22.914 23.065 23.216 23.367 23.517 23.668 23.819 23.97 24.12 24.271 24.422 24.573 24.723 24.874 25.025 25.176 25.326 25.477 25.628 25.779 25.929 26.08 26.231 26.382 26.532 26.683 26.834 26.985 27.135 27.286 27.437 27.588 27.738 27.889 28.04 28.191 28.341 28.492 28.643 28.794 28.944 29.095 29.246 29.397 29.547 29.698 29.849 30]
      | sbobj.Groups.Signals(5).YData = [0 0.0019316 0.0034825 0.0047149 0.0056861 0.0064464 0.0070393 0.007501 0.0078612 0.0081436 0.0083667 0.0085448 0.0086886 0.008806 0.0089029 0.0089833 0.0090503 0.009106 0.0091518 0.009189 0.0092184 0.0092408 0.0092568 0.0092671 0.0092721 0.0092726 0.0092691 0.0092623 0.0092527 0.009241 0.009228 0.0092142 0.0092004 0.0091874 0.0091758 0.0091665 0.0091601 0.0091573 0.009159 0.0091657 0.0091781 0.0091968 0.0092222 0.0092549 0.009295 0.0093429 0.0093987 0.0094623 0.0095338 0.0096129 0.0096992 0.0097925 0.0098921 0.0099974 0.010108 0.010223 0.010341 0.010462 0.010585 0.010708 0.010832 0.010954 0.011075 0.011193 0.011307 0.011417 0.011522 0.011621 0.011714 0.011799 0.011878 0.011949 0.012012 0.012067 0.012114 0.012153 0.012184 0.012207 0.012223 0.012232 0.012235 0.012233 0.012225 0.012213 0.012197 0.012179 0.012159 0.012138 0.012117 0.012098 0.012081 0.012066 0.012056 0.012051 0.012051 0.012058 0.012073 0.012095 0.012125 0.012165 0.012214 0.012273 0.012341 0.012419 0.012506 0.012603 0.012709 0.012823 0.012946 0.013075 0.013211 0.013353 0.013499 0.013649 0.013802 0.013955 0.014109 0.014261 0.01441 0.014556 0.014697 0.014832 0.014959 0.015077 0.015186 0.015285 0.015372 0.015448 0.015511 0.015561 0.015598 0.015622 0.015633 0.015632 0.015619 0.015594 0.015559 0.015514 0.015461 0.015402 0.015337 0.015269 0.015199 0.015129 0.015062 0.014999 0.014943 0.014895 0.014858 0.014834 0.014825 0.014833 0.01486 0.014906 0.014974 0.015065 0.015179 0.015317 0.01548 0.015667 0.015877 0.01611 0.016365 0.01664 0.016933 0.017241 0.017561 0.017891 0.018227 0.018564 0.018899 0.019228 0.019544 0.019845 0.020125 0.020378 0.0206 0.020786 0.02093 0.021027 0.021072 0.021059 0.020983 0.020838 0.020618 0.020316 0.019926 0.019438 0.018845 0.018135 0.017296 0.016314 0.01517 0.013843 0.012306 0.010527 0.0084644 0.0060676 0.0032728 -5.8634e-16]
      | sbobj.Groups.Signals(6).Name = 'Velocity Linear z'
      | sbobj.Groups.Signals(6).XData = [0 0.15075 0.3015 0.45226 0.60301 0.75376 0.90451 1.0553 1.206 1.3568 1.5075 1.6583 1.809 1.9598 2.1105 2.2613 2.412 2.5628 2.7135 2.8643 3.015 3.1658 3.3165 3.4673 3.618 3.7688 3.9196 4.0703 4.2211 4.3718 4.5226 4.6733 4.8241 4.9748 5.1256 5.2763 5.4271 5.5778 5.7286 5.8793 6.0301 6.1808 6.3316 6.4823 6.6331 6.7838 6.9346 7.0853 7.2361 7.3869 7.5376 7.6884 7.8391 7.9899 8.1406 8.2914 8.4421 8.5929 8.7436 8.8944 9.0451 9.1959 9.3466 9.4974 9.6481 9.7989 9.9496 10.1 10.251 10.402 10.553 10.703 10.854 11.005 11.156 11.306 11.457 11.608 11.759 11.909 12.06 12.211 12.362 12.512 12.663 12.814 12.965 13.115 13.266 13.417 13.568 13.718 13.869 14.02 14.171 14.321 14.472 14.623 14.774 14.924 15.075 15.226 15.377 15.527 15.678 15.829 15.98 16.13 16.281 16.432 16.583 16.733 16.884 17.035 17.186 17.336 17.487 17.638 17.789 17.939 18.09 18.241 18.392 18.543 18.693 18.844 18.995 19.146 19.296 19.447 19.598 19.749 19.899 20.05 20.201 20.352 20.502 20.653 20.804 20.955 21.105 21.256 21.407 21.558 21.708 21.859 22.01 22.161 22.311 22.462 22.613 22.764 22.914 23.065 23.216 23.367 23.517 23.668 23.819 23.97 24.12 24.271 24.422 24.573 24.723 24.874 25.025 25.176 25.326 25.477 25.628 25.779 25.929 26.08 26.231 26.382 26.532 26.683 26.834 26.985 27.135 27.286 27.437 27.588 27.738 27.889 28.04 28.191 28.341 28.492 28.643 28.794 28.944 29.095 29.246 29.397 29.547 29.698 29.849 30]
      | sbobj.Groups.Signals(6).YData = [0 0.0063472 0.013725 0.021607 0.029579 0.037322 0.044602 0.051251 0.057163 0.06228 0.066581 0.070078 0.072807 0.074819 0.076181 0.076964 0.077246 0.077103 0.076612 0.075845 0.074871 0.073751 0.072542 0.071292 0.070045 0.068835 0.067693 0.06664 0.065694 0.064866 0.064164 0.06359 0.063142 0.062816 0.062605 0.062498 0.062484 0.062552 0.062686 0.062875 0.063102 0.063355 0.06362 0.063885 0.064138 0.064368 0.064567 0.064726 0.064839 0.064901 0.064907 0.064856 0.064745 0.064576 0.064349 0.064066 0.063731 0.063347 0.062919 0.062452 0.061951 0.061423 0.060873 0.060307 0.059732 0.059153 0.058576 0.058006 0.057449 0.056909 0.05639 0.055895 0.055429 0.054992 0.054587 0.054215 0.053876 0.053572 0.0533 0.05306 0.05285 0.052669 0.052514 0.052382 0.052269 0.052173 0.05209 0.052015 0.051947 0.051879 0.05181 0.051734 0.051649 0.051551 0.051438 0.051306 0.051153 0.050977 0.050776 0.05055 0.050296 0.050015 0.049706 0.04937 0.049008 0.048621 0.04821 0.047777 0.047325 0.046855 0.04637 0.045874 0.045369 0.044858 0.044344 0.043831 0.043322 0.04282 0.042328 0.041849 0.041385 0.040939 0.040513 0.040109 0.039728 0.039371 0.03904 0.038734 0.038453 0.038197 0.037965 0.037755 0.037566 0.037396 0.037241 0.0371 0.036969 0.036845 0.036723 0.036602 0.036476 0.036341 0.036195 0.036034 0.035853 0.03565 0.035422 0.035166 0.034881 0.034563 0.034212 0.033828 0.03341 0.032959 0.032476 0.031962 0.031422 0.030856 0.03027 0.029668 0.029053 0.028432 0.027811 0.027194 0.026589 0.026001 0.025437 0.024902 0.024402 0.023943 0.023527 0.023159 0.022841 0.022573 0.022354 0.022184 0.022056 0.021965 0.021903 0.021858 0.021819 0.02177 0.021694 0.021574 0.021389 0.021119 0.02074 0.020232 0.019573 0.018744 0.017726 0.016506 0.015074 0.013425 0.011564 0.0095037 0.007268 0.0048968 0.0024476 -3.505e-15]
      | sbobj.Groups.TimeRange = [0 30]
  Subsystem : Subsystem
  Bus : Outport
  wires:
  Bus Creator/1 -> Bus/1
  Subsystem/6(Velocity Linear z) -> Bus Creator/6  "Velocity Linear z"
  Subsystem/5(Velocity Linear y) -> Bus Creator/5  "Velocity Linear y"
  Subsystem/4(Velocity Linear x) -> Bus Creator/4  "Velocity Linear x"
  Subsystem/3(Velocity Angular z) -> Bus Creator/3  "Velocity Angular z"
  Subsystem/2(Velocity Angular y) -> Bus Creator/2  "Velocity Angular y"
  Subsystem/1(Velocity Angular x) -> Bus Creator/1  "Velocity Angular x"
  FromWs/1 -> Subsystem/1(In1)

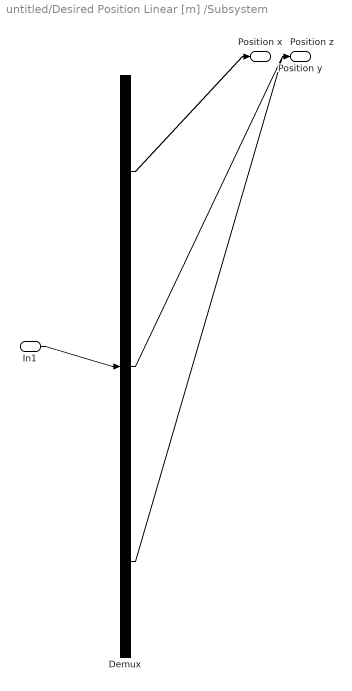
== system untitled/Desired Position Linear [m] /Subsystem ==
  In1 : Inport
  Demux : Demux  Tag=STV Demux  Outputs=3
  Position x : Outport  Tag=STV Outport
  Position y : Outport  Tag=STV Outport  Port=2
  Position z : Outport  Tag=STV Outport  Port=3
  wires:
  In1/1 -> Demux/1
  Demux/1 -> Position x/1
  Demux/2 -> Position y/1
  Demux/3 -> Position z/1

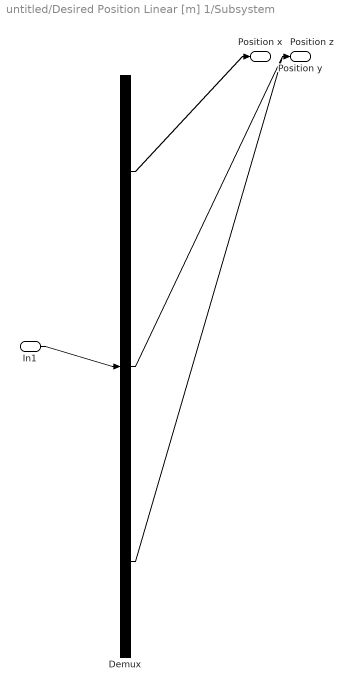
== system untitled/Desired Position Linear [m] 1/Subsystem ==
  In1 : Inport
  Demux : Demux  Tag=STV Demux  Outputs=3
  Position x : Outport  Tag=STV Outport
  Position y : Outport  Tag=STV Outport  Port=2
  Position z : Outport  Tag=STV Outport  Port=3
  wires:
  In1/1 -> Demux/1
  Demux/1 -> Position x/1
  Demux/2 -> Position y/1
  Demux/3 -> Position z/1

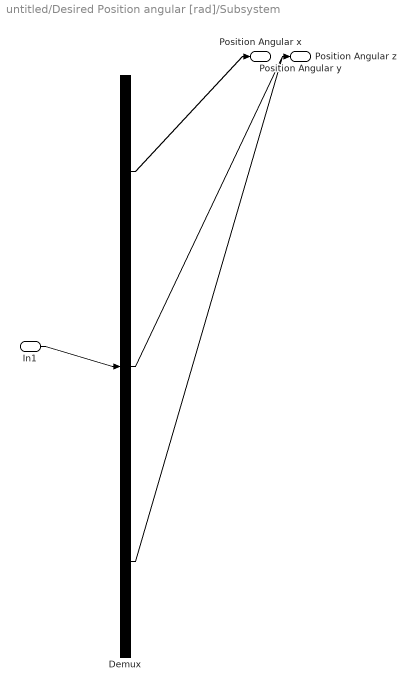
== system untitled/Desired Position angular [rad]/Subsystem ==
  In1 : Inport
  Demux : Demux  Tag=STV Demux  Outputs=3
  Position Angular x : Outport  Tag=STV Outport
  Position Angular y : Outport  Tag=STV Outport  Port=2
  Position Angular z : Outport  Tag=STV Outport  Port=3
  wires:
  In1/1 -> Demux/1
  Demux/3 -> Position Angular z/1
  Demux/2 -> Position Angular y/1
  Demux/1 -> Position Angular x/1

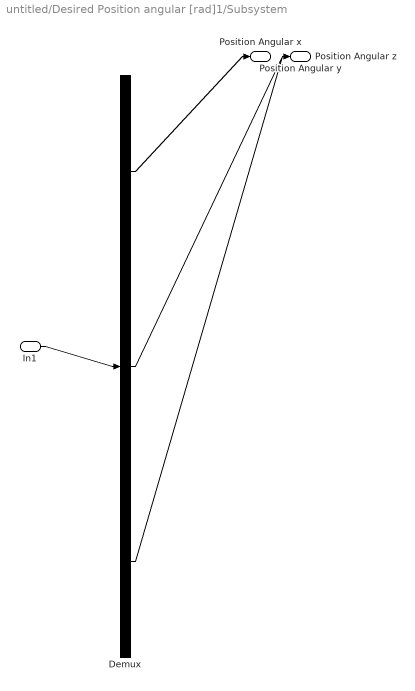
== system untitled/Desired Position angular [rad]1/Subsystem ==
  In1 : Inport
  Demux : Demux  Tag=STV Demux  Outputs=3
  Position Angular x : Outport  Tag=STV Outport
  Position Angular y : Outport  Tag=STV Outport  Port=2
  Position Angular z : Outport  Tag=STV Outport  Port=3
  wires:
  In1/1 -> Demux/1
  Demux/3 -> Position Angular z/1
  Demux/2 -> Position Angular y/1
  Demux/1 -> Position Angular x/1

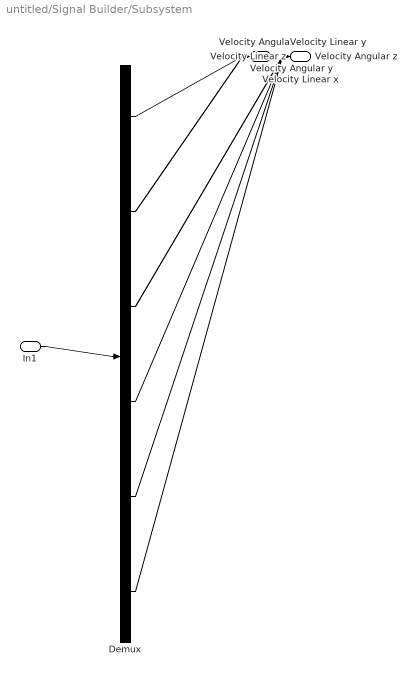
== system untitled/Signal Builder/Subsystem ==
  In1 : Inport
  Demux : Demux  Tag=STV Demux  Outputs=6
  Velocity Angular x : Outport  Tag=STV Outport
  Velocity Angular y : Outport  Tag=STV Outport  Port=2
  Velocity Angular z : Outport  Tag=STV Outport  Port=3
  Velocity Linear x : Outport  Tag=STV Outport  Port=4
  Velocity Linear y : Outport  Tag=STV Outport  Port=5
  Velocity Linear z : Outport  Tag=STV Outport  Port=6
  wires:
  Demux/1 -> Velocity Angular x/1
  Demux/2 -> Velocity Angular y/1
  Demux/3 -> Velocity Angular z/1
  Demux/4 -> Velocity Linear x/1
  Demux/5 -> Velocity Linear y/1
  Demux/6 -> Velocity Linear z/1
  In1/1 -> Demux/1

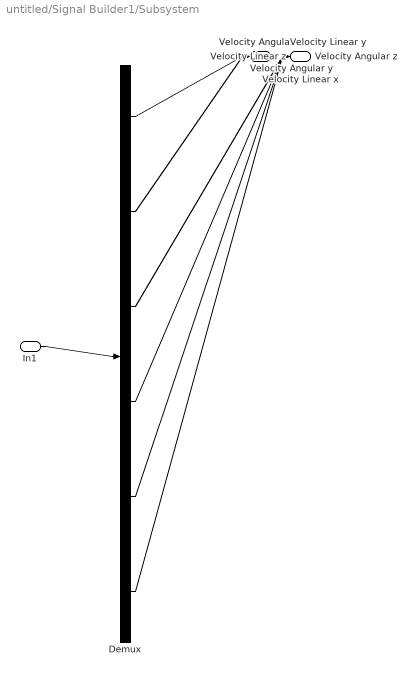
== system untitled/Signal Builder1/Subsystem ==
  In1 : Inport
  Demux : Demux  Tag=STV Demux  Outputs=6
  Velocity Angular x : Outport  Tag=STV Outport
  Velocity Angular y : Outport  Tag=STV Outport  Port=2
  Velocity Angular z : Outport  Tag=STV Outport  Port=3
  Velocity Linear x : Outport  Tag=STV Outport  Port=4
  Velocity Linear y : Outport  Tag=STV Outport  Port=5
  Velocity Linear z : Outport  Tag=STV Outport  Port=6
  wires:
  In1/1 -> Demux/1
  Demux/6 -> Velocity Linear z/1
  Demux/5 -> Velocity Linear y/1
  Demux/4 -> Velocity Linear x/1
  Demux/3 -> Velocity Angular z/1
  Demux/2 -> Velocity Angular y/1
  Demux/1 -> Velocity Angular x/1

== matlab function untitled/CHASER/robotForwardDynamics  ==
  data: tau0 input; base_acc output; taum input; wF0 input; wFm input; t0 input; tL input; P0 input; pm input; I0 input; Im input; Bij input; Bi0 input; u0 input; um input; qdotdot_joints output; robot parameter
function [base_acc, qdotdot_joints]= robotForwardDyn(tau0,taum, wF0,wFm,t0,tL,P0,pm,I0,Im,Bij,Bi0,u0,um, robot)

[base_acc, qdotdot_joints] = FD(tau0,taum,wF0,wFm,t0,tL,P0,pm,I0,Im,Bij,Bi0,u0,um,robot);

end

== matlab function untitled/CHASER/CalculateJacobianAndInertias ==
  data: RL output; rL output; base_pose input; J0_0ee output; q_joints input; Jman_0ee output; H0 output; H0m output; Hm output; Cm output; t0 output; tL output; P0 output; pm output; I0 output; Im output; Bij output; Bi0 output; robot parameter; u0 input; um input
function [RL, rL, J0_0ee, Jman_0ee, H0, H0m, Hm, Cm, t0, tL, P0, pm, I0, Im, Bij, Bi0]   ...
    = jacobianAndInertiaMatrices(base_pose, q_joints, robot, u0, um)

r0 = base_pose(4:6,:);
R0 = eul2rotm((base_pose(1:3,:))', 'ZYX');
%% kinematic (to return jacobian)
[RJ,RL,rJ,rL,e,g]=Kinematics(R0,r0,q_joints,robot);
%Diferential Kinematics
[Bij,Bi0,P0,pm]=DiffKinematics(R0,r0,rL,e,g,robot);
%Velocities
[t0,tL]=Velocities(Bij,Bi0,P0,pm,u0,um,robot);
%Jacobian of the last link (the end effector)
[J0_0ee, Jman_0ee]=Jacob(rL(1:3,end),r0,rL,P0,pm,robot.n_links_joints,robot);

%% dynamic 
% (to return generalized inertia matrix and Convective Inertia Matrix

%Inertias projected in the inertial frame
[I0,Im]=I_I(R0,RL,robot);
%Mass Composite Body matrix
[M0_tilde,Mm_tilde]=MCB(I0,Im,Bij,Bi0,robot);
%Generalized Inertia Matrix
[H0, H0m, Hm] = GIM(M0_tilde,Mm_tilde,Bij,Bi0,P0,pm,robot);
%Generalized Convective Inertia Matrix
[C0, C0m, Cm0, Cm] = CIM(t0,tL,I0,Im,M0_tilde,Mm_tilde,Bij,Bi0,P0,pm,robot);





end

== matlab function untitled/CHASER/rot matrix to euler  ==
  data: rotm input; eul output
function eul = rotm2eulcolumnvect(rotm)

eulrow = rotm2eul(rotm, 'ZYX');
eul = eulrow';
end

== matlab function untitled/CHASER1/CalculateJacobianAndInertias ==
  data: RL output; rL output; base_pose input; J0_0ee output; q_joints input; Jman_0ee output; H0 output; H0m output; Hm output; Cm output; t0 output; tL output; P0 output; pm output; I0 output; Im output; Bij output; Bi0 output; robot parameter; u0 input; um input
function [RL, rL, J0_0ee, Jman_0ee, H0, H0m, Hm, Cm, t0, tL, P0, pm, I0, Im, Bij, Bi0]   ...
    = jacobianAndInertiaMatrices(base_pose, q_joints, robot, u0, um)

r0 = base_pose(4:6,:);
R0 = eul2rotm((base_pose(1:3,:))', 'ZYX');
%% kinematic (to return jacobian)
[RJ,RL,rJ,rL,e,g]=Kinematics(R0,r0,q_joints,robot);
%Diferential Kinematics
[Bij,Bi0,P0,pm]=DiffKinematics(R0,r0,rL,e,g,robot);
%Velocities
[t0,tL]=Velocities(Bij,Bi0,P0,pm,u0,um,robot);
%Jacobian of the last link (the end effector)
[J0_0ee, Jman_0ee]=Jacob(rL(1:3,end),r0,rL,P0,pm,robot.n_links_joints,robot);

%% dynamic 
% (to return generalized inertia matrix and Convective Inertia Matrix

%Inertias projected in the inertial frame
[I0,Im]=I_I(R0,RL,robot);
%Mass Composite Body matrix
[M0_tilde,Mm_tilde]=MCB(I0,Im,Bij,Bi0,robot);
%Generalized Inertia Matrix
[H0, H0m, Hm] = GIM(M0_tilde,Mm_tilde,Bij,Bi0,P0,pm,robot);
%Generalized Convective Inertia Matrix
[C0, C0m, Cm0, Cm] = CIM(t0,tL,I0,Im,M0_tilde,Mm_tilde,Bij,Bi0,P0,pm,robot);





end

== matlab function untitled/CHASER1/robotForwardDynamics  ==
  data: tau0 input; base_acc output; taum input; wF0 input; wFm input; t0 input; tL input; P0 input; pm input; I0 input; Im input; Bij input; Bi0 input; u0 input; um input; qdotdot_joints output; robot parameter
function [base_acc, qdotdot_joints]= robotForwardDyn(tau0,taum, wF0,wFm,t0,tL,P0,pm,I0,Im,Bij,Bi0,u0,um, robot)

[base_acc, qdotdot_joints] = FD(tau0,taum,wF0,wFm,t0,tL,P0,pm,I0,Im,Bij,Bi0,u0,um,robot);

end

== matlab function untitled/CHASER1/rot matrix to euler  ==
  data: rotm input; eul output
function eul = rotm2eulcolumnvect(rotm)

eulrow = rotm2eul(rotm, 'ZYX');
eul = eulrow';
end

== matlab function untitled/Cartesian Error ==
  data: ang1 input; diffAng output; lin1 input; ang2 input; lin2 input; diffLin output
function [diffAng, diffLin] = angLinError(ang1, lin1, ang2, lin2)

T1 = eye(4,4);
T2 = eye(4,4);

T1(1:3,1:3) = eul2rotm(ang1', 'ZYX');
T2(1:3,1:3) = eul2rotm(ang2', 'ZYX');

T1(1:3, 4) = lin1;
T2(1:3, 4) = lin2;

[diffAng, diffLin] = CartError(T1, T2);
end

== matlab function untitled/Cartesian Error1 ==
  data: ang1 input; diffAng output; lin1 input; ang2 input; lin2 input; diffLin output
function [diffAng, diffLin] = angLinError(ang1, lin1, ang2, lin2)

T1 = eye(4,4);
T2 = eye(4,4);

T1(1:3,1:3) = eul2rotm(ang1', 'ZYX');
T2(1:3,1:3) = eul2rotm(ang2', 'ZYX');

T1(1:3, 4) = lin1;
T2(1:3, 4) = lin2;

[diffAng, diffLin] = CartError(T1, T2);
end
